simulink model "kinovaMicoSimscapeModel"  (R2021b)
(part 41 of 50)

Y5_10_1=(111*dq4*dqr1*sin(q2)*sin(q3)*sin(q6))/4000 - (37*dq6*dqr1*sin(q2)*sin(q3)*sin(q6))/4000 - (111*dq4*dqr1*cos(q5)^2*sin(q2)*sin(q3)*sin(q6))/2000 - (111*dq6*dqr1*cos(q5)*sin(q2)*sin(q3)*sin(q6))/4000 - (37*dq2*dqr1*cos(q3)*cos(q4)^2*cos(q6)*sin(q2))/2000 + (37*dq3*dqr1*cos(q3)*cos(q4)^2*cos(q6)*sin(q2))/2000 + (37*3^(1/2)*dq1*dqr1*cos(q2)*sin(q2)*sin(q4)*sin(q6))/2000 - (37*3^(1/2)*dq2*dqr1*cos(q4)*sin(q2)*sin(q3)*sin(q6))/4000 + (37*3^(1/2)*dq3*dqr1*cos(q4)*sin(q2)*sin(q3)*sin(q6))/4000 - (37*3^(1/2)*dq4*dqr1*cos(q3)*sin(q2)*sin(q4)*sin(q6))/4000 - (37*3^(1/2)*dq6*dqr1*cos(q3)*sin(q2)*sin(q4)*sin(q6))/4000 + (37*dq2*dqr1*cos(q3)*cos(q4)^2*cos(q5)^2*cos(q6)*sin(q2))/1000 - (37*dq3*dqr1*cos(q3)*cos(q4)^2*cos(q5)^2*cos(q6)*sin(q2))/1000 + (37*dq1*dqr1*cos(q2)*cos(q3)*sin(q2)*sin(q3)*sin(q6))/1000 - (877*dq1*dqr1*cos(q2)*cos(q4)*sin(q2)*sin(q5)*sin(q6))/4000 - (1231*dq1*dqr1*cos(q2)*cos(q6)*sin(q2)*sin(q4)*sin(q5))/40000 + (37*dq2*dqr1*cos(q3)*cos(q4)*sin(q2)*sin(q4)*sin(q6))/800 + (877*dq2*dqr1*cos(q4)*cos(q5)*sin(q2)*sin(q3)*sin(q6))/8000 - (37*dq3*dqr1*cos(q3)*cos(q4)*sin(q2)*sin(q4)*sin(q6))/800 + (37*dq2*dqr1*cos(q3)*cos(q5)*sin(q2)*sin(q5)*sin(q6))/1000 - (877*dq3*dqr1*cos(q4)*cos(q5)*sin(q2)*sin(q3)*sin(q6))/8000 - (37*dq3*dqr1*cos(q3)*cos(q5)*sin(q2)*sin(q5)*sin(q6))/1000 - (111*dq4*dqr1*cos(q5)*cos(q6)*sin(q2)*sin(q3)*sin(q5))/4000 - (877*dq2*dqr1*sin(q2)*sin(q3)*sin(q4)*sin(q5)*sin(q6))/4000 + (877*dq3*dqr1*sin(q2)*sin(q3)*sin(q4)*sin(q5)*sin(q6))/4000 - dq2*dqr1*cos(q3)*sin(q2)*sin(q5)*sin(q6)*((641*3^(1/2))/20000 + 37/1000) + dq3*dqr1*cos(q3)*sin(q2)*sin(q5)*sin(q6)*((641*3^(1/2))/20000 + 37/1000) - dq4*dqr1*cos(q5)*sin(q2)*sin(q3)*sin(q6)*((641*3^(1/2))/40000 + 37/2000) - dq4*dqr1*cos(q6)*sin(q2)*sin(q3)*sin(q5)*((641*3^(1/2))/80000 - 37/8000) - (37*3^(1/2)*dq1*dqr1*cos(q2)*cos(q4)*cos(q6)*sin(q2))/2000 + (37*3^(1/2)*dq1*dqr1*cos(q2)*cos(q3)^2*cos(q4)*cos(q6)*sin(q2))/1000 + (37*3^(1/2)*dq1*dqr1*cos(q2)*cos(q4)*cos(q5)^2*cos(q6)*sin(q2))/1000 - (37*3^(1/2)*dq4*dqr1*cos(q3)*cos(q4)*cos(q5)^2*cos(q6)*sin(q2))/2000 + (29*dq1*dqr1*cos(q2)*cos(q3)*cos(q4)*cos(q5)*cos(q6)*sin(q2))/200 - (37*3^(1/2)*dq1*dqr1*cos(q2)*cos(q3)^2*sin(q2)*sin(q4)*sin(q6))/1000 - (37*3^(1/2)*dq1*dqr1*cos(q2)*cos(q5)^2*sin(q2)*sin(q4)*sin(q6))/1000 + (37*3^(1/2)*dq2*dqr1*cos(q4)*cos(q5)^2*sin(q2)*sin(q3)*sin(q6))/2000 + (37*3^(1/2)*dq2*dqr1*cos(q5)^2*cos(q6)*sin(q2)*sin(q3)*sin(q4))/2000 - (37*3^(1/2)*dq3*dqr1*cos(q4)*cos(q5)^2*sin(q2)*sin(q3)*sin(q6))/2000 - (37*3^(1/2)*dq3*dqr1*cos(q5)^2*cos(q6)*sin(q2)*sin(q3)*sin(q4))/2000 + (37*3^(1/2)*dq4*dqr1*cos(q3)*cos(q5)^2*sin(q2)*sin(q4)*sin(q6))/2000 - (29*dq1*dqr1*cos(q2)*cos(q3)*cos(q4)*sin(q2)*sin(q5)*sin(q6))/100 - (29*dq1*dqr1*cos(q2)*cos(q3)*cos(q5)*sin(q2)*sin(q4)*sin(q6))/200 - (29*dq1*dqr1*cos(q2)*cos(q3)*cos(q6)*sin(q2)*sin(q4)*sin(q5))/400 - dq1*dqr1*cos(q2)*cos(q4)*cos(q5)*cos(q6)*sin(q2)*((37*3^(1/2))/4000 - 877/8000) - dq2*dqr1*cos(q5)*cos(q6)*sin(q2)*sin(q3)*sin(q4)*((37*3^(1/2))/4000 - 877/8000) + dq3*dqr1*cos(q5)*cos(q6)*sin(q2)*sin(q3)*sin(q4)*((37*3^(1/2))/4000 - 877/8000) + dq1*dqr1*cos(q2)*cos(q5)*sin(q2)*sin(q4)*sin(q6)*((37*3^(1/2))/2000 - 1231/20000) - dq2*dqr1*cos(q4)*cos(q6)*sin(q2)*sin(q3)*sin(q5)*((37*3^(1/2))/8000 - 877/16000) + dq3*dqr1*cos(q4)*cos(q6)*sin(q2)*sin(q3)*sin(q5)*((37*3^(1/2))/8000 - 877/16000) - dq4*dqr1*cos(q3)*cos(q5)*sin(q2)*sin(q4)*sin(q6)*((37*3^(1/2))/2000 + 1923/40000) + dq4*dqr1*cos(q3)*cos(q6)*sin(q2)*sin(q4)*sin(q5)*((37*3^(1/2))/8000 - 1923/80000) + (37*dq1*dqr1*cos(q2)*cos(q3)*cos(q4)^2*sin(q2)*sin(q3)*sin(q6))/400 - (37*dq1*dqr1*cos(q2)*cos(q3)*cos(q5)^2*sin(q2)*sin(q3)*sin(q6))/500 + (877*dq1*dqr1*cos(q2)*cos(q3)^2*cos(q4)*sin(q2)*sin(q5)*sin(q6))/2000 + (1231*dq1*dqr1*cos(q2)*cos(q3)^2*cos(q6)*sin(q2)*sin(q4)*sin(q5))/20000 - (37*dq2*dqr1*cos(q3)*cos(q4)*cos(q5)^2*sin(q2)*sin(q4)*sin(q6))/400 - (37*dq2*dqr1*cos(q3)*cos(q4)^2*cos(q5)*sin(q2)*sin(q5)*sin(q6))/500 + (37*dq3*dqr1*cos(q3)*cos(q4)*cos(q5)^2*sin(q2)*sin(q4)*sin(q6))/400 + (37*dq3*dqr1*cos(q3)*cos(q4)^2*cos(q5)*sin(q2)*sin(q5)*sin(q6))/500 - dq2*dqr1*cos(q3)*cos(q4)^2*cos(q5)*cos(q6)*sin(q2)*((641*3^(1/2))/40000 - 37/4000) + dq3*dqr1*cos(q3)*cos(q4)^2*cos(q5)*cos(q6)*sin(q2)*((641*3^(1/2))/40000 - 37/4000) + (29*3^(1/2)*dq1*dqr1*cos(q2)*cos(q5)*sin(q2)*sin(q3)*sin(q6))/200 + (29*3^(1/2)*dq1*dqr1*cos(q2)*cos(q6)*sin(q2)*sin(q3)*sin(q5))/400 + (37*3^(1/2)*dq6*dqr1*cos(q3)*cos(q4)*sin(q2)*sin(q5)*sin(q6))/2000 + (37*3^(1/2)*dq6*dqr1*cos(q3)*cos(q5)*sin(q2)*sin(q4)*sin(q6))/4000 + dq2*dqr1*cos(q3)*cos(q4)^2*sin(q2)*sin(q5)*sin(q6)*((641*3^(1/2))/20000 + 37/1000) - dq3*dqr1*cos(q3)*cos(q4)^2*sin(q2)*sin(q5)*sin(q6)*((641*3^(1/2))/20000 + 37/1000) + (37*dq1*dqr1*cos(q2)*cos(q3)*cos(q4)*cos(q6)*sin(q2)*sin(q3)*sin(q4))/1000 - (37*dq1*dqr1*cos(q2)*cos(q3)*cos(q5)*cos(q6)*sin(q2)*sin(q3)*sin(q5))/1000 - (37*dq2*dqr1*cos(q3)*cos(q4)*cos(q5)*cos(q6)*sin(q2)*sin(q4)*sin(q5))/800 + (37*dq3*dqr1*cos(q3)*cos(q4)*cos(q5)*cos(q6)*sin(q2)*sin(q4)*sin(q5))/800 - (37*3^(1/2)*dq1*dqr1*cos(q2)*cos(q3)^2*cos(q4)*cos(q5)^2*cos(q6)*sin(q2))/500 - dq1*dqr1*cos(q2)*cos(q3)*cos(q5)*sin(q2)*sin(q3)*sin(q6)*((2513*3^(1/2))/10000 + 37/1000) - dq1*dqr1*cos(q2)*cos(q3)*cos(q6)*sin(q2)*sin(q3)*sin(q5)*((2513*3^(1/2))/20000 - 37/1000) + dq2*dqr1*cos(q3)*cos(q4)*cos(q5)*sin(q2)*sin(q4)*sin(q6)*((641*3^(1/2))/40000 + 37/2000) - dq3*dqr1*cos(q3)*cos(q4)*cos(q5)*sin(q2)*sin(q4)*sin(q6)*((641*3^(1/2))/40000 + 37/2000) + dq2*dqr1*cos(q3)*cos(q4)*cos(q6)*sin(q2)*sin(q4)*sin(q5)*((641*3^(1/2))/80000 - 37/8000) - dq3*dqr1*cos(q3)*cos(q4)*cos(q6)*sin(q2)*sin(q4)*sin(q5)*((641*3^(1/2))/80000 - 37/8000) + (37*3^(1/2)*dq1*dqr1*cos(q2)*cos(q3)^2*cos(q5)^2*sin(q2)*sin(q4)*sin(q6))/500 + dq1*dqr1*cos(q2)*cos(q3)^2*cos(q4)*cos(q5)*cos(q6)*sin(q2)*((37*3^(1/2))/2000 - 877/4000) - (37*3^(1/2)*dq1*dqr1*cos(q2)*cos(q4)*cos(q5)*sin(q2)*sin(q5)*sin(q6))/500 - (37*3^(1/2)*dq1*dqr1*cos(q2)*cos(q5)*cos(q6)*sin(q2)*sin(q4)*sin(q5))/2000 + (37*3^(1/2)*dq2*dqr1*cos(q4)*cos(q5)*cos(q6)*sin(q2)*sin(q3)*sin(q5))/4000 - (37*3^(1/2)*dq3*dqr1*cos(q4)*cos(q5)*cos(q6)*sin(q2)*sin(q3)*sin(q5))/4000 + (37*3^(1/2)*dq4*dqr1*cos(q3)*cos(q4)*cos(q5)*sin(q2)*sin(q5)*sin(q6))/1000 + (37*3^(1/2)*dq4*dqr1*cos(q3)*cos(q5)*cos(q6)*sin(q2)*sin(q4)*sin(q5))/4000 - dq1*dqr1*cos(q2)*cos(q3)^2*cos(q5)*sin(q2)*sin(q4)*sin(q6)*((37*3^(1/2))/1000 - 1231/10000) - (37*3^(1/2)*dq2*dqr1*cos(q5)*sin(q2)*sin(q3)*sin(q4)*sin(q5)*sin(q6))/1000 + (37*3^(1/2)*dq3*dqr1*cos(q5)*sin(q2)*sin(q3)*sin(q4)*sin(q5)*sin(q6))/1000 - (37*dq1*dqr1*cos(q2)*cos(q3)*cos(q4)^2*cos(q5)^2*sin(q2)*sin(q3)*sin(q6))/200 - (37*dq1*dqr1*cos(q2)*cos(q3)*cos(q4)*cos(q5)^2*cos(q6)*sin(q2)*sin(q3)*sin(q4))/500 - (37*dq1*dqr1*cos(q2)*cos(q3)*cos(q4)^2*cos(q5)*cos(q6)*sin(q2)*sin(q3)*sin(q5))/400 + dq1*dqr1*cos(q2)*cos(q3)*cos(q4)^2*cos(q5)*sin(q2)*sin(q3)*sin(q6)*((641*3^(1/2))/20000 + 37/1000) + dq1*dqr1*cos(q2)*cos(q3)*cos(q4)^2*cos(q6)*sin(q2)*sin(q3)*sin(q5)*((641*3^(1/2))/40000 - 37/4000) + (37*3^(1/2)*dq1*dqr1*cos(q2)*cos(q3)^2*cos(q4)*cos(q5)*sin(q2)*sin(q5)*sin(q6))/250 + (37*3^(1/2)*dq1*dqr1*cos(q2)*cos(q3)^2*cos(q5)*cos(q6)*sin(q2)*sin(q4)*sin(q5))/1000 + dq1*dqr1*cos(q2)*cos(q3)*cos(q4)*cos(q5)*cos(q6)*sin(q2)*sin(q3)*sin(q4)*((641*3^(1/2))/20000 - 37/2000) - dq1*dqr1*cos(q2)*cos(q3)*cos(q4)*sin(q2)*sin(q3)*sin(q4)*sin(q5)*sin(q6)*((641*3^(1/2))/10000 + 37/500) + (37*dq1*dqr1*cos(q2)*cos(q3)*cos(q4)*cos(q5)*sin(q2)*sin(q3)*sin(q4)*sin(q5)*sin(q6))/250;
Y5_10_2=(7*dq1*dqr1*cos(q5)*cos(q6)*sin(q4))/2000 - (7*dq1*dqr1*sin(q4)*sin(q5)*sin(q6))/1000 + (29*dq1*dqr1*cos(q4)*cos(q5)*cos(q6)*sin(q3))/200 - (29*dq2*dqr1*cos(q2)*cos(q5)*cos(q6)*sin(q4))/200 - (29*dq1*dqr1*cos(q4)*sin(q3)*sin(q5)*sin(q6))/100 - (29*dq1*dqr1*cos(q5)*sin(q3)*sin(q4)*sin(q6))/200 - (29*dq1*dqr1*cos(q6)*sin(q3)*sin(q4)*sin(q5))/400 + (29*dq2*dqr1*cos(q2)*sin(q4)*sin(q5)*sin(q6))/100 - (37*dq1*dqr1*cos(q2)^2*cos(q4)*cos(q6)*sin(q4))/2000 + (37*dq2*dqr1*cos(q2)*cos(q4)^2*cos(q6)*sin(q3))/2000 - (37*dq1*dqr1*cos(q3)^2*cos(q4)*cos(q6)*sin(q4))/2000 + (37*dq2*dqr1*cos(q2)*cos(q5)^2*cos(q6)*sin(q3))/2000 - (37*dq2*dqr1*cos(q3)*cos(q5)^2*cos(q6)*sin(q2))/2000 - (37*dq3*dqr1*cos(q2)*cos(q4)^2*cos(q6)*sin(q3))/2000 - (37*dq3*dqr1*cos(q2)*cos(q5)^2*cos(q6)*sin(q3))/2000 + (37*dq3*dqr1*cos(q3)*cos(q5)^2*cos(q6)*sin(q2))/2000 - (37*3^(1/2)*dq1*dqr1*cos(q3)*sin(q3)*sin(q4)*sin(q6))/2000 + (37*3^(1/2)*dq4*dqr1*cos(q2)*sin(q3)*sin(q4)*sin(q6))/4000 + (37*3^(1/2)*dq6*dqr1*cos(q2)*sin(q3)*sin(q4)*sin(q6))/4000 + (37*dq1*dqr1*cos(q2)^2*cos(q3)^2*cos(q4)*cos(q6)*sin(q4))/1000 + (37*dq1*dqr1*cos(q2)^2*cos(q4)*cos(q5)^2*cos(q6)*sin(q4))/1000 - (37*dq2*dqr1*cos(q2)*cos(q4)^2*cos(q5)^2*cos(q6)*sin(q3))/1000 + (37*dq1*dqr1*cos(q3)^2*cos(q4)*cos(q5)^2*cos(q6)*sin(q4))/1000 + (37*dq3*dqr1*cos(q2)*cos(q4)^2*cos(q5)^2*cos(q6)*sin(q3))/1000 - (37*dq2*dqr1*cos(q2)*cos(q4)*sin(q3)*sin(q4)*sin(q6))/800 + (877*dq1*dqr1*cos(q3)*cos(q4)*sin(q3)*sin(q5)*sin(q6))/4000 + (1231*dq1*dqr1*cos(q3)*cos(q6)*sin(q3)*sin(q4)*sin(q5))/40000 - (877*dq2*dqr1*cos(q2)*cos(q3)*sin(q4)*sin(q5)*sin(q6))/4000 + (37*dq3*dqr1*cos(q2)*cos(q4)*sin(q3)*sin(q4)*sin(q6))/800 - (37*dq2*dqr1*cos(q2)*cos(q5)*sin(q3)*sin(q5)*sin(q6))/1000 + (877*dq3*dqr1*cos(q2)*cos(q3)*sin(q4)*sin(q5)*sin(q6))/4000 + (37*dq3*dqr1*cos(q2)*cos(q5)*sin(q3)*sin(q5)*sin(q6))/1000 - dq2*dqr1*cos(q2)*cos(q5)*cos(q6)*sin(q3)*((641*3^(1/2))/40000 - 37/4000) + dq2*dqr1*cos(q3)*cos(q5)*cos(q6)*sin(q2)*((641*3^(1/2))/40000 - 37/4000) + dq3*dqr1*cos(q2)*cos(q5)*cos(q6)*sin(q3)*((641*3^(1/2))/40000 - 37/4000) - dq3*dqr1*cos(q3)*cos(q5)*cos(q6)*sin(q2)*((641*3^(1/2))/40000 - 37/4000) - (29*dq1*dqr1*cos(q2)^2*cos(q4)*cos(q5)*cos(q6)*sin(q3))/200 + dq2*dqr1*cos(q2)*sin(q3)*sin(q5)*sin(q6)*((641*3^(1/2))/20000 + 37/1000) - dq3*dqr1*cos(q2)*sin(q3)*sin(q5)*sin(q6)*((641*3^(1/2))/20000 + 37/1000) + (29*dq1*dqr1*cos(q2)^2*cos(q4)*sin(q3)*sin(q5)*sin(q6))/100 + (29*dq1*dqr1*cos(q2)^2*cos(q5)*sin(q3)*sin(q4)*sin(q6))/200 + (29*dq1*dqr1*cos(q2)^2*cos(q6)*sin(q3)*sin(q4)*sin(q5))/400 + (37*3^(1/2)*dq1*dqr1*cos(q3)*cos(q4)*cos(q6)*sin(q3))/2000 - (37*3^(1/2)*dq4*dqr1*cos(q2)*cos(q4)*cos(q6)*sin(q3))/2000 + (37*3^(1/2)*dq4*dqr1*cos(q3)*cos(q4)*cos(q6)*sin(q2))/2000 - (37*3^(1/2)*dq1*dqr1*cos(q2)^2*cos(q3)*cos(q4)*cos(q6)*sin(q3))/1000 - (37*3^(1/2)*dq1*dqr1*cos(q3)*cos(q4)*cos(q5)^2*cos(q6)*sin(q3))/1000 + (37*3^(1/2)*dq2*dqr1*cos(q2)*cos(q3)*cos(q5)^2*cos(q6)*sin(q4))/2000 - (37*3^(1/2)*dq3*dqr1*cos(q2)*cos(q3)*cos(q5)^2*cos(q6)*sin(q4))/2000 + (37*3^(1/2)*dq4*dqr1*cos(q2)*cos(q4)*cos(q5)^2*cos(q6)*sin(q3))/2000 + (37*3^(1/2)*dq1*dqr1*cos(q2)^2*cos(q3)*sin(q3)*sin(q4)*sin(q6))/1000 + (37*3^(1/2)*dq1*dqr1*cos(q3)*cos(q5)^2*sin(q3)*sin(q4)*sin(q6))/1000 - (37*3^(1/2)*dq4*dqr1*cos(q2)*cos(q5)^2*sin(q3)*sin(q4)*sin(q6))/2000 - (37*dq1*dqr1*cos(q2)^2*cos(q3)^2*cos(q4)*cos(q5)^2*cos(q6)*sin(q4))/500 - (37*dq1*dqr1*cos(q2)^2*cos(q3)^2*cos(q4)^2*cos(q5)*cos(q6)*sin(q5))/400 + dq1*dqr1*cos(q3)*cos(q4)*cos(q5)*cos(q6)*sin(q3)*((37*3^(1/2))/4000 - 877/8000) - dq2*dqr1*cos(q2)*cos(q3)*cos(q5)*cos(q6)*sin(q4)*((37*3^(1/2))/4000 - 877/8000) + dq3*dqr1*cos(q2)*cos(q3)*cos(q5)*cos(q6)*sin(q4)*((37*3^(1/2))/4000 - 877/8000) - dq1*dqr1*cos(q3)*cos(q5)*sin(q3)*sin(q4)*sin(q6)*((37*3^(1/2))/2000 - 1231/20000) + dq4*dqr1*cos(q2)*cos(q5)*sin(q3)*sin(q4)*sin(q6)*((37*3^(1/2))/2000 + 1923/40000) - dq4*dqr1*cos(q2)*cos(q6)*sin(q3)*sin(q4)*sin(q5)*((37*3^(1/2))/8000 - 1923/80000) - (877*dq1*dqr1*cos(q2)^2*cos(q3)*cos(q4)*sin(q3)*sin(q5)*sin(q6))/2000 - (1231*dq1*dqr1*cos(q2)^2*cos(q3)*cos(q6)*sin(q3)*sin(q4)*sin(q5))/20000 + (37*dq2*dqr1*cos(q2)*cos(q4)*cos(q5)^2*sin(q3)*sin(q4)*sin(q6))/400 - (37*dq1*dqr1*cos(q2)^2*cos(q4)*cos(q5)*sin(q4)*sin(q5)*sin(q6))/500 + (37*dq2*dqr1*cos(q2)*cos(q4)^2*cos(q5)*sin(q3)*sin(q5)*sin(q6))/500 - (37*dq3*dqr1*cos(q2)*cos(q4)*cos(q5)^2*sin(q3)*sin(q4)*sin(q6))/400 - (37*dq1*dqr1*cos(q3)^2*cos(q4)*cos(q5)*sin(q4)*sin(q5)*sin(q6))/500 - (37*dq3*dqr1*cos(q2)*cos(q4)^2*cos(q5)*sin(q3)*sin(q5)*sin(q6))/500 - dq1*dqr1*cos(q2)^2*cos(q4)*cos(q5)*cos(q6)*sin(q4)*((641*3^(1/2))/40000 - 37/4000) + dq2*dqr1*cos(q2)*cos(q4)^2*cos(q5)*cos(q6)*sin(q3)*((641*3^(1/2))/40000 - 37/4000) - dq1*dqr1*cos(q3)^2*cos(q4)*cos(q5)*cos(q6)*sin(q4)*((641*3^(1/2))/40000 - 37/4000) - dq3*dqr1*cos(q2)*cos(q4)^2*cos(q5)*cos(q6)*sin(q3)*((641*3^(1/2))/40000 - 37/4000) - (37*3^(1/2)*dq6*dqr1*cos(q2)*cos(q4)*sin(q3)*sin(q5)*sin(q6))/2000 - (37*3^(1/2)*dq6*dqr1*cos(q2)*cos(q5)*sin(q3)*sin(q4)*sin(q6))/4000 + dq1*dqr1*cos(q2)^2*cos(q4)*sin(q4)*sin(q5)*sin(q6)*((641*3^(1/2))/20000 + 37/1000) - dq2*dqr1*cos(q2)*cos(q4)^2*sin(q3)*sin(q5)*sin(q6)*((641*3^(1/2))/20000 + 37/1000) + dq1*dqr1*cos(q3)^2*cos(q4)*sin(q4)*sin(q5)*sin(q6)*((641*3^(1/2))/20000 + 37/1000) + dq3*dqr1*cos(q2)*cos(q4)^2*sin(q3)*sin(q5)*sin(q6)*((641*3^(1/2))/20000 + 37/1000) + dq1*dqr1*cos(q2)^2*cos(q3)^2*cos(q4)*cos(q5)*cos(q6)*sin(q4)*((641*3^(1/2))/20000 - 37/2000) + (37*dq2*dqr1*cos(q2)*cos(q4)*cos(q5)*cos(q6)*sin(q3)*sin(q4)*sin(q5))/800 - (37*dq3*dqr1*cos(q2)*cos(q4)*cos(q5)*cos(q6)*sin(q3)*sin(q4)*sin(q5))/800 - dq1*dqr1*cos(q2)^2*cos(q3)^2*cos(q4)*sin(q4)*sin(q5)*sin(q6)*((641*3^(1/2))/10000 + 37/500) + (37*3^(1/2)*dq1*dqr1*cos(q2)^2*cos(q3)*cos(q4)*cos(q5)^2*cos(q6)*sin(q3))/500 - dq2*dqr1*cos(q2)*cos(q4)*cos(q5)*sin(q3)*sin(q4)*sin(q6)*((641*3^(1/2))/40000 + 37/2000) + dq3*dqr1*cos(q2)*cos(q4)*cos(q5)*sin(q3)*sin(q4)*sin(q6)*((641*3^(1/2))/40000 + 37/2000) - dq2*dqr1*cos(q2)*cos(q4)*cos(q6)*sin(q3)*sin(q4)*sin(q5)*((641*3^(1/2))/80000 - 37/8000) + dq3*dqr1*cos(q2)*cos(q4)*cos(q6)*sin(q3)*sin(q4)*sin(q5)*((641*3^(1/2))/80000 - 37/8000) - (37*3^(1/2)*dq1*dqr1*cos(q2)^2*cos(q3)*cos(q5)^2*sin(q3)*sin(q4)*sin(q6))/500 - dq1*dqr1*cos(q2)^2*cos(q3)*cos(q4)*cos(q5)*cos(q6)*sin(q3)*((37*3^(1/2))/2000 - 877/4000) + (37*3^(1/2)*dq1*dqr1*cos(q3)*cos(q4)*cos(q5)*sin(q3)*sin(q5)*sin(q6))/500 + (37*3^(1/2)*dq1*dqr1*cos(q3)*cos(q5)*cos(q6)*sin(q3)*sin(q4)*sin(q5))/2000 - (37*3^(1/2)*dq2*dqr1*cos(q2)*cos(q3)*cos(q5)*sin(q4)*sin(q5)*sin(q6))/1000 + (37*3^(1/2)*dq3*dqr1*cos(q2)*cos(q3)*cos(q5)*sin(q4)*sin(q5)*sin(q6))/1000 - (37*3^(1/2)*dq4*dqr1*cos(q2)*cos(q4)*cos(q5)*sin(q3)*sin(q5)*sin(q6))/1000 - (37*3^(1/2)*dq4*dqr1*cos(q2)*cos(q5)*cos(q6)*sin(q3)*sin(q4)*sin(q5))/4000 + dq1*dqr1*cos(q2)^2*cos(q3)*cos(q5)*sin(q3)*sin(q4)*sin(q6)*((37*3^(1/2))/1000 - 1231/10000) + (37*dq1*dqr1*cos(q2)^2*cos(q3)^2*cos(q4)*cos(q5)*sin(q4)*sin(q5)*sin(q6))/250 - (37*3^(1/2)*dq1*dqr1*cos(q2)^2*cos(q3)*cos(q4)*cos(q5)*sin(q3)*sin(q5)*sin(q6))/250 - (37*3^(1/2)*dq1*dqr1*cos(q2)^2*cos(q3)*cos(q5)*cos(q6)*sin(q3)*sin(q4)*sin(q5))/1000;
Y5_10_3=(111*dq1*dqr1*sin(q6))/4000 - (37*dq1*dqr1*cos(q2)^2*sin(q6))/2000 - (37*dq1*dqr1*cos(q3)^2*sin(q6))/2000 - (111*dq1*dqr1*cos(q5)^2*sin(q6))/2000 + (37*dq1*dqr1*cos(q2)^2*cos(q3)^2*sin(q6))/1000 - (37*dq1*dqr1*cos(q2)^2*cos(q4)^2*sin(q6))/800 + (37*dq1*dqr1*cos(q2)^2*cos(q5)^2*sin(q6))/1000 - (37*dq1*dqr1*cos(q3)^2*cos(q4)^2*sin(q6))/800 + (37*dq1*dqr1*cos(q3)^2*cos(q5)^2*sin(q6))/1000 + (111*dq4*dqr1*cos(q2)*cos(q3)*sin(q6))/4000 + (7*dq1*dqr1*cos(q4)*cos(q5)*sin(q6))/2000 + (7*dq1*dqr1*cos(q4)*cos(q6)*sin(q5))/4000 - (111*dq1*dqr1*cos(q5)*cos(q6)*sin(q5))/4000 - (37*dq6*dqr1*cos(q2)*cos(q3)*sin(q6))/4000 - dq1*dqr1*cos(q5)*sin(q6)*((641*3^(1/2))/40000 + 37/2000) - dq1*dqr1*cos(q6)*sin(q5)*((641*3^(1/2))/80000 - 37/8000) - (29*3^(1/2)*dq1*dqr1*cos(q3)*cos(q5)*sin(q6))/200 - (29*3^(1/2)*dq1*dqr1*cos(q3)*cos(q6)*sin(q5))/400 + dq1*dqr1*cos(q2)^2*cos(q5)*sin(q6)*((2513*3^(1/2))/20000 + 37/2000) + dq1*dqr1*cos(q3)^2*cos(q5)*sin(q6)*((2513*3^(1/2))/20000 + 37/2000) + dq1*dqr1*cos(q2)^2*cos(q6)*sin(q5)*((2513*3^(1/2))/40000 - 37/2000) + dq1*dqr1*cos(q3)^2*cos(q6)*sin(q5)*((2513*3^(1/2))/40000 - 37/2000) - (29*dq2*dqr1*cos(q2)*cos(q4)*cos(q5)*sin(q6))/200 - (29*dq2*dqr1*cos(q2)*cos(q4)*cos(q6)*sin(q5))/400 + (29*dq2*dqr2*cos(q4)*cos(q5)*cos(q6)*sin(q3))/200 - (111*dq6*dqr1*cos(q2)*cos(q3)*cos(q5)*sin(q6))/4000 + (37*dq1*dqr1*cos(q2)^2*cos(q3)^2*cos(q4)^2*sin(q6))/400 - (37*dq1*dqr1*cos(q2)^2*cos(q3)^2*cos(q5)^2*sin(q6))/500 + (37*dq1*dqr1*cos(q2)^2*cos(q4)^2*cos(q5)^2*sin(q6))/400 + (37*dq1*dqr1*cos(q3)^2*cos(q4)^2*cos(q5)^2*sin(q6))/400 - (29*dq2*dqr2*cos(q4)*sin(q3)*sin(q5)*sin(q6))/100 - (29*dq2*dqr2*cos(q5)*sin(q3)*sin(q4)*sin(q6))/200 - (29*dq2*dqr2*cos(q6)*sin(q3)*sin(q4)*sin(q5))/400 + (37*dq1*dqr2*cos(q2)*cos(q4)^2*cos(q6)*sin(q3))/2000 - (37*dq1*dqr2*cos(q3)*cos(q4)^2*cos(q6)*sin(q2))/2000 + (37*dq1*dqr2*cos(q2)*cos(q5)^2*cos(q6)*sin(q3))/2000 - (37*dq1*dqr2*cos(q3)*cos(q5)^2*cos(q6)*sin(q2))/2000 + (37*dq1*dqr1*cos(q2)^2*cos(q5)*cos(q6)*sin(q5))/2000 + (37*dq1*dqr1*cos(q3)^2*cos(q5)*cos(q6)*sin(q5))/2000 - (111*dq4*dqr1*cos(q2)*cos(q3)*cos(q5)^2*sin(q6))/2000 - (37*3^(1/2)*dq1*dqr2*cos(q4)*sin(q2)*sin(q3)*sin(q6))/4000 - (37*dq1*dqr1*cos(q2)^2*cos(q3)^2*cos(q5)*cos(q6)*sin(q5))/1000 - (37*dq1*dqr2*cos(q2)*cos(q4)^2*cos(q5)^2*cos(q6)*sin(q3))/1000 + (37*dq1*dqr2*cos(q3)*cos(q4)^2*cos(q5)^2*cos(q6)*sin(q2))/1000 + (37*dq1*dqr1*cos(q2)^2*cos(q4)^2*cos(q5)*cos(q6)*sin(q5))/800 + (37*dq1*dqr1*cos(q3)^2*cos(q4)^2*cos(q5)*cos(q6)*sin(q5))/800 + (29*3^(1/2)*dq1*dqr1*cos(q2)^2*cos(q3)*cos(q5)*sin(q6))/200 + (29*3^(1/2)*dq1*dqr1*cos(q2)^2*cos(q3)*cos(q6)*sin(q5))/400 + (877*dq2*dqr1*cos(q2)*cos(q3)*cos(q4)*cos(q5)*sin(q6))/8000 - (877*dq3*dqr1*cos(q2)*cos(q3)*cos(q4)*cos(q5)*sin(q6))/8000 - (111*dq4*dqr1*cos(q2)*cos(q3)*cos(q5)*cos(q6)*sin(q5))/4000 - dq1*dqr1*cos(q2)^2*cos(q3)^2*cos(q5)*sin(q6)*((2513*3^(1/2))/10000 + 37/1000) - dq1*dqr1*cos(q2)^2*cos(q3)^2*cos(q6)*sin(q5)*((2513*3^(1/2))/20000 - 37/1000) - dq1*dqr1*cos(q2)^2*cos(q4)^2*cos(q5)*sin(q6)*((641*3^(1/2))/40000 + 37/2000) - dq1*dqr1*cos(q3)^2*cos(q4)^2*cos(q5)*sin(q6)*((641*3^(1/2))/40000 + 37/2000) - dq1*dqr1*cos(q2)^2*cos(q4)^2*cos(q6)*sin(q5)*((641*3^(1/2))/80000 - 37/8000) - dq1*dqr1*cos(q3)^2*cos(q4)^2*cos(q6)*sin(q5)*((641*3^(1/2))/80000 - 37/8000) - (37*dq1*dqr2*cos(q2)*cos(q4)*sin(q3)*sin(q4)*sin(q6))/800 + (37*dq1*dqr2*cos(q3)*cos(q4)*sin(q2)*sin(q4)*sin(q6))/800 + (877*dq1*dqr2*cos(q4)*cos(q5)*sin(q2)*sin(q3)*sin(q6))/8000 - (37*dq1*dqr2*cos(q2)*cos(q5)*sin(q3)*sin(q5)*sin(q6))/1000 + (37*dq1*dqr2*cos(q3)*cos(q5)*sin(q2)*sin(q5)*sin(q6))/1000 - (877*dq1*dqr2*sin(q2)*sin(q3)*sin(q4)*sin(q5)*sin(q6))/4000 - dq4*dqr1*cos(q2)*cos(q3)*cos(q5)*sin(q6)*((641*3^(1/2))/40000 + 37/2000) - dq1*dqr2*cos(q2)*cos(q5)*cos(q6)*sin(q3)*((641*3^(1/2))/40000 - 37/4000) + dq1*dqr2*cos(q3)*cos(q5)*cos(q6)*sin(q2)*((641*3^(1/2))/40000 - 37/4000) - dq4*dqr1*cos(q2)*cos(q3)*cos(q6)*sin(q5)*((641*3^(1/2))/80000 - 37/8000) + dq1*dqr2*cos(q2)*sin(q3)*sin(q5)*sin(q6)*((641*3^(1/2))/20000 + 37/1000) - dq1*dqr2*cos(q3)*sin(q2)*sin(q5)*sin(q6)*((641*3^(1/2))/20000 + 37/1000) - (37*dq1*dqr1*cos(q2)^2*cos(q3)^2*cos(q4)^2*cos(q5)^2*sin(q6))/200 - (37*3^(1/2)*dq2*dqr1*cos(q2)*cos(q3)*cos(q4)*sin(q6))/4000 + (37*3^(1/2)*dq3*dqr1*cos(q2)*cos(q3)*cos(q4)*sin(q6))/4000 + (37*3^(1/2)*dq2*dqr1*cos(q2)*cos(q3)*cos(q4)*cos(q5)^2*sin(q6))/2000 - (37*3^(1/2)*dq3*dqr1*cos(q2)*cos(q3)*cos(q4)*cos(q5)^2*sin(q6))/2000 + (37*3^(1/2)*dq1*dqr2*cos(q4)*cos(q5)^2*sin(q2)*sin(q3)*sin(q6))/2000 + (37*3^(1/2)*dq1*dqr2*cos(q5)^2*cos(q6)*sin(q2)*sin(q3)*sin(q4))/2000 - dq2*dqr1*cos(q2)*cos(q3)*cos(q4)*cos(q6)*sin(q5)*((37*3^(1/2))/8000 - 877/16000) + dq3*dqr1*cos(q2)*cos(q3)*cos(q4)*cos(q6)*sin(q5)*((37*3^(1/2))/8000 - 877/16000) + dq1*dqr1*cos(q2)^2*cos(q3)^2*cos(q4)^2*cos(q5)*sin(q6)*((641*3^(1/2))/20000 + 37/1000) + dq1*dqr1*cos(q2)^2*cos(q3)^2*cos(q4)^2*cos(q6)*sin(q5)*((641*3^(1/2))/40000 - 37/4000) - dq1*dqr2*cos(q5)*cos(q6)*sin(q2)*sin(q3)*sin(q4)*((37*3^(1/2))/4000 - 877/8000) - dq1*dqr2*cos(q4)*cos(q6)*sin(q2)*sin(q3)*sin(q5)*((37*3^(1/2))/8000 - 877/16000) + (37*dq1*dqr2*cos(q2)*cos(q4)*cos(q5)^2*sin(q3)*sin(q4)*sin(q6))/400 - (37*dq1*dqr2*cos(q3)*cos(q4)*cos(q5)^2*sin(q2)*sin(q4)*sin(q6))/400 + (37*dq1*dqr2*cos(q2)*cos(q4)^2*cos(q5)*sin(q3)*sin(q5)*sin(q6))/500 - (37*dq1*dqr2*cos(q3)*cos(q4)^2*cos(q5)*sin(q2)*sin(q5)*sin(q6))/500 + dq1*dqr2*cos(q2)*cos(q4)^2*cos(q5)*cos(q6)*sin(q3)*((641*3^(1/2))/40000 - 37/4000) - dq1*dqr2*cos(q3)*cos(q4)^2*cos(q5)*cos(q6)*sin(q2)*((641*3^(1/2))/40000 - 37/4000) - dq1*dqr2*cos(q2)*cos(q4)^2*sin(q3)*sin(q5)*sin(q6)*((641*3^(1/2))/20000 + 37/1000) + dq1*dqr2*cos(q3)*cos(q4)^2*sin(q2)*sin(q5)*sin(q6)*((641*3^(1/2))/20000 + 37/1000) + (37*dq1*dqr2*cos(q2)*cos(q4)*cos(q5)*cos(q6)*sin(q3)*sin(q4)*sin(q5))/800 - (37*dq1*dqr2*cos(q3)*cos(q4)*cos(q5)*cos(q6)*sin(q2)*sin(q4)*sin(q5))/800 - dq1*dqr2*cos(q2)*cos(q4)*cos(q5)*sin(q3)*sin(q4)*sin(q6)*((641*3^(1/2))/40000 + 37/2000) + dq1*dqr2*cos(q3)*cos(q4)*cos(q5)*sin(q2)*sin(q4)*sin(q6)*((641*3^(1/2))/40000 + 37/2000) - dq1*dqr2*cos(q2)*cos(q4)*cos(q6)*sin(q3)*sin(q4)*sin(q5)*((641*3^(1/2))/80000 - 37/8000) + dq1*dqr2*cos(q3)*cos(q4)*cos(q6)*sin(q2)*sin(q4)*sin(q5)*((641*3^(1/2))/80000 - 37/8000) + (37*3^(1/2)*dq2*dqr1*cos(q2)*cos(q3)*cos(q4)*cos(q5)*cos(q6)*sin(q5))/4000 - (37*3^(1/2)*dq3*dqr1*cos(q2)*cos(q3)*cos(q4)*cos(q5)*cos(q6)*sin(q5))/4000 + (37*3^(1/2)*dq1*dqr2*cos(q4)*cos(q5)*cos(q6)*sin(q2)*sin(q3)*sin(q5))/4000 - (37*3^(1/2)*dq1*dqr2*cos(q5)*sin(q2)*sin(q3)*sin(q4)*sin(q5)*sin(q6))/1000;
Y5_10_4=(37*dq3*dqr2*sin(q6))/1000 - (37*dq2*dqr2*sin(q6))/1000 + (37*dq2*dqr2*cos(q4)^2*sin(q6))/800 + (37*dq2*dqr2*cos(q5)^2*sin(q6))/500 - (37*dq3*dqr2*cos(q4)^2*sin(q6))/800 - (37*dq3*dqr2*cos(q5)^2*sin(q6))/500 - (37*3^(1/2)*dq4*dqr2*cos(q4)*sin(q6))/4000 - (37*3^(1/2)*dq4*dqr2*cos(q6)*sin(q4))/2000 - (37*3^(1/2)*dq6*dqr2*cos(q4)*sin(q6))/4000 - (37*dq2*dqr2*cos(q4)^2*cos(q5)^2*sin(q6))/400 + (37*dq3*dqr2*cos(q4)^2*cos(q5)^2*sin(q6))/400 + (37*dq2*dqr2*cos(q4)*cos(q6)*sin(q4))/2000 - (37*dq3*dqr2*cos(q4)*cos(q6)*sin(q4))/2000 + (37*dq2*dqr2*cos(q5)*cos(q6)*sin(q5))/1000 - (37*dq3*dqr2*cos(q5)*cos(q6)*sin(q5))/1000 + dq2*dqr2*cos(q5)*sin(q6)*((117*3^(1/2))/1250 - 37/2000) - dq3*dqr2*cos(q5)*sin(q6)*((117*3^(1/2))/1250 - 37/2000) + dq2*dqr2*cos(q6)*sin(q5)*((117*3^(1/2))/2500 - 37/4000) - dq3*dqr2*cos(q6)*sin(q5)*((117*3^(1/2))/2500 - 37/4000) - (29*3^(1/2)*dq2*dqr2*cos(q3)*cos(q5)*sin(q6))/200 - (29*3^(1/2)*dq2*dqr2*cos(q3)*cos(q6)*sin(q5))/400 + (37*3^(1/2)*dq6*dqr2*cos(q4)*cos(q5)*sin(q6))/4000 + dq2*dqr2*cos(q4)^2*cos(q5)*sin(q6)*((641*3^(1/2))/40000 + 37/2000) - dq3*dqr2*cos(q4)^2*cos(q5)*sin(q6)*((641*3^(1/2))/40000 + 37/2000) + dq2*dqr2*cos(q4)^2*cos(q6)*sin(q5)*((641*3^(1/2))/80000 - 37/8000) - dq3*dqr2*cos(q4)^2*cos(q6)*sin(q5)*((641*3^(1/2))/80000 - 37/8000) - (37*3^(1/2)*dq6*dqr2*sin(q4)*sin(q5)*sin(q6))/2000 + (37*3^(1/2)*dq4*dqr2*cos(q4)*cos(q5)^2*sin(q6))/2000 + (37*3^(1/2)*dq4*dqr2*cos(q5)^2*cos(q6)*sin(q4))/2000 - (29*dq1*dqr2*cos(q2)*cos(q4)*cos(q5)*sin(q6))/200 - (29*dq1*dqr2*cos(q2)*cos(q4)*cos(q6)*sin(q5))/400 - (29*dq1*dqr2*cos(q2)*cos(q5)*cos(q6)*sin(q4))/200 + (29*dq1*dqr2*cos(q2)*sin(q4)*sin(q5)*sin(q6))/100 - dq4*dqr2*cos(q4)*cos(q5)*sin(q6)*((37*3^(1/2))/2000 + 1923/40000) + dq4*dqr2*cos(q4)*cos(q6)*sin(q5)*((37*3^(1/2))/8000 - 1923/80000) - (37*dq1*dqr3*cos(q2)*cos(q4)^2*cos(q6)*sin(q3))/2000 + (37*dq1*dqr3*cos(q3)*cos(q4)^2*cos(q6)*sin(q2))/2000 - (37*dq1*dqr3*cos(q2)*cos(q5)^2*cos(q6)*sin(q3))/2000 + (37*dq1*dqr3*cos(q3)*cos(q5)^2*cos(q6)*sin(q2))/2000 - (37*dq2*dqr2*cos(q4)*cos(q5)^2*cos(q6)*sin(q4))/1000 - (37*dq2*dqr2*cos(q4)^2*cos(q5)*cos(q6)*sin(q5))/800 + (37*dq3*dqr2*cos(q4)*cos(q5)^2*cos(q6)*sin(q4))/1000 + (37*dq3*dqr2*cos(q4)^2*cos(q5)*cos(q6)*sin(q5))/800 + (37*3^(1/2)*dq1*dqr3*cos(q4)*sin(q2)*sin(q3)*sin(q6))/4000 - (37*3^(1/2)*dq4*dqr2*cos(q5)*sin(q4)*sin(q5)*sin(q6))/1000 + (37*3^(1/2)*dq4*dqr3*cos(q5)*sin(q4)*sin(q5)*sin(q6))/1000 + (37*dq1*dqr3*cos(q2)*cos(q4)^2*cos(q5)^2*cos(q6)*sin(q3))/1000 - (37*dq1*dqr3*cos(q3)*cos(q4)^2*cos(q5)^2*cos(q6)*sin(q2))/1000 + (877*dq1*dqr2*cos(q2)*cos(q3)*cos(q4)*cos(q5)*sin(q6))/8000 - (877*dq1*dqr2*cos(q2)*cos(q3)*sin(q4)*sin(q5)*sin(q6))/4000 + (37*dq1*dqr3*cos(q2)*cos(q4)*sin(q3)*sin(q4)*sin(q6))/800 - (37*dq1*dqr3*cos(q3)*cos(q4)*sin(q2)*sin(q4)*sin(q6))/800 + (877*dq1*dqr3*cos(q2)*cos(q3)*sin(q4)*sin(q5)*sin(q6))/4000 - (877*dq1*dqr3*cos(q4)*cos(q5)*sin(q2)*sin(q3)*sin(q6))/8000 + (37*dq1*dqr3*cos(q2)*cos(q5)*sin(q3)*sin(q5)*sin(q6))/1000 - (37*dq1*dqr3*cos(q3)*cos(q5)*sin(q2)*sin(q5)*sin(q6))/1000 + (37*dq2*dqr2*cos(q4)*cos(q5)*sin(q4)*sin(q5)*sin(q6))/500 - (37*dq2*dqr3*cos(q4)*cos(q5)*sin(q4)*sin(q5)*sin(q6))/500 - (37*dq3*dqr2*cos(q4)*cos(q5)*sin(q4)*sin(q5)*sin(q6))/500 + (37*dq3*dqr3*cos(q4)*cos(q5)*sin(q4)*sin(q5)*sin(q6))/500 + (877*dq1*dqr3*sin(q2)*sin(q3)*sin(q4)*sin(q5)*sin(q6))/4000 + dq1*dqr3*cos(q2)*cos(q5)*cos(q6)*sin(q3)*((641*3^(1/2))/40000 - 37/4000) - dq1*dqr3*cos(q3)*cos(q5)*cos(q6)*sin(q2)*((641*3^(1/2))/40000 - 37/4000) + dq2*dqr2*cos(q4)*cos(q5)*cos(q6)*sin(q4)*((641*3^(1/2))/40000 - 37/4000) - dq3*dqr2*cos(q4)*cos(q5)*cos(q6)*sin(q4)*((641*3^(1/2))/40000 - 37/4000) - dq1*dqr3*cos(q2)*sin(q3)*sin(q5)*sin(q6)*((641*3^(1/2))/20000 + 37/1000) + dq1*dqr3*cos(q3)*sin(q2)*sin(q5)*sin(q6)*((641*3^(1/2))/20000 + 37/1000) - dq2*dqr2*cos(q4)*sin(q4)*sin(q5)*sin(q6)*((641*3^(1/2))/20000 + 37/1000) + dq2*dqr3*cos(q4)*sin(q4)*sin(q5)*sin(q6)*((641*3^(1/2))/20000 + 37/1000) + dq3*dqr2*cos(q4)*sin(q4)*sin(q5)*sin(q6)*((641*3^(1/2))/20000 + 37/1000) - dq3*dqr3*cos(q4)*sin(q4)*sin(q5)*sin(q6)*((641*3^(1/2))/20000 + 37/1000) - (37*3^(1/2)*dq1*dqr2*cos(q2)*cos(q3)*cos(q4)*sin(q6))/4000 + (37*3^(1/2)*dq4*dqr2*cos(q4)*cos(q5)*cos(q6)*sin(q5))/4000 + (37*3^(1/2)*dq1*dqr2*cos(q2)*cos(q3)*cos(q4)*cos(q5)^2*sin(q6))/2000 + (37*3^(1/2)*dq1*dqr2*cos(q2)*cos(q3)*cos(q5)^2*cos(q6)*sin(q4))/2000 - (37*3^(1/2)*dq1*dqr3*cos(q4)*cos(q5)^2*sin(q2)*sin(q3)*sin(q6))/2000 - (37*3^(1/2)*dq1*dqr3*cos(q5)^2*cos(q6)*sin(q2)*sin(q3)*sin(q4))/2000 - dq1*dqr2*cos(q2)*cos(q3)*cos(q5)*cos(q6)*sin(q4)*((37*3^(1/2))/4000 - 877/8000) - dq1*dqr2*cos(q2)*cos(q3)*cos(q4)*cos(q6)*sin(q5)*((37*3^(1/2))/8000 - 877/16000) + dq1*dqr3*cos(q5)*cos(q6)*sin(q2)*sin(q3)*sin(q4)*((37*3^(1/2))/4000 - 877/8000) + dq1*dqr3*cos(q4)*cos(q6)*sin(q2)*sin(q3)*sin(q5)*((37*3^(1/2))/8000 - 877/16000) - (37*dq1*dqr3*cos(q2)*cos(q4)*cos(q5)^2*sin(q3)*sin(q4)*sin(q6))/400 + (37*dq1*dqr3*cos(q3)*cos(q4)*cos(q5)^2*sin(q2)*sin(q4)*sin(q6))/400 - (37*dq1*dqr3*cos(q2)*cos(q4)^2*cos(q5)*sin(q3)*sin(q5)*sin(q6))/500 + (37*dq1*dqr3*cos(q3)*cos(q4)^2*cos(q5)*sin(q2)*sin(q5)*sin(q6))/500 - dq1*dqr3*cos(q2)*cos(q4)^2*cos(q5)*cos(q6)*sin(q3)*((641*3^(1/2))/40000 - 37/4000) + dq1*dqr3*cos(q3)*cos(q4)^2*cos(q5)*cos(q6)*sin(q2)*((641*3^(1/2))/40000 - 37/4000) + dq1*dqr3*cos(q2)*cos(q4)^2*sin(q3)*sin(q5)*sin(q6)*((641*3^(1/2))/20000 + 37/1000) - dq1*dqr3*cos(q3)*cos(q4)^2*sin(q2)*sin(q5)*sin(q6)*((641*3^(1/2))/20000 + 37/1000) - (37*dq1*dqr3*cos(q2)*cos(q4)*cos(q5)*cos(q6)*sin(q3)*sin(q4)*sin(q5))/800 + (37*dq1*dqr3*cos(q3)*cos(q4)*cos(q5)*cos(q6)*sin(q2)*sin(q4)*sin(q5))/800 + dq1*dqr3*cos(q2)*cos(q4)*cos(q5)*sin(q3)*sin(q4)*sin(q6)*((641*3^(1/2))/40000 + 37/2000) - dq1*dqr3*cos(q3)*cos(q4)*cos(q5)*sin(q2)*sin(q4)*sin(q6)*((641*3^(1/2))/40000 + 37/2000) + dq1*dqr3*cos(q2)*cos(q4)*cos(q6)*sin(q3)*sin(q4)*sin(q5)*((641*3^(1/2))/80000 - 37/8000) - dq1*dqr3*cos(q3)*cos(q4)*cos(q6)*sin(q2)*sin(q4)*sin(q5)*((641*3^(1/2))/80000 - 37/8000) + (37*3^(1/2)*dq1*dqr2*cos(q2)*cos(q3)*cos(q4)*cos(q5)*cos(q6)*sin(q5))/4000 - (37*3^(1/2)*dq1*dqr2*cos(q2)*cos(q3)*cos(q5)*sin(q4)*sin(q5)*sin(q6))/1000 + (37*3^(1/2)*dq1*dqr3*cos(q2)*cos(q3)*cos(q5)*sin(q4)*sin(q5)*sin(q6))/1000 - (37*3^(1/2)*dq1*dqr3*cos(q4)*cos(q5)*cos(q6)*sin(q2)*sin(q3)*sin(q5))/4000 + (37*3^(1/2)*dq1*dqr3*cos(q5)*sin(q2)*sin(q3)*sin(q4)*sin(q5)*sin(q6))/1000;
Y5_10_5=(37*dq2*dqr3*sin(q6))/1000 - (37*dq3*dqr3*sin(q6))/1000 + (111*dq4*dqr4*sin(q6))/4000 - (37*dq6*dqr4*sin(q6))/4000 - (37*dq6*dqr5*sin(q6))/2000 - (37*dq2*dqr3*cos(q4)^2*sin(q6))/800 - (37*dq2*dqr3*cos(q5)^2*sin(q6))/500 + (37*dq3*dqr3*cos(q4)^2*sin(q6))/800 + (37*dq3*dqr3*cos(q5)^2*sin(q6))/500 - (111*dq4*dqr4*cos(q5)^2*sin(q6))/2000 - (111*dq6*dqr4*cos(q5)*sin(q6))/4000 - (37*3^(1/2)*dq2*dqr4*cos(q4)*sin(q6))/4000 - (37*3^(1/2)*dq2*dqr4*cos(q6)*sin(q4))/2000 + (37*3^(1/2)*dq3*dqr4*cos(q4)*sin(q6))/4000 + (37*3^(1/2)*dq3*dqr4*cos(q6)*sin(q4))/2000 + (37*3^(1/2)*dq4*dqr3*cos(q4)*sin(q6))/4000 + (37*3^(1/2)*dq4*dqr3*cos(q6)*sin(q4))/2000 + (37*3^(1/2)*dq6*dqr3*cos(q4)*sin(q6))/4000 + (37*dq2*dqr3*cos(q4)^2*cos(q5)^2*sin(q6))/400 - (37*dq3*dqr3*cos(q4)^2*cos(q5)^2*sin(q6))/400 + (111*dq1*dqr4*cos(q2)*cos(q3)*sin(q6))/4000 - (37*dq2*dqr3*cos(q4)*cos(q6)*sin(q4))/2000 + (37*dq3*dqr3*cos(q4)*cos(q6)*sin(q4))/2000 - (37*dq2*dqr3*cos(q5)*cos(q6)*sin(q5))/1000 + (37*dq3*dqr3*cos(q5)*cos(q6)*sin(q5))/1000 - (111*dq4*dqr4*cos(q5)*cos(q6)*sin(q5))/4000 + (111*dq1*dqr4*sin(q2)*sin(q3)*sin(q6))/4000 - (37*dq1*dqr6*sin(q2)*sin(q3)*sin(q6))/4000 - dq2*dqr3*cos(q5)*sin(q6)*((117*3^(1/2))/1250 - 37/2000) + dq3*dqr3*cos(q5)*sin(q6)*((117*3^(1/2))/1250 - 37/2000) - dq2*dqr3*cos(q6)*sin(q5)*((117*3^(1/2))/2500 - 37/4000) + dq3*dqr3*cos(q6)*sin(q5)*((117*3^(1/2))/2500 - 37/4000) - dq4*dqr4*cos(q5)*sin(q6)*((641*3^(1/2))/40000 + 37/2000) - dq4*dqr4*cos(q6)*sin(q5)*((641*3^(1/2))/80000 - 37/8000) - (111*dq1*dqr4*cos(q5)^2*sin(q2)*sin(q3)*sin(q6))/2000 - (37*3^(1/2)*dq6*dqr3*cos(q4)*cos(q5)*sin(q6))/4000 - dq2*dqr3*cos(q4)^2*cos(q5)*sin(q6)*((641*3^(1/2))/40000 + 37/2000) + dq3*dqr3*cos(q4)^2*cos(q5)*sin(q6)*((641*3^(1/2))/40000 + 37/2000) - dq2*dqr3*cos(q4)^2*cos(q6)*sin(q5)*((641*3^(1/2))/80000 - 37/8000) + dq3*dqr3*cos(q4)^2*cos(q6)*sin(q5)*((641*3^(1/2))/80000 - 37/8000) + (37*3^(1/2)*dq6*dqr3*sin(q4)*sin(q5)*sin(q6))/2000 + (37*3^(1/2)*dq2*dqr4*cos(q4)*cos(q5)^2*sin(q6))/2000 + (37*3^(1/2)*dq2*dqr4*cos(q5)^2*cos(q6)*sin(q4))/2000 - (37*3^(1/2)*dq3*dqr4*cos(q4)*cos(q5)^2*sin(q6))/2000 - (37*3^(1/2)*dq3*dqr4*cos(q5)^2*cos(q6)*sin(q4))/2000 - (37*3^(1/2)*dq4*dqr3*cos(q4)*cos(q5)^2*sin(q6))/2000 - (37*3^(1/2)*dq4*dqr3*cos(q5)^2*cos(q6)*sin(q4))/2000 - (111*dq1*dqr6*cos(q5)*sin(q2)*sin(q3)*sin(q6))/4000 - dq2*dqr4*cos(q4)*cos(q5)*sin(q6)*((37*3^(1/2))/2000 + 1923/40000) + dq3*dqr4*cos(q4)*cos(q5)*sin(q6)*((37*3^(1/2))/2000 + 1923/40000) + dq4*dqr3*cos(q4)*cos(q5)*sin(q6)*((37*3^(1/2))/2000 + 1923/40000) + dq2*dqr4*cos(q4)*cos(q6)*sin(q5)*((37*3^(1/2))/8000 - 1923/80000) - dq3*dqr4*cos(q4)*cos(q6)*sin(q5)*((37*3^(1/2))/8000 - 1923/80000) - dq4*dqr3*cos(q4)*cos(q6)*sin(q5)*((37*3^(1/2))/8000 - 1923/80000) - (111*dq1*dqr4*cos(q2)*cos(q3)*cos(q5)^2*sin(q6))/2000 + (37*dq2*dqr3*cos(q4)*cos(q5)^2*cos(q6)*sin(q4))/1000 + (37*dq2*dqr3*cos(q4)^2*cos(q5)*cos(q6)*sin(q5))/800 - (37*dq3*dqr3*cos(q4)*cos(q5)^2*cos(q6)*sin(q4))/1000 - (37*dq3*dqr3*cos(q4)^2*cos(q5)*cos(q6)*sin(q5))/800 + (37*3^(1/2)*dq1*dqr4*cos(q2)*sin(q3)*sin(q4)*sin(q6))/4000 - (37*3^(1/2)*dq1*dqr4*cos(q3)*sin(q2)*sin(q4)*sin(q6))/4000 + (37*3^(1/2)*dq1*dqr6*cos(q2)*sin(q3)*sin(q4)*sin(q6))/4000 - (37*3^(1/2)*dq1*dqr6*cos(q3)*sin(q2)*sin(q4)*sin(q6))/4000 - (37*3^(1/2)*dq2*dqr4*cos(q5)*sin(q4)*sin(q5)*sin(q6))/1000 + (37*3^(1/2)*dq3*dqr4*cos(q5)*sin(q4)*sin(q5)*sin(q6))/1000 - (877*dq1*dqr3*cos(q2)*cos(q3)*cos(q4)*cos(q5)*sin(q6))/8000 - (111*dq1*dqr4*cos(q2)*cos(q3)*cos(q5)*cos(q6)*sin(q5))/4000 - (111*dq1*dqr4*cos(q5)*cos(q6)*sin(q2)*sin(q3)*sin(q5))/4000 - dq1*dqr4*cos(q2)*cos(q3)*cos(q5)*sin(q6)*((641*3^(1/2))/40000 + 37/2000) - dq2*dqr3*cos(q4)*cos(q5)*cos(q6)*sin(q4)*((641*3^(1/2))/40000 - 37/4000) + dq3*dqr3*cos(q4)*cos(q5)*cos(q6)*sin(q4)*((641*3^(1/2))/40000 - 37/4000) - dq1*dqr4*cos(q2)*cos(q3)*cos(q6)*sin(q5)*((641*3^(1/2))/80000 - 37/8000) - dq1*dqr4*cos(q5)*sin(q2)*sin(q3)*sin(q6)*((641*3^(1/2))/40000 + 37/2000) - dq1*dqr4*cos(q6)*sin(q2)*sin(q3)*sin(q5)*((641*3^(1/2))/80000 - 37/8000) + (37*3^(1/2)*dq1*dqr3*cos(q2)*cos(q3)*cos(q4)*sin(q6))/4000 - (37*3^(1/2)*dq1*dqr4*cos(q2)*cos(q4)*cos(q6)*sin(q3))/2000 + (37*3^(1/2)*dq1*dqr4*cos(q3)*cos(q4)*cos(q6)*sin(q2))/2000 + (37*3^(1/2)*dq2*dqr4*cos(q4)*cos(q5)*cos(q6)*sin(q5))/4000 - (37*3^(1/2)*dq3*dqr4*cos(q4)*cos(q5)*cos(q6)*sin(q5))/4000 - (37*3^(1/2)*dq4*dqr3*cos(q4)*cos(q5)*cos(q6)*sin(q5))/4000 - (37*3^(1/2)*dq1*dqr3*cos(q2)*cos(q3)*cos(q4)*cos(q5)^2*sin(q6))/2000 - (37*3^(1/2)*dq1*dqr3*cos(q2)*cos(q3)*cos(q5)^2*cos(q6)*sin(q4))/2000 + (37*3^(1/2)*dq1*dqr4*cos(q2)*cos(q4)*cos(q5)^2*cos(q6)*sin(q3))/2000 - (37*3^(1/2)*dq1*dqr4*cos(q3)*cos(q4)*cos(q5)^2*cos(q6)*sin(q2))/2000 - (37*3^(1/2)*dq1*dqr4*cos(q2)*cos(q5)^2*sin(q3)*sin(q4)*sin(q6))/2000 + (37*3^(1/2)*dq1*dqr4*cos(q3)*cos(q5)^2*sin(q2)*sin(q4)*sin(q6))/2000 + dq1*dqr3*cos(q2)*cos(q3)*cos(q5)*cos(q6)*sin(q4)*((37*3^(1/2))/4000 - 877/8000) + dq1*dqr3*cos(q2)*cos(q3)*cos(q4)*cos(q6)*sin(q5)*((37*3^(1/2))/8000 - 877/16000) + dq1*dqr4*cos(q2)*cos(q5)*sin(q3)*sin(q4)*sin(q6)*((37*3^(1/2))/2000 + 1923/40000) - dq1*dqr4*cos(q3)*cos(q5)*sin(q2)*sin(q4)*sin(q6)*((37*3^(1/2))/2000 + 1923/40000) - dq1*dqr4*cos(q2)*cos(q6)*sin(q3)*sin(q4)*sin(q5)*((37*3^(1/2))/8000 - 1923/80000) + dq1*dqr4*cos(q3)*cos(q6)*sin(q2)*sin(q4)*sin(q5)*((37*3^(1/2))/8000 - 1923/80000) - (37*3^(1/2)*dq1*dqr6*cos(q2)*cos(q5)*sin(q3)*sin(q4)*sin(q6))/4000 + (37*3^(1/2)*dq1*dqr6*cos(q3)*cos(q4)*sin(q2)*sin(q5)*sin(q6))/2000 + (37*3^(1/2)*dq1*dqr6*cos(q3)*cos(q5)*sin(q2)*sin(q4)*sin(q6))/4000 - (37*3^(1/2)*dq1*dqr3*cos(q2)*cos(q3)*cos(q4)*cos(q5)*cos(q6)*sin(q5))/4000 - (37*3^(1/2)*dq1*dqr4*cos(q2)*cos(q4)*cos(q5)*sin(q3)*sin(q5)*sin(q6))/1000 - (37*3^(1/2)*dq1*dqr4*cos(q2)*cos(q5)*cos(q6)*sin(q3)*sin(q4)*sin(q5))/4000 + (37*3^(1/2)*dq1*dqr4*cos(q3)*cos(q4)*cos(q5)*sin(q2)*sin(q5)*sin(q6))/1000 + (37*3^(1/2)*dq1*dqr4*cos(q3)*cos(q5)*cos(q6)*sin(q2)*sin(q4)*sin(q5))/4000;
Y5_10_6=(37*ddqr4*cos(q6))/2000 + (37*ddqr5*cos(q6))/1000 + (37*ddqr6*cos(q6))/1000 - (37*dq4*dqr6*sin(q6))/4000 - (37*dq5*dqr6*sin(q6))/2000 - (37*dq6*dqr6*sin(q6))/1000 + (37*ddqr1*cos(q2)*cos(q3)*cos(q6))/2000 + (37*ddqr1*cos(q6)*sin(q2)*sin(q3))/2000 - (877*ddqr2*cos(q4)*sin(q5)*sin(q6))/4000 + (877*ddqr3*cos(q4)*sin(q5)*sin(q6))/4000 - ddqr4*cos(q5)*cos(q6)*((641*3^(1/2))/40000 - 37/4000) + ddqr4*sin(q5)*sin(q6)*((641*3^(1/2))/20000 + 37/1000) + (37*3^(1/2)*ddqr2*cos(q4)*cos(q6))/2000 - (37*3^(1/2)*ddqr3*cos(q4)*cos(q6))/2000 - (111*dq4*dqr6*cos(q5)*sin(q6))/4000 - (29*ddqr2*cos(q3)*cos(q4)*cos(q5)*cos(q6))/200 - (29*ddqr1*cos(q4)*cos(q5)*sin(q2)*sin(q6))/200 - (29*ddqr1*cos(q4)*cos(q6)*sin(q2)*sin(q5))/400 - (29*ddqr1*cos(q5)*cos(q6)*sin(q2)*sin(q4))/200 + (29*ddqr2*cos(q3)*cos(q4)*sin(q5)*sin(q6))/100 + (29*ddqr2*cos(q3)*cos(q5)*sin(q4)*sin(q6))/200 + (29*ddqr2*cos(q3)*cos(q6)*sin(q4)*sin(q5))/400 - (37*3^(1/2)*dq2*dqr6*cos(q4)*sin(q6))/4000 + (37*3^(1/2)*dq3*dqr6*cos(q4)*sin(q6))/4000 + (29*ddqr1*sin(q2)*sin(q4)*sin(q5)*sin(q6))/100 - ddqr2*cos(q4)*cos(q5)*cos(q6)*((37*3^(1/2))/4000 - 877/8000) + ddqr3*cos(q4)*cos(q5)*cos(q6)*((37*3^(1/2))/4000 - 877/8000) - ddqr2*cos(q5)*sin(q4)*sin(q6)*((37*3^(1/2))/2000 + 1577/10000) + ddqr3*cos(q5)*sin(q4)*sin(q6)*((37*3^(1/2))/2000 + 1577/10000) + ddqr2*cos(q6)*sin(q4)*sin(q5)*((37*3^(1/2))/4000 - 1577/20000) - ddqr3*cos(q6)*sin(q4)*sin(q5)*((37*3^(1/2))/4000 - 1577/20000) - (37*dq1*dqr6*cos(q2)*cos(q3)*sin(q6))/4000 - (29*3^(1/2)*ddqr2*cos(q5)*sin(q3)*sin(q6))/200 - (29*3^(1/2)*ddqr2*cos(q6)*sin(q3)*sin(q5))/400 - (7*ddqr1*cos(q2)*cos(q3)*cos(q4)*sin(q5)*sin(q6))/1000 - (7*ddqr1*cos(q2)*cos(q3)*cos(q5)*sin(q4)*sin(q6))/2000 - (7*ddqr1*cos(q2)*cos(q3)*cos(q6)*sin(q4)*sin(q5))/4000 + (7*ddqr1*cos(q4)*cos(q5)*cos(q6)*sin(q2)*sin(q3))/2000 + (37*3^(1/2)*dq2*dqr6*cos(q4)*cos(q5)*sin(q6))/4000 - (37*3^(1/2)*dq3*dqr6*cos(q4)*cos(q5)*sin(q6))/4000 + (877*ddqr1*cos(q2)*sin(q3)*sin(q4)*sin(q5)*sin(q6))/4000 - (877*ddqr1*cos(q3)*sin(q2)*sin(q4)*sin(q5)*sin(q6))/4000 - (7*ddqr1*cos(q4)*sin(q2)*sin(q3)*sin(q5)*sin(q6))/1000 - (7*ddqr1*cos(q5)*sin(q2)*sin(q3)*sin(q4)*sin(q6))/2000 - (7*ddqr1*cos(q6)*sin(q2)*sin(q3)*sin(q4)*sin(q5))/4000 - ddqr1*cos(q2)*cos(q3)*cos(q5)*cos(q6)*((641*3^(1/2))/40000 - 37/4000) - (37*3^(1/2)*dq2*dqr6*sin(q4)*sin(q5)*sin(q6))/2000 + (37*3^(1/2)*dq3*dqr6*sin(q4)*sin(q5)*sin(q6))/2000 + ddqr1*cos(q2)*cos(q3)*sin(q5)*sin(q6)*((641*3^(1/2))/20000 + 37/1000) - ddqr1*cos(q5)*cos(q6)*sin(q2)*sin(q3)*((641*3^(1/2))/40000 - 37/4000) + ddqr1*sin(q2)*sin(q3)*sin(q5)*sin(q6)*((641*3^(1/2))/20000 + 37/1000) - (111*dq1*dqr6*cos(q2)*cos(q3)*cos(q5)*sin(q6))/4000 - (37*3^(1/2)*ddqr1*cos(q2)*cos(q6)*sin(q3)*sin(q4))/2000 + (37*3^(1/2)*ddqr1*cos(q3)*cos(q6)*sin(q2)*sin(q4))/2000 + (7*3^(1/2)*ddqr1*cos(q2)*cos(q5)*sin(q3)*sin(q6))/2000 + (7*3^(1/2)*ddqr1*cos(q2)*cos(q6)*sin(q3)*sin(q5))/4000 - (7*3^(1/2)*ddqr1*cos(q3)*cos(q5)*sin(q2)*sin(q6))/2000 - (7*3^(1/2)*ddqr1*cos(q3)*cos(q6)*sin(q2)*sin(q5))/4000 + (7*ddqr1*cos(q2)*cos(q3)*cos(q4)*cos(q5)*cos(q6))/2000 + ddqr1*cos(q2)*cos(q5)*cos(q6)*sin(q3)*sin(q4)*((37*3^(1/2))/4000 - 877/8000) - ddqr1*cos(q3)*cos(q5)*cos(q6)*sin(q2)*sin(q4)*((37*3^(1/2))/4000 - 877/8000) - ddqr1*cos(q2)*cos(q4)*cos(q5)*sin(q3)*sin(q6)*((37*3^(1/2))/2000 + 1577/10000) + ddqr1*cos(q3)*cos(q4)*cos(q5)*sin(q2)*sin(q6)*((37*3^(1/2))/2000 + 1577/10000) + ddqr1*cos(q2)*cos(q4)*cos(q6)*sin(q3)*sin(q5)*((37*3^(1/2))/4000 - 1577/20000) - ddqr1*cos(q3)*cos(q4)*cos(q6)*sin(q2)*sin(q5)*((37*3^(1/2))/4000 - 1577/20000) - (37*3^(1/2)*dq1*dqr6*cos(q2)*cos(q4)*sin(q3)*sin(q5)*sin(q6))/2000;
Y5_14_1=(37*cos(q2)*cos(q4)*cos(q5)*sin(q3))/1000 - (37*3^(1/2)*sin(q2)*sin(q3)*sin(q5))/2000 - (37*3^(1/2)*cos(q2)*cos(q3)*sin(q5))/2000 - (37*cos(q3)*cos(q4)*cos(q5)*sin(q2))/1000 - (37*cos(q2)*sin(q3)*sin(q4)*sin(q5))/2000 + (37*cos(q3)*sin(q2)*sin(q4)*sin(q5))/2000;
Y5_19_1=(dq2*dqr2*sin(2*q4))/4 - (3*dq1*dqr1*sin(2*q5))/8 + (dq2*dqr2*sin(2*q5))/2 - (dq3*dqr2*sin(2*q4))/4 - (dq3*dqr2*sin(2*q5))/2 - (3^(1/2)*dq4*dqr2*sin(q4))/2 + (3^(1/2)*dq4*dqr3*sin(q4))/2 - (dq1*dqr1*cos(q2)^2*cos(q4)*sin(q4))/2 + (dq1*dqr2*cos(q2)*cos(q4)^2*sin(q3))/2 - (dq1*dqr2*cos(q3)*cos(q4)^2*sin(q2))/2 + (dq2*dqr1*cos(q2)*cos(q4)^2*sin(q3))/2 - (dq2*dqr1*cos(q3)*cos(q4)^2*sin(q2))/2 - (dq1*dqr1*cos(q3)^2*cos(q4)*sin(q4))/2 + (dq1*dqr2*cos(q2)*cos(q5)^2*sin(q3))/2 - (dq1*dqr2*cos(q3)*cos(q5)^2*sin(q2))/2 - (dq1*dqr3*cos(q2)*cos(q4)^2*sin(q3))/2 + (dq1*dqr3*cos(q3)*cos(q4)^2*sin(q2))/2 + (dq2*dqr1*cos(q2)*cos(q5)^2*sin(q3))/2 - (dq2*dqr1*cos(q3)*cos(q5)^2*sin(q2))/2 - (dq3*dqr1*cos(q2)*cos(q4)^2*sin(q3))/2 + (dq3*dqr1*cos(q3)*cos(q4)^2*sin(q2))/2 + (dq1*dqr1*cos(q2)^2*cos(q5)*sin(q5))/2 - (dq1*dqr3*cos(q2)*cos(q5)^2*sin(q3))/2 + (dq1*dqr3*cos(q3)*cos(q5)^2*sin(q2))/2 - (dq3*dqr1*cos(q2)*cos(q5)^2*sin(q3))/2 + (dq3*dqr1*cos(q3)*cos(q5)^2*sin(q2))/2 + (dq1*dqr1*cos(q3)^2*cos(q5)*sin(q5))/2 - dq2*dqr2*cos(q4)*cos(q5)^2*sin(q4) - (5*dq2*dqr2*cos(q4)^2*cos(q5)*sin(q5))/4 + dq2*dqr3*cos(q4)*cos(q5)^2*sin(q4) + dq3*dqr2*cos(q4)*cos(q5)^2*sin(q4) + (5*dq3*dqr2*cos(q4)^2*cos(q5)*sin(q5))/4 - dq3*dqr3*cos(q4)*cos(q5)^2*sin(q4) + (3^(1/2)*dq4*dqr2*cos(q5)^2*sin(q4))/2 - (3^(1/2)*dq4*dqr3*cos(q5)^2*sin(q4))/2 - (3^(1/2)*dq1*dqr1*cos(q2)*cos(q4)*sin(q2))/2 + (3^(1/2)*dq1*dqr1*cos(q3)*cos(q4)*sin(q3))/2 - (3^(1/2)*dq4*dqr1*cos(q2)*cos(q4)*sin(q3))/2 + (3^(1/2)*dq4*dqr1*cos(q3)*cos(q4)*sin(q2))/2 + (3^(1/2)*dq4*dqr2*cos(q4)*cos(q5)*sin(q5))/4 + dq1*dqr1*cos(q2)^2*cos(q3)^2*cos(q4)*sin(q4) + dq1*dqr1*cos(q2)^2*cos(q4)*cos(q5)^2*sin(q4) - dq1*dqr1*cos(q2)^2*cos(q3)^2*cos(q5)*sin(q5) - dq1*dqr2*cos(q2)*cos(q4)^2*cos(q5)^2*sin(q3) + dq1*dqr2*cos(q3)*cos(q4)^2*cos(q5)^2*sin(q2) - dq2*dqr1*cos(q2)*cos(q4)^2*cos(q5)^2*sin(q3) + dq2*dqr1*cos(q3)*cos(q4)^2*cos(q5)^2*sin(q2) + (5*dq1*dqr1*cos(q2)^2*cos(q4)^2*cos(q5)*sin(q5))/4 + dq1*dqr1*cos(q3)^2*cos(q4)*cos(q5)^2*sin(q4) + dq1*dqr3*cos(q2)*cos(q4)^2*cos(q5)^2*sin(q3) - dq1*dqr3*cos(q3)*cos(q4)^2*cos(q5)^2*sin(q2) + dq3*dqr1*cos(q2)*cos(q4)^2*cos(q5)^2*sin(q3) - dq3*dqr1*cos(q3)*cos(q4)^2*cos(q5)^2*sin(q2) + (5*dq1*dqr1*cos(q3)^2*cos(q4)^2*cos(q5)*sin(q5))/4 - (3*dq4*dqr1*cos(q2)*cos(q3)*cos(q5)*sin(q5))/4 - (3*dq4*dqr1*cos(q5)*sin(q2)*sin(q3)*sin(q5))/4 + 3^(1/2)*dq1*dqr1*cos(q2)*cos(q3)^2*cos(q4)*sin(q2) - 3^(1/2)*dq1*dqr1*cos(q2)^2*cos(q3)*cos(q4)*sin(q3) + 3^(1/2)*dq1*dqr1*cos(q2)*cos(q4)*cos(q5)^2*sin(q2) - 3^(1/2)*dq1*dqr1*cos(q3)*cos(q4)*cos(q5)^2*sin(q3) + (3^(1/2)*dq1*dqr2*cos(q2)*cos(q3)*cos(q5)^2*sin(q4))/2 + (3^(1/2)*dq2*dqr1*cos(q2)*cos(q3)*cos(q5)^2*sin(q4))/2 - (3^(1/2)*dq1*dqr3*cos(q2)*cos(q3)*cos(q5)^2*sin(q4))/2 - (3^(1/2)*dq3*dqr1*cos(q2)*cos(q3)*cos(q5)^2*sin(q4))/2 + (3^(1/2)*dq4*dqr1*cos(q2)*cos(q4)*cos(q5)^2*sin(q3))/2 - (3^(1/2)*dq4*dqr1*cos(q3)*cos(q4)*cos(q5)^2*sin(q2))/2 + (3^(1/2)*dq1*dqr2*cos(q5)^2*sin(q2)*sin(q3)*sin(q4))/2 + (3^(1/2)*dq2*dqr1*cos(q5)^2*sin(q2)*sin(q3)*sin(q4))/2 - (3^(1/2)*dq1*dqr3*cos(q5)^2*sin(q2)*sin(q3)*sin(q4))/2 - (3^(1/2)*dq3*dqr1*cos(q5)^2*sin(q2)*sin(q3)*sin(q4))/2 - 2*dq1*dqr1*cos(q2)^2*cos(q3)^2*cos(q4)*cos(q5)^2*sin(q4) - (5*dq1*dqr1*cos(q2)^2*cos(q3)^2*cos(q4)^2*cos(q5)*sin(q5))/2 + dq1*dqr1*cos(q2)*cos(q3)*cos(q4)*sin(q2)*sin(q3)*sin(q4) - dq1*dqr1*cos(q2)*cos(q3)*cos(q5)*sin(q2)*sin(q3)*sin(q5) + (5*dq1*dqr2*cos(q2)*cos(q4)*cos(q5)*sin(q3)*sin(q4)*sin(q5))/4 - (5*dq1*dqr2*cos(q3)*cos(q4)*cos(q5)*sin(q2)*sin(q4)*sin(q5))/4 + (5*dq2*dqr1*cos(q2)*cos(q4)*cos(q5)*sin(q3)*sin(q4)*sin(q5))/4 - (5*dq2*dqr1*cos(q3)*cos(q4)*cos(q5)*sin(q2)*sin(q4)*sin(q5))/4 - (5*dq1*dqr3*cos(q2)*cos(q4)*cos(q5)*sin(q3)*sin(q4)*sin(q5))/4 + (5*dq1*dqr3*cos(q3)*cos(q4)*cos(q5)*sin(q2)*sin(q4)*sin(q5))/4 - (5*dq3*dqr1*cos(q2)*cos(q4)*cos(q5)*sin(q3)*sin(q4)*sin(q5))/4 + (5*dq3*dqr1*cos(q3)*cos(q4)*cos(q5)*sin(q2)*sin(q4)*sin(q5))/4 - 2*3^(1/2)*dq1*dqr1*cos(q2)*cos(q3)^2*cos(q4)*cos(q5)^2*sin(q2) + 2*3^(1/2)*dq1*dqr1*cos(q2)^2*cos(q3)*cos(q4)*cos(q5)^2*sin(q3) + (3^(1/2)*dq1*dqr2*cos(q2)*cos(q3)*cos(q4)*cos(q5)*sin(q5))/4 + (3^(1/2)*dq2*dqr1*cos(q2)*cos(q3)*cos(q4)*cos(q5)*sin(q5))/4 - (3^(1/2)*dq1*dqr3*cos(q2)*cos(q3)*cos(q4)*cos(q5)*sin(q5))/4 - (3^(1/2)*dq3*dqr1*cos(q2)*cos(q3)*cos(q4)*cos(q5)*sin(q5))/4 - (3^(1/2)*dq1*dqr1*cos(q2)*cos(q5)*sin(q2)*sin(q4)*sin(q5))/2 + (3^(1/2)*dq1*dqr1*cos(q3)*cos(q5)*sin(q3)*sin(q4)*sin(q5))/2 + (3^(1/2)*dq1*dqr2*cos(q4)*cos(q5)*sin(q2)*sin(q3)*sin(q5))/4 + (3^(1/2)*dq2*dqr1*cos(q4)*cos(q5)*sin(q2)*sin(q3)*sin(q5))/4 - (3^(1/2)*dq1*dqr3*cos(q4)*cos(q5)*sin(q2)*sin(q3)*sin(q5))/4 - (3^(1/2)*dq3*dqr1*cos(q4)*cos(q5)*sin(q2)*sin(q3)*sin(q5))/4 - (3^(1/2)*dq4*dqr1*cos(q2)*cos(q5)*sin(q3)*sin(q4)*sin(q5))/4 + (3^(1/2)*dq4*dqr1*cos(q3)*cos(q5)*sin(q2)*sin(q4)*sin(q5))/4 + 3^(1/2)*dq1*dqr1*cos(q2)*cos(q3)^2*cos(q5)*sin(q2)*sin(q4)*sin(q5) - 3^(1/2)*dq1*dqr1*cos(q2)^2*cos(q3)*cos(q5)*sin(q3)*sin(q4)*sin(q5) - 2*dq1*dqr1*cos(q2)*cos(q3)*cos(q4)*cos(q5)^2*sin(q2)*sin(q3)*sin(q4) - (5*dq1*dqr1*cos(q2)*cos(q3)*cos(q4)^2*cos(q5)*sin(q2)*sin(q3)*sin(q5))/2;
Y5_19_2=ddqr4/2 + ddqr5 - (dq2*dqr3*sin(2*q4))/4 - (dq2*dqr3*sin(2*q5))/2 + (dq3*dqr3*sin(2*q4))/4 + (dq3*dqr3*sin(2*q5))/2 - (3*dq4*dqr4*sin(2*q5))/8 + (ddqr1*cos(q2)*cos(q3))/2 + (ddqr1*sin(q2)*sin(q3))/2 + (3^(1/2)*ddqr2*cos(q4))/2 - (3^(1/2)*ddqr3*cos(q4))/2 - (3^(1/2)*dq2*dqr4*sin(q4))/2 + (3^(1/2)*dq3*dqr4*sin(q4))/2 + (5*dq2*dqr3*cos(q4)^2*cos(q5)*sin(q5))/4 - (5*dq3*dqr3*cos(q4)^2*cos(q5)*sin(q5))/4 + (3^(1/2)*dq2*dqr4*cos(q5)^2*sin(q4))/2 - (3^(1/2)*dq3*dqr4*cos(q5)^2*sin(q4))/2 - (3^(1/2)*ddqr1*cos(q2)*sin(q3)*sin(q4))/2 + (3^(1/2)*ddqr1*cos(q3)*sin(q2)*sin(q4))/2 - (3^(1/2)*dq1*dqr4*cos(q2)*cos(q4)*sin(q3))/2 + (3^(1/2)*dq1*dqr4*cos(q3)*cos(q4)*sin(q2))/2 + (3^(1/2)*dq2*dqr4*cos(q4)*cos(q5)*sin(q5))/4 - (3^(1/2)*dq3*dqr4*cos(q4)*cos(q5)*sin(q5))/4 - (3^(1/2)*dq4*dqr3*cos(q4)*cos(q5)*sin(q5))/4 - (3*dq1*dqr4*cos(q2)*cos(q3)*cos(q5)*sin(q5))/4 - (3*dq1*dqr4*cos(q5)*sin(q2)*sin(q3)*sin(q5))/4 + (3^(1/2)*dq1*dqr4*cos(q2)*cos(q4)*cos(q5)^2*sin(q3))/2 - (3^(1/2)*dq1*dqr4*cos(q3)*cos(q4)*cos(q5)^2*sin(q2))/2 - (3^(1/2)*dq1*dqr4*cos(q2)*cos(q5)*sin(q3)*sin(q4)*sin(q5))/4 + (3^(1/2)*dq1*dqr4*cos(q3)*cos(q5)*sin(q2)*sin(q4)*sin(q5))/4;
Y5_20_1=(3*dq6*dqr1*sin(q2)*sin(q3)*sin(q5))/4 + (3*dq4*dqr1*cos(q6)^2*sin(q2)*sin(q3)*sin(q5))/16 - (3*dq6*dqr1*cos(q6)^2*sin(q2)*sin(q3)*sin(q5))/4 + (3^(1/2)*dq2*dqr1*sin(q2)*sin(q3)*sin(q4))/2 - (3^(1/2)*dq3*dqr1*sin(q2)*sin(q3)*sin(q4))/2 + (3*dq4*dqr1*cos(q5)*sin(q2)*sin(q3)*sin(q5))/4 + (3*dq4*dqr1*cos(q6)*sin(q2)*sin(q3)*sin(q6))/8 + (3*dq6*dqr1*cos(q6)*sin(q2)*sin(q3)*sin(q6))/8 - (3^(1/2)*dq6*dqr1*cos(q3)*sin(q2)*sin(q4)*sin(q5))/4 - (3^(1/2)*dq2*dqr1*cos(q5)^2*sin(q2)*sin(q3)*sin(q4))/2 - (3^(1/2)*dq2*dqr1*cos(q6)^2*sin(q2)*sin(q3)*sin(q4))/2 + (3^(1/2)*dq3*dqr1*cos(q5)^2*sin(q2)*sin(q3)*sin(q4))/2 + (3^(1/2)*dq3*dqr1*cos(q6)^2*sin(q2)*sin(q3)*sin(q4))/2 + (3*dq4*dqr1*cos(q5)*cos(q6)*sin(q2)*sin(q3)*sin(q6))/8 - (3*dq6*dqr1*cos(q5)*cos(q6)*sin(q2)*sin(q3)*sin(q6))/8 - (15*dq4*dqr1*cos(q5)*cos(q6)^2*sin(q2)*sin(q3)*sin(q5))/16 - (3*dq4*dqr1*cos(q5)^2*cos(q6)*sin(q2)*sin(q3)*sin(q6))/4 - (3^(1/2)*dq1*dqr1*cos(q2)*cos(q6)^2*sin(q2)*sin(q4)*sin(q5))/8 - (3^(1/2)*dq2*dqr1*cos(q4)*cos(q6)^2*sin(q2)*sin(q3)*sin(q5))/16 - (3^(1/2)*dq2*dqr1*cos(q5)*cos(q6)^2*sin(q2)*sin(q3)*sin(q4))/8 + (3^(1/2)*dq3*dqr1*cos(q4)*cos(q6)^2*sin(q2)*sin(q3)*sin(q5))/16 + (3^(1/2)*dq3*dqr1*cos(q5)*cos(q6)^2*sin(q2)*sin(q3)*sin(q4))/8 + (3*3^(1/2)*dq4*dqr1*cos(q3)*cos(q6)^2*sin(q2)*sin(q4)*sin(q5))/16 + (3^(1/2)*dq6*dqr1*cos(q3)*cos(q6)^2*sin(q2)*sin(q4)*sin(q5))/4 - dq1*dqr1*cos(q2)*cos(q3)*cos(q4)*sin(q2)*sin(q3)*sin(q4) + dq1*dqr1*cos(q2)*cos(q3)*cos(q5)*sin(q2)*sin(q3)*sin(q5) + (dq1*dqr1*cos(q2)*cos(q3)*cos(q6)*sin(q2)*sin(q3)*sin(q6))/2 + (5*dq2*dqr1*cos(q3)*cos(q4)*cos(q5)*sin(q2)*sin(q4)*sin(q5))/4 - (5*dq3*dqr1*cos(q3)*cos(q4)*cos(q5)*sin(q2)*sin(q4)*sin(q5))/4 + (5*dq2*dqr1*cos(q3)*cos(q4)*cos(q6)*sin(q2)*sin(q4)*sin(q6))/8 - (5*dq3*dqr1*cos(q3)*cos(q4)*cos(q6)*sin(q2)*sin(q4)*sin(q6))/8 + (dq2*dqr1*cos(q3)*cos(q5)*cos(q6)*sin(q2)*sin(q5)*sin(q6))/2 + (5*3^(1/2)*dq2*dqr1*cos(q5)^2*cos(q6)^2*sin(q2)*sin(q3)*sin(q4))/8 - (5*3^(1/2)*dq3*dqr1*cos(q5)^2*cos(q6)^2*sin(q2)*sin(q3)*sin(q4))/8 + (3*dq1*dqr1*cos(q2)*cos(q3)*cos(q6)^2*sin(q2)*sin(q3)*sin(q5))/4 - (3*dq2*dqr1*cos(q3)*cos(q4)*cos(q6)^2*sin(q2)*sin(q4)*sin(q5))/16 + (3*dq3*dqr1*cos(q3)*cos(q4)*cos(q6)^2*sin(q2)*sin(q4)*sin(q5))/16 - (3*dq2*dqr1*cos(q3)*cos(q4)^2*cos(q6)*sin(q2)*sin(q5)*sin(q6))/4 + (3*dq3*dqr1*cos(q3)*cos(q4)^2*cos(q6)*sin(q2)*sin(q5)*sin(q6))/4 + (3^(1/2)*dq1*dqr1*cos(q2)*cos(q5)*sin(q2)*sin(q4)*sin(q5))/2 + (3^(1/2)*dq1*dqr1*cos(q2)*cos(q6)*sin(q2)*sin(q4)*sin(q6))/4 - (3^(1/2)*dq2*dqr1*cos(q4)*cos(q5)*sin(q2)*sin(q3)*sin(q5))/4 + (3^(1/2)*dq3*dqr1*cos(q4)*cos(q5)*sin(q2)*sin(q3)*sin(q5))/4 - (3^(1/2)*dq2*dqr1*cos(q4)*cos(q6)*sin(q2)*sin(q3)*sin(q6))/8 - (3^(1/2)*dq4*dqr1*cos(q3)*cos(q5)*sin(q2)*sin(q4)*sin(q5))/4 + (3^(1/2)*dq3*dqr1*cos(q4)*cos(q6)*sin(q2)*sin(q3)*sin(q6))/8 - (3^(1/2)*dq4*dqr1*cos(q3)*cos(q6)*sin(q2)*sin(q4)*sin(q6))/8 + (3*3^(1/2)*dq6*dqr1*cos(q3)*cos(q6)*sin(q2)*sin(q4)*sin(q6))/8 - 3^(1/2)*dq1*dqr1*cos(q2)*cos(q3)^2*cos(q5)*sin(q2)*sin(q4)*sin(q5) - (3^(1/2)*dq1*dqr1*cos(q2)*cos(q3)^2*cos(q6)*sin(q2)*sin(q4)*sin(q6))/2 - (5*3^(1/2)*dq1*dqr1*cos(q2)*cos(q5)*cos(q6)^2*sin(q2)*sin(q4)*sin(q5))/8 - (3^(1/2)*dq1*dqr1*cos(q2)*cos(q5)^2*cos(q6)*sin(q2)*sin(q4)*sin(q6))/2 + (5*3^(1/2)*dq2*dqr1*cos(q4)*cos(q5)*cos(q6)^2*sin(q2)*sin(q3)*sin(q5))/16 + (3^(1/2)*dq2*dqr1*cos(q4)*cos(q5)^2*cos(q6)*sin(q2)*sin(q3)*sin(q6))/4 - (5*3^(1/2)*dq3*dqr1*cos(q4)*cos(q5)*cos(q6)^2*sin(q2)*sin(q3)*sin(q5))/16 - (3^(1/2)*dq3*dqr1*cos(q4)*cos(q5)^2*cos(q6)*sin(q2)*sin(q3)*sin(q6))/4 + (5*3^(1/2)*dq4*dqr1*cos(q3)*cos(q5)*cos(q6)^2*sin(q2)*sin(q4)*sin(q5))/16 + (3^(1/2)*dq4*dqr1*cos(q3)*cos(q5)^2*cos(q6)*sin(q2)*sin(q4)*sin(q6))/4 + (3*dq1*dqr1*cos(q2)*cos(q3)*cos(q5)*cos(q6)*sin(q2)*sin(q3)*sin(q6))/2 - (3*dq2*dqr1*cos(q3)*cos(q4)*cos(q5)*cos(q6)*sin(q2)*sin(q4)*sin(q6))/8 + (3*dq3*dqr1*cos(q3)*cos(q4)*cos(q5)*cos(q6)*sin(q2)*sin(q4)*sin(q6))/8 + (3^(1/2)*dq1*dqr1*cos(q2)*cos(q3)^2*cos(q6)^2*sin(q2)*sin(q4)*sin(q5))/4 + 2*dq1*dqr1*cos(q2)*cos(q3)*cos(q4)*cos(q5)^2*sin(q2)*sin(q3)*sin(q4) + (5*dq1*dqr1*cos(q2)*cos(q3)*cos(q4)*cos(q6)^2*sin(q2)*sin(q3)*sin(q4))/4 + (5*dq1*dqr1*cos(q2)*cos(q3)*cos(q4)^2*cos(q5)*sin(q2)*sin(q3)*sin(q5))/2 - (5*dq1*dqr1*cos(q2)*cos(q3)*cos(q5)*cos(q6)^2*sin(q2)*sin(q3)*sin(q5))/4 + (5*dq1*dqr1*cos(q2)*cos(q3)*cos(q4)^2*cos(q6)*sin(q2)*sin(q3)*sin(q6))/4 - dq1*dqr1*cos(q2)*cos(q3)*cos(q5)^2*cos(q6)*sin(q2)*sin(q3)*sin(q6) - (25*dq2*dqr1*cos(q3)*cos(q4)*cos(q5)*cos(q6)^2*sin(q2)*sin(q4)*sin(q5))/16 - (5*dq2*dqr1*cos(q3)*cos(q4)*cos(q5)^2*cos(q6)*sin(q2)*sin(q4)*sin(q6))/4 + (25*dq3*dqr1*cos(q3)*cos(q4)*cos(q5)*cos(q6)^2*sin(q2)*sin(q4)*sin(q5))/16 - dq2*dqr1*cos(q3)*cos(q4)^2*cos(q5)*cos(q6)*sin(q2)*sin(q5)*sin(q6) + (5*dq3*dqr1*cos(q3)*cos(q4)*cos(q5)^2*cos(q6)*sin(q2)*sin(q4)*sin(q6))/4 + dq3*dqr1*cos(q3)*cos(q4)^2*cos(q5)*cos(q6)*sin(q2)*sin(q5)*sin(q6) + (3^(1/2)*dq1*dqr1*cos(q2)*cos(q4)*cos(q6)*sin(q2)*sin(q5)*sin(q6))/4 - (3^(1/2)*dq1*dqr1*cos(q2)*cos(q5)*cos(q6)*sin(q2)*sin(q4)*sin(q6))/4 - (3^(1/2)*dq2*dqr1*cos(q4)*cos(q5)*cos(q6)*sin(q2)*sin(q3)*sin(q6))/8 + (3^(1/2)*dq3*dqr1*cos(q4)*cos(q5)*cos(q6)*sin(q2)*sin(q3)*sin(q6))/8 + (3*3^(1/2)*dq4*dqr1*cos(q3)*cos(q5)*cos(q6)*sin(q2)*sin(q4)*sin(q6))/8 + (3^(1/2)*dq6*dqr1*cos(q3)*cos(q4)*cos(q6)*sin(q2)*sin(q5)*sin(q6))/4 + (3^(1/2)*dq6*dqr1*cos(q3)*cos(q5)*cos(q6)*sin(q2)*sin(q4)*sin(q6))/8 + (3^(1/2)*dq2*dqr1*cos(q6)*sin(q2)*sin(q3)*sin(q4)*sin(q5)*sin(q6))/4 - (3^(1/2)*dq3*dqr1*cos(q6)*sin(q2)*sin(q3)*sin(q4)*sin(q5)*sin(q6))/4 - (3*dq1*dqr1*cos(q2)*cos(q3)*cos(q4)^2*cos(q6)^2*sin(q2)*sin(q3)*sin(q5))/8 + (5*3^(1/2)*dq1*dqr1*cos(q2)*cos(q3)^2*cos(q5)*cos(q6)^2*sin(q2)*sin(q4)*sin(q5))/4 + 3^(1/2)*dq1*dqr1*cos(q2)*cos(q3)^2*cos(q5)^2*cos(q6)*sin(q2)*sin(q4)*sin(q6) - (3*dq1*dqr1*cos(q2)*cos(q3)*cos(q4)*cos(q5)*cos(q6)^2*sin(q2)*sin(q3)*sin(q4))/4 - (3*dq1*dqr1*cos(q2)*cos(q3)*cos(q4)^2*cos(q5)*cos(q6)*sin(q2)*sin(q3)*sin(q6))/4 - 3^(1/2)*dq1*dqr1*cos(q2)*cos(q4)*cos(q5)*cos(q6)*sin(q2)*sin(q5)*sin(q6) + (3^(1/2)*dq4*dqr1*cos(q3)*cos(q4)*cos(q5)*cos(q6)*sin(q2)*sin(q5)*sin(q6))/2 - (3^(1/2)*dq2*dqr1*cos(q5)*cos(q6)*sin(q2)*sin(q3)*sin(q4)*sin(q5)*sin(q6))/2 + (3^(1/2)*dq3*dqr1*cos(q5)*cos(q6)*sin(q2)*sin(q3)*sin(q4)*sin(q5)*sin(q6))/2 - (5*dq1*dqr1*cos(q2)*cos(q3)*cos(q4)*cos(q5)^2*cos(q6)^2*sin(q2)*sin(q3)*sin(q4))/2 - (25*dq1*dqr1*cos(q2)*cos(q3)*cos(q4)^2*cos(q5)*cos(q6)^2*sin(q2)*sin(q3)*sin(q5))/8 - (5*dq1*dqr1*cos(q2)*cos(q3)*cos(q4)^2*cos(q5)^2*cos(q6)*sin(q2)*sin(q3)*sin(q6))/2 - (3^(1/2)*dq1*dqr1*cos(q2)*cos(q3)^2*cos(q4)*cos(q6)*sin(q2)*sin(q5)*sin(q6))/2 + (3^(1/2)*dq1*dqr1*cos(q2)*cos(q3)^2*cos(q5)*cos(q6)*sin(q2)*sin(q4)*sin(q6))/2 + 2*3^(1/2)*dq1*dqr1*cos(q2)*cos(q3)^2*cos(q4)*cos(q5)*cos(q6)*sin(q2)*sin(q5)*sin(q6) + (3*dq1*dqr1*cos(q2)*cos(q3)*cos(q4)*cos(q6)*sin(q2)*sin(q3)*sin(q4)*sin(q5)*sin(q6))/2 + 2*dq1*dqr1*cos(q2)*cos(q3)*cos(q4)*cos(q5)*cos(q6)*sin(q2)*sin(q3)*sin(q4)*sin(q5)*sin(q6);
Y5_20_2=(dq3*dqr1*cos(q3)*sin(q2))/2 - (dq2*dqr1*cos(q3)*sin(q2))/2 - (dq2*dqr1*cos(q2)*cos(q4)^2*sin(q3))/2 + (dq2*dqr1*cos(q3)*cos(q4)^2*sin(q2))/2 + (dq2*dqr1*cos(q3)*cos(q5)^2*sin(q2))/2 - (dq3*dqr1*cos(q3)*cos(q4)^2*sin(q2))/2 + (dq2*dqr1*cos(q3)*cos(q6)^2*sin(q2))/2 - (dq3*dqr1*cos(q3)*cos(q5)^2*sin(q2))/2 - (dq3*dqr1*cos(q3)*cos(q6)^2*sin(q2))/2 + (3^(1/2)*dq1*dqr1*cos(q2)*cos(q4)*sin(q2))/2 + dq2*dqr1*cos(q2)*cos(q4)^2*cos(q5)^2*sin(q3) - dq2*dqr1*cos(q3)*cos(q4)^2*cos(q5)^2*sin(q2) + (5*dq2*dqr1*cos(q2)*cos(q4)^2*cos(q6)^2*sin(q3))/8 - (5*dq2*dqr1*cos(q3)*cos(q4)^2*cos(q6)^2*sin(q2))/8 - dq3*dqr1*cos(q2)*cos(q4)^2*cos(q5)^2*sin(q3) + dq3*dqr1*cos(q3)*cos(q4)^2*cos(q5)^2*sin(q2) - (5*dq2*dqr1*cos(q3)*cos(q5)^2*cos(q6)^2*sin(q2))/8 - (5*dq3*dqr1*cos(q2)*cos(q4)^2*cos(q6)^2*sin(q3))/8 + (5*dq3*dqr1*cos(q3)*cos(q4)^2*cos(q6)^2*sin(q2))/8 + (5*dq3*dqr1*cos(q3)*cos(q5)^2*cos(q6)^2*sin(q2))/8 - (3*dq2*dqr1*cos(q3)*cos(q5)*cos(q6)^2*sin(q2))/8 + (3*dq3*dqr1*cos(q3)*cos(q5)*cos(q6)^2*sin(q2))/8 + (3^(1/2)*dq6*dqr1*cos(q2)*sin(q3)*sin(q4)*sin(q5))/4 - (3*dq2*dqr1*cos(q2)*cos(q4)^2*cos(q5)*cos(q6)^2*sin(q3))/8 + (3*dq2*dqr1*cos(q3)*cos(q4)^2*cos(q5)*cos(q6)^2*sin(q2))/8 + (3*dq3*dqr1*cos(q2)*cos(q4)^2*cos(q5)*cos(q6)^2*sin(q3))/8 - (3*dq3*dqr1*cos(q3)*cos(q4)^2*cos(q5)*cos(q6)^2*sin(q2))/8 - 3^(1/2)*dq1*dqr1*cos(q2)*cos(q3)^2*cos(q4)*sin(q2) + 3^(1/2)*dq1*dqr1*cos(q2)^2*cos(q3)*cos(q4)*sin(q3) - 3^(1/2)*dq1*dqr1*cos(q2)*cos(q4)*cos(q5)^2*sin(q2) - (5*3^(1/2)*dq1*dqr1*cos(q2)*cos(q4)*cos(q6)^2*sin(q2))/8 + (3^(1/2)*dq4*dqr1*cos(q3)*cos(q4)*cos(q5)^2*sin(q2))/2 + (3^(1/2)*dq4*dqr1*cos(q3)*cos(q4)*cos(q6)^2*sin(q2))/8 - (5*dq2*dqr1*cos(q2)*cos(q4)^2*cos(q5)^2*cos(q6)^2*sin(q3))/4 + (5*dq2*dqr1*cos(q3)*cos(q4)^2*cos(q5)^2*cos(q6)^2*sin(q2))/4 + (5*dq3*dqr1*cos(q2)*cos(q4)^2*cos(q5)^2*cos(q6)^2*sin(q3))/4 - (5*dq3*dqr1*cos(q3)*cos(q4)^2*cos(q5)^2*cos(q6)^2*sin(q2))/4 - (3*dq2*dqr1*cos(q2)*cos(q6)*sin(q3)*sin(q5)*sin(q6))/4 + (3*dq2*dqr1*cos(q3)*cos(q6)*sin(q2)*sin(q5)*sin(q6))/4 + (3*dq3*dqr1*cos(q2)*cos(q6)*sin(q3)*sin(q5)*sin(q6))/4 - (3*dq3*dqr1*cos(q3)*cos(q6)*sin(q2)*sin(q5)*sin(q6))/4 + (3^(1/2)*dq6*dqr1*cos(q3)*cos(q4)*cos(q5)*sin(q2))/2 - (3^(1/2)*dq1*dqr1*cos(q2)*cos(q4)*cos(q5)*cos(q6)^2*sin(q2))/8 - (3^(1/2)*dq6*dqr1*cos(q3)*cos(q4)*cos(q5)*cos(q6)^2*sin(q2))/2 + (3^(1/2)*dq1*dqr1*cos(q3)*cos(q6)^2*sin(q3)*sin(q4)*sin(q5))/8 - (3*3^(1/2)*dq4*dqr1*cos(q2)*cos(q6)^2*sin(q3)*sin(q4)*sin(q5))/16 - (3^(1/2)*dq6*dqr1*cos(q2)*cos(q6)^2*sin(q3)*sin(q4)*sin(q5))/4 - (5*dq2*dqr1*cos(q2)*cos(q4)*cos(q5)*sin(q3)*sin(q4)*sin(q5))/4 + (5*dq3*dqr1*cos(q2)*cos(q4)*cos(q5)*sin(q3)*sin(q4)*sin(q5))/4 - (5*dq2*dqr1*cos(q2)*cos(q4)*cos(q6)*sin(q3)*sin(q4)*sin(q6))/8 + (5*dq3*dqr1*cos(q2)*cos(q4)*cos(q6)*sin(q3)*sin(q4)*sin(q6))/8 - (dq2*dqr1*cos(q2)*cos(q5)*cos(q6)*sin(q3)*sin(q5)*sin(q6))/2 + (dq3*dqr1*cos(q2)*cos(q5)*cos(q6)*sin(q3)*sin(q5)*sin(q6))/2 - (dq3*dqr1*cos(q3)*cos(q5)*cos(q6)*sin(q2)*sin(q5)*sin(q6))/2 + 2*3^(1/2)*dq1*dqr1*cos(q2)*cos(q3)^2*cos(q4)*cos(q5)^2*sin(q2) + (5*3^(1/2)*dq1*dqr1*cos(q2)*cos(q3)^2*cos(q4)*cos(q6)^2*sin(q2))/4 - 2*3^(1/2)*dq1*dqr1*cos(q2)^2*cos(q3)*cos(q4)*cos(q5)^2*sin(q3) - (5*3^(1/2)*dq1*dqr1*cos(q2)^2*cos(q3)*cos(q4)*cos(q6)^2*sin(q3))/4 + (5*3^(1/2)*dq1*dqr1*cos(q2)*cos(q4)*cos(q5)^2*cos(q6)^2*sin(q2))/4 - (5*3^(1/2)*dq4*dqr1*cos(q3)*cos(q4)*cos(q5)^2*cos(q6)^2*sin(q2))/8 + (3*dq2*dqr1*cos(q2)*cos(q4)*cos(q6)^2*sin(q3)*sin(q4)*sin(q5))/16 - (3*dq3*dqr1*cos(q2)*cos(q4)*cos(q6)^2*sin(q3)*sin(q4)*sin(q5))/16 + (3*dq2*dqr1*cos(q2)*cos(q4)^2*cos(q6)*sin(q3)*sin(q5)*sin(q6))/4 - (3*dq3*dqr1*cos(q2)*cos(q4)^2*cos(q6)*sin(q3)*sin(q5)*sin(q6))/4 - (3^(1/2)*dq1*dqr1*cos(q3)*cos(q5)*sin(q3)*sin(q4)*sin(q5))/2 - (3^(1/2)*dq1*dqr1*cos(q3)*cos(q6)*sin(q3)*sin(q4)*sin(q6))/4 + (3^(1/2)*dq4*dqr1*cos(q2)*cos(q5)*sin(q3)*sin(q4)*sin(q5))/4 + (3^(1/2)*dq4*dqr1*cos(q2)*cos(q6)*sin(q3)*sin(q4)*sin(q6))/8 - (3*3^(1/2)*dq6*dqr1*cos(q2)*cos(q6)*sin(q3)*sin(q4)*sin(q6))/8 + 3^(1/2)*dq1*dqr1*cos(q2)^2*cos(q3)*cos(q5)*sin(q3)*sin(q4)*sin(q5) + (3^(1/2)*dq1*dqr1*cos(q2)^2*cos(q3)*cos(q6)*sin(q3)*sin(q4)*sin(q6))/2 + (5*3^(1/2)*dq1*dqr1*cos(q3)*cos(q5)*cos(q6)^2*sin(q3)*sin(q4)*sin(q5))/8 + (3^(1/2)*dq1*dqr1*cos(q3)*cos(q5)^2*cos(q6)*sin(q3)*sin(q4)*sin(q6))/2 - (5*3^(1/2)*dq4*dqr1*cos(q2)*cos(q5)*cos(q6)^2*sin(q3)*sin(q4)*sin(q5))/16 - (3^(1/2)*dq4*dqr1*cos(q2)*cos(q5)^2*cos(q6)*sin(q3)*sin(q4)*sin(q6))/4 + (3*dq2*dqr1*cos(q2)*cos(q4)*cos(q5)*cos(q6)*sin(q3)*sin(q4)*sin(q6))/8 - (3*dq3*dqr1*cos(q2)*cos(q4)*cos(q5)*cos(q6)*sin(q3)*sin(q4)*sin(q6))/8 + (3^(1/2)*dq1*dqr1*cos(q2)*cos(q3)^2*cos(q4)*cos(q5)*cos(q6)^2*sin(q2))/4 - (3^(1/2)*dq1*dqr1*cos(q2)^2*cos(q3)*cos(q4)*cos(q5)*cos(q6)^2*sin(q3))/4 - (3^(1/2)*dq1*dqr1*cos(q2)^2*cos(q3)*cos(q6)^2*sin(q3)*sin(q4)*sin(q5))/4 + (25*dq2*dqr1*cos(q2)*cos(q4)*cos(q5)*cos(q6)^2*sin(q3)*sin(q4)*sin(q5))/16 + (5*dq2*dqr1*cos(q2)*cos(q4)*cos(q5)^2*cos(q6)*sin(q3)*sin(q4)*sin(q6))/4 - (25*dq3*dqr1*cos(q2)*cos(q4)*cos(q5)*cos(q6)^2*sin(q3)*sin(q4)*sin(q5))/16 + dq2*dqr1*cos(q2)*cos(q4)^2*cos(q5)*cos(q6)*sin(q3)*sin(q5)*sin(q6) - (5*dq3*dqr1*cos(q2)*cos(q4)*cos(q5)^2*cos(q6)*sin(q3)*sin(q4)*sin(q6))/4 - dq3*dqr1*cos(q2)*cos(q4)^2*cos(q5)*cos(q6)*sin(q3)*sin(q5)*sin(q6) - (5*3^(1/2)*dq1*dqr1*cos(q2)*cos(q3)^2*cos(q4)*cos(q5)^2*cos(q6)^2*sin(q2))/2 + (5*3^(1/2)*dq1*dqr1*cos(q2)^2*cos(q3)*cos(q4)*cos(q5)^2*cos(q6)^2*sin(q3))/2 - (3^(1/2)*dq1*dqr1*cos(q3)*cos(q4)*cos(q6)*sin(q3)*sin(q5)*sin(q6))/4 + (3^(1/2)*dq1*dqr1*cos(q3)*cos(q5)*cos(q6)*sin(q3)*sin(q4)*sin(q6))/4 - (3*3^(1/2)*dq4*dqr1*cos(q2)*cos(q5)*cos(q6)*sin(q3)*sin(q4)*sin(q6))/8 - (3^(1/2)*dq6*dqr1*cos(q2)*cos(q4)*cos(q6)*sin(q3)*sin(q5)*sin(q6))/4 - (3^(1/2)*dq6*dqr1*cos(q2)*cos(q5)*cos(q6)*sin(q3)*sin(q4)*sin(q6))/8 - (5*3^(1/2)*dq1*dqr1*cos(q2)^2*cos(q3)*cos(q5)*cos(q6)^2*sin(q3)*sin(q4)*sin(q5))/4 - 3^(1/2)*dq1*dqr1*cos(q2)^2*cos(q3)*cos(q5)^2*cos(q6)*sin(q3)*sin(q4)*sin(q6) + 3^(1/2)*dq1*dqr1*cos(q3)*cos(q4)*cos(q5)*cos(q6)*sin(q3)*sin(q5)*sin(q6) - (3^(1/2)*dq4*dqr1*cos(q2)*cos(q4)*cos(q5)*cos(q6)*sin(q3)*sin(q5)*sin(q6))/2 + (3^(1/2)*dq1*dqr1*cos(q2)^2*cos(q3)*cos(q4)*cos(q6)*sin(q3)*sin(q5)*sin(q6))/2 - (3^(1/2)*dq1*dqr1*cos(q2)^2*cos(q3)*cos(q5)*cos(q6)*sin(q3)*sin(q4)*sin(q6))/2 - 2*3^(1/2)*dq1*dqr1*cos(q2)^2*cos(q3)*cos(q4)*cos(q5)*cos(q6)*sin(q3)*sin(q5)*sin(q6);
Y5_20_3=(3*dq1*dqr1*cos(q6)^2*sin(q5))/16 + (dq2*dqr1*cos(q2)*sin(q3))/2 - (dq3*dqr1*cos(q2)*sin(q3))/2 + (dq1*dqr1*cos(q2)^2*cos(q4)*sin(q4))/2 + (dq1*dqr1*cos(q3)^2*cos(q4)*sin(q4))/2 - (dq2*dqr1*cos(q2)*cos(q5)^2*sin(q3))/2 + (dq3*dqr1*cos(q2)*cos(q4)^2*sin(q3))/2 - (dq1*dqr1*cos(q2)^2*cos(q5)*sin(q5))/2 - (dq2*dqr1*cos(q2)*cos(q6)^2*sin(q3))/2 + (dq3*dqr1*cos(q2)*cos(q5)^2*sin(q3))/2 - (dq1*dqr1*cos(q3)^2*cos(q5)*sin(q5))/2 + (dq3*dqr1*cos(q2)*cos(q6)^2*sin(q3))/2 - (dq1*dqr1*cos(q2)^2*cos(q6)*sin(q6))/4 - (15*dq1*dqr1*cos(q5)*cos(q6)^2*sin(q5))/16 - (3*dq1*dqr1*cos(q2)^2*cos(q6)^2*sin(q5))/8 - (3*dq1*dqr1*cos(q3)^2*cos(q6)^2*sin(q5))/8 + (3*dq6*dqr1*cos(q2)*cos(q3)*sin(q5))/4 - (3^(1/2)*dq1*dqr1*cos(q3)*cos(q4)*sin(q3))/2 + (3^(1/2)*dq2*dqr1*cos(q2)*cos(q3)*sin(q4))/2 - (3^(1/2)*dq3*dqr1*cos(q2)*cos(q3)*sin(q4))/2 - dq1*dqr1*cos(q2)^2*cos(q3)^2*cos(q4)*sin(q4) - dq1*dqr1*cos(q2)^2*cos(q4)*cos(q5)^2*sin(q4) + dq1*dqr1*cos(q2)^2*cos(q3)^2*cos(q5)*sin(q5) - (5*dq1*dqr1*cos(q2)^2*cos(q4)*cos(q6)^2*sin(q4))/8 - (5*dq1*dqr1*cos(q2)^2*cos(q4)^2*cos(q5)*sin(q5))/4 - dq1*dqr1*cos(q3)^2*cos(q4)*cos(q5)^2*sin(q4) + (dq1*dqr1*cos(q2)^2*cos(q3)^2*cos(q6)*sin(q6))/2 - (5*dq1*dqr1*cos(q3)^2*cos(q4)*cos(q6)^2*sin(q4))/8 - (5*dq1*dqr1*cos(q3)^2*cos(q4)^2*cos(q5)*sin(q5))/4 + (5*dq2*dqr1*cos(q2)*cos(q5)^2*cos(q6)^2*sin(q3))/8 + (5*dq1*dqr1*cos(q2)^2*cos(q5)*cos(q6)^2*sin(q5))/8 - (5*dq1*dqr1*cos(q2)^2*cos(q4)^2*cos(q6)*sin(q6))/8 - (5*dq3*dqr1*cos(q2)*cos(q5)^2*cos(q6)^2*sin(q3))/8 + (dq1*dqr1*cos(q2)^2*cos(q5)^2*cos(q6)*sin(q6))/2 + (5*dq1*dqr1*cos(q3)^2*cos(q5)*cos(q6)^2*sin(q5))/8 + (3*dq4*dqr1*cos(q2)*cos(q3)*cos(q5)*sin(q5))/4 + (3*dq1*dqr1*cos(q2)^2*cos(q3)^2*cos(q6)^2*sin(q5))/4 + (3*dq1*dqr1*cos(q2)^2*cos(q4)^2*cos(q6)^2*sin(q5))/16 + (3*dq1*dqr1*cos(q3)^2*cos(q4)^2*cos(q6)^2*sin(q5))/16 + (3*dq2*dqr1*cos(q2)*cos(q5)*cos(q6)^2*sin(q3))/8 - (3*dq3*dqr1*cos(q2)*cos(q5)*cos(q6)^2*sin(q3))/8 - (3*dq1*dqr1*cos(q2)^2*cos(q5)*cos(q6)*sin(q6))/4 + (3*dq4*dqr1*cos(q2)*cos(q3)*cos(q6)^2*sin(q5))/16 - (3*dq6*dqr1*cos(q2)*cos(q3)*cos(q6)^2*sin(q5))/4 + (3*dq1*dqr1*cos(q2)^2*cos(q4)*cos(q5)*cos(q6)^2*sin(q4))/8 + (3*dq1*dqr1*cos(q2)^2*cos(q3)^2*cos(q5)*cos(q6)*sin(q6))/2 + (3*dq1*dqr1*cos(q3)^2*cos(q4)*cos(q5)*cos(q6)^2*sin(q4))/8 + (3*dq1*dqr1*cos(q2)^2*cos(q4)^2*cos(q5)*cos(q6)*sin(q6))/8 + 3^(1/2)*dq1*dqr1*cos(q3)*cos(q4)*cos(q5)^2*sin(q3) - (3^(1/2)*dq2*dqr1*cos(q2)*cos(q3)*cos(q5)^2*sin(q4))/2 + (5*3^(1/2)*dq1*dqr1*cos(q3)*cos(q4)*cos(q6)^2*sin(q3))/8 - (3^(1/2)*dq2*dqr1*cos(q2)*cos(q3)*cos(q6)^2*sin(q4))/2 + (3^(1/2)*dq3*dqr1*cos(q2)*cos(q3)*cos(q5)^2*sin(q4))/2 + (3^(1/2)*dq3*dqr1*cos(q2)*cos(q3)*cos(q6)^2*sin(q4))/2 - (3^(1/2)*dq4*dqr1*cos(q2)*cos(q4)*cos(q5)^2*sin(q3))/2 - (3^(1/2)*dq4*dqr1*cos(q2)*cos(q4)*cos(q6)^2*sin(q3))/8 + 2*dq1*dqr1*cos(q2)^2*cos(q3)^2*cos(q4)*cos(q5)^2*sin(q4) + (5*dq1*dqr1*cos(q2)^2*cos(q3)^2*cos(q4)*cos(q6)^2*sin(q4))/4 + (5*dq1*dqr1*cos(q2)^2*cos(q3)^2*cos(q4)^2*cos(q5)*sin(q5))/2 + (5*dq1*dqr1*cos(q2)^2*cos(q4)*cos(q5)^2*cos(q6)^2*sin(q4))/4 - (5*dq1*dqr1*cos(q2)^2*cos(q3)^2*cos(q5)*cos(q6)^2*sin(q5))/4 + (5*dq1*dqr1*cos(q2)^2*cos(q3)^2*cos(q4)^2*cos(q6)*sin(q6))/4 - dq1*dqr1*cos(q2)^2*cos(q3)^2*cos(q5)^2*cos(q6)*sin(q6) + (25*dq1*dqr1*cos(q2)^2*cos(q4)^2*cos(q5)*cos(q6)^2*sin(q5))/16 + (5*dq1*dqr1*cos(q3)^2*cos(q4)*cos(q5)^2*cos(q6)^2*sin(q4))/4 + (5*dq1*dqr1*cos(q2)^2*cos(q4)^2*cos(q5)^2*cos(q6)*sin(q6))/4 + (25*dq1*dqr1*cos(q3)^2*cos(q4)^2*cos(q5)*cos(q6)^2*sin(q5))/16 - (15*dq4*dqr1*cos(q2)*cos(q3)*cos(q5)*cos(q6)^2*sin(q5))/16 - (3*dq1*dqr1*cos(q2)^2*cos(q3)^2*cos(q4)^2*cos(q6)^2*sin(q5))/8 - (3^(1/2)*dq6*dqr1*cos(q2)*cos(q4)*cos(q5)*sin(q3))/2 + (3^(1/2)*dq1*dqr1*cos(q3)*cos(q4)*cos(q5)*cos(q6)^2*sin(q3))/8 - (3^(1/2)*dq2*dqr1*cos(q2)*cos(q3)*cos(q4)*cos(q6)^2*sin(q5))/16 - (3^(1/2)*dq2*dqr1*cos(q2)*cos(q3)*cos(q5)*cos(q6)^2*sin(q4))/8 + (3^(1/2)*dq3*dqr1*cos(q2)*cos(q3)*cos(q4)*cos(q6)^2*sin(q5))/16 + (3^(1/2)*dq3*dqr1*cos(q2)*cos(q3)*cos(q5)*cos(q6)^2*sin(q4))/8 + (3^(1/2)*dq6*dqr1*cos(q2)*cos(q4)*cos(q5)*cos(q6)^2*sin(q3))/2 - (3*dq1*dqr1*cos(q2)^2*cos(q3)^2*cos(q4)*cos(q5)*cos(q6)^2*sin(q4))/4 - (3*dq1*dqr1*cos(q2)^2*cos(q3)^2*cos(q4)^2*cos(q5)*cos(q6)*sin(q6))/4 - (5*3^(1/2)*dq1*dqr1*cos(q3)*cos(q4)*cos(q5)^2*cos(q6)^2*sin(q3))/4 + (5*3^(1/2)*dq2*dqr1*cos(q2)*cos(q3)*cos(q5)^2*cos(q6)^2*sin(q4))/8 - (5*3^(1/2)*dq3*dqr1*cos(q2)*cos(q3)*cos(q5)^2*cos(q6)^2*sin(q4))/8 + (5*3^(1/2)*dq4*dqr1*cos(q2)*cos(q4)*cos(q5)^2*cos(q6)^2*sin(q3))/8 - (5*dq1*dqr1*cos(q2)^2*cos(q3)^2*cos(q4)*cos(q5)^2*cos(q6)^2*sin(q4))/2 - (25*dq1*dqr1*cos(q2)^2*cos(q3)^2*cos(q4)^2*cos(q5)*cos(q6)^2*sin(q5))/8 - (5*dq1*dqr1*cos(q2)^2*cos(q3)^2*cos(q4)^2*cos(q5)^2*cos(q6)*sin(q6))/2 - (3*dq1*dqr1*cos(q2)^2*cos(q4)*cos(q6)*sin(q4)*sin(q5)*sin(q6))/4 - (3*dq1*dqr1*cos(q3)^2*cos(q4)*cos(q6)*sin(q4)*sin(q5)*sin(q6))/4 - (3^(1/2)*dq2*dqr1*cos(q2)*cos(q3)*cos(q4)*cos(q5)*sin(q5))/4 + (3^(1/2)*dq3*dqr1*cos(q2)*cos(q3)*cos(q4)*cos(q5)*sin(q5))/4 - dq1*dqr1*cos(q2)^2*cos(q4)*cos(q5)*cos(q6)*sin(q4)*sin(q5)*sin(q6) - dq1*dqr1*cos(q3)^2*cos(q4)*cos(q5)*cos(q6)*sin(q4)*sin(q5)*sin(q6) + (3^(1/2)*dq2*dqr1*cos(q2)*cos(q3)*cos(q6)*sin(q4)*sin(q5)*sin(q6))/4 - (3^(1/2)*dq3*dqr1*cos(q2)*cos(q3)*cos(q6)*sin(q4)*sin(q5)*sin(q6))/4 + (3*dq1*dqr1*cos(q2)^2*cos(q3)^2*cos(q4)*cos(q6)*sin(q4)*sin(q5)*sin(q6))/2 + (5*3^(1/2)*dq2*dqr1*cos(q2)*cos(q3)*cos(q4)*cos(q5)*cos(q6)^2*sin(q5))/16 + (3^(1/2)*dq2*dqr1*cos(q2)*cos(q3)*cos(q4)*cos(q5)^2*cos(q6)*sin(q6))/4 - (5*3^(1/2)*dq3*dqr1*cos(q2)*cos(q3)*cos(q4)*cos(q5)*cos(q6)^2*sin(q5))/16 - (3^(1/2)*dq2*dqr1*cos(q2)*cos(q3)*cos(q5)*cos(q6)*sin(q4)*sin(q5)*sin(q6))/2 + (3^(1/2)*dq3*dqr1*cos(q2)*cos(q3)*cos(q5)*cos(q6)*sin(q4)*sin(q5)*sin(q6))/2 + 2*dq1*dqr1*cos(q2)^2*cos(q3)^2*cos(q4)*cos(q5)*cos(q6)*sin(q4)*sin(q5)*sin(q6);
Y5_20_4=(3*dq1*dqr1*sin(2*q5))/8 + (3*dq1*dqr1*sin(2*q6))/16 + (dq1*dqr2*cos(q2)*sin(q3))/2 - (dq1*dqr2*cos(q3)*sin(q2))/2 - (dq1*dqr2*cos(q2)*cos(q4)^2*sin(q3))/2 + (dq1*dqr2*cos(q3)*cos(q4)^2*sin(q2))/2 - (dq1*dqr2*cos(q2)*cos(q5)^2*sin(q3))/2 + (dq1*dqr2*cos(q3)*cos(q5)^2*sin(q2))/2 - (dq1*dqr2*cos(q2)*cos(q6)^2*sin(q3))/2 + (dq1*dqr2*cos(q3)*cos(q6)^2*sin(q2))/2 - (dq1*dqr1*cos(q3)^2*cos(q6)*sin(q6))/4 + dq2*dqr2*cos(q4)*cos(q5)^2*sin(q4) + (5*dq2*dqr2*cos(q4)*cos(q6)^2*sin(q4))/8 - dq3*dqr2*cos(q4)*cos(q5)^2*sin(q4) - (3*dq1*dqr1*cos(q5)^2*cos(q6)*sin(q6))/4 - (5*dq3*dqr2*cos(q4)*cos(q6)^2*sin(q4))/8 - (3^(1/2)*dq6*dqr2*cos(q5)*sin(q4))/2 - (3^(1/2)*dq4*dqr2*cos(q5)^2*sin(q4))/2 - (3^(1/2)*dq4*dqr2*cos(q6)^2*sin(q4))/8 + (3*dq1*dqr1*cos(q5)*cos(q6)*sin(q6))/8 + (3^(1/2)*dq1*dqr2*cos(q2)*cos(q3)*sin(q4))/2 + (3^(1/2)*dq1*dqr2*sin(q2)*sin(q3)*sin(q4))/2 + dq1*dqr2*cos(q2)*cos(q4)^2*cos(q5)^2*sin(q3) - dq1*dqr2*cos(q3)*cos(q4)^2*cos(q5)^2*sin(q2) + (5*dq1*dqr2*cos(q2)*cos(q4)^2*cos(q6)^2*sin(q3))/8 - (5*dq1*dqr2*cos(q3)*cos(q4)^2*cos(q6)^2*sin(q2))/8 + (5*dq1*dqr2*cos(q2)*cos(q5)^2*cos(q6)^2*sin(q3))/8 - (5*dq1*dqr2*cos(q3)*cos(q5)^2*cos(q6)^2*sin(q2))/8 - (5*dq1*dqr1*cos(q3)^2*cos(q4)^2*cos(q6)*sin(q6))/8 + (dq1*dqr1*cos(q3)^2*cos(q5)^2*cos(q6)*sin(q6))/2 - (5*dq2*dqr2*cos(q4)*cos(q5)^2*cos(q6)^2*sin(q4))/4 + (5*dq3*dqr2*cos(q4)*cos(q5)^2*cos(q6)^2*sin(q4))/4 + (3^(1/2)*dq6*dqr2*cos(q5)*cos(q6)^2*sin(q4))/2 + (3*dq4*dqr1*cos(q2)*cos(q3)*cos(q6)*sin(q6))/8 + (3*dq6*dqr1*cos(q2)*cos(q3)*cos(q6)*sin(q6))/8 + (5*3^(1/2)*dq4*dqr2*cos(q5)^2*cos(q6)^2*sin(q4))/8 + (3*dq1*dqr2*cos(q2)*cos(q5)*cos(q6)^2*sin(q3))/8 - (3*dq1*dqr2*cos(q3)*cos(q5)*cos(q6)^2*sin(q2))/8 - (3*dq1*dqr1*cos(q3)^2*cos(q5)*cos(q6)*sin(q6))/4 - (3*dq2*dqr2*cos(q4)*cos(q5)*cos(q6)^2*sin(q4))/8 + (3*dq3*dqr2*cos(q4)*cos(q5)*cos(q6)^2*sin(q4))/8 - (3^(1/2)*dq6*dqr2*cos(q6)*sin(q4)*sin(q5)*sin(q6))/4 - (3*dq1*dqr2*cos(q2)*cos(q4)^2*cos(q5)*cos(q6)^2*sin(q3))/8 + (3*dq1*dqr2*cos(q3)*cos(q4)^2*cos(q5)*cos(q6)^2*sin(q2))/8 + (3*dq1*dqr1*cos(q3)^2*cos(q4)^2*cos(q5)*cos(q6)*sin(q6))/8 - (3^(1/2)*dq1*dqr2*cos(q2)*cos(q3)*cos(q5)^2*sin(q4))/2 - (3^(1/2)*dq1*dqr2*cos(q2)*cos(q3)*cos(q6)^2*sin(q4))/2 + (3*dq4*dqr1*cos(q2)*cos(q3)*cos(q5)*cos(q6)*sin(q6))/8 - (3*dq6*dqr1*cos(q2)*cos(q3)*cos(q5)*cos(q6)*sin(q6))/8 - (3^(1/2)*dq1*dqr2*cos(q5)^2*sin(q2)*sin(q3)*sin(q4))/2 - (3^(1/2)*dq1*dqr2*cos(q6)^2*sin(q2)*sin(q3)*sin(q4))/2 - (5*dq1*dqr2*cos(q2)*cos(q4)^2*cos(q5)^2*cos(q6)^2*sin(q3))/4 + (5*dq1*dqr2*cos(q3)*cos(q4)^2*cos(q5)^2*cos(q6)^2*sin(q2))/4 + (5*dq1*dqr1*cos(q3)^2*cos(q4)^2*cos(q5)^2*cos(q6)*sin(q6))/4 - (3*dq1*dqr2*cos(q2)*cos(q6)*sin(q3)*sin(q5)*sin(q6))/4 + (3*dq1*dqr2*cos(q3)*cos(q6)*sin(q2)*sin(q5)*sin(q6))/4 + (3*dq2*dqr2*cos(q4)*cos(q6)*sin(q4)*sin(q5)*sin(q6))/4 - (3*dq3*dqr2*cos(q4)*cos(q6)*sin(q4)*sin(q5)*sin(q6))/4 - (3*dq4*dqr1*cos(q2)*cos(q3)*cos(q5)^2*cos(q6)*sin(q6))/4 - (3^(1/2)*dq1*dqr2*cos(q2)*cos(q3)*cos(q5)*cos(q6)^2*sin(q4))/8 - (3^(1/2)*dq1*dqr2*cos(q4)*cos(q6)^2*sin(q2)*sin(q3)*sin(q5))/16 - (3^(1/2)*dq1*dqr2*cos(q5)*cos(q6)^2*sin(q2)*sin(q3)*sin(q4))/8 - (5*dq1*dqr2*cos(q2)*cos(q4)*cos(q5)*sin(q3)*sin(q4)*sin(q5))/4 + (5*dq1*dqr2*cos(q3)*cos(q4)*cos(q5)*sin(q2)*sin(q4)*sin(q5))/4 - (5*dq1*dqr2*cos(q2)*cos(q4)*cos(q6)*sin(q3)*sin(q4)*sin(q6))/8 + (5*dq1*dqr2*cos(q3)*cos(q4)*cos(q6)*sin(q2)*sin(q4)*sin(q6))/8 - (dq1*dqr2*cos(q2)*cos(q5)*cos(q6)*sin(q3)*sin(q5)*sin(q6))/2 + (dq1*dqr2*cos(q3)*cos(q5)*cos(q6)*sin(q2)*sin(q5)*sin(q6))/2 + dq2*dqr2*cos(q4)*cos(q5)*cos(q6)*sin(q4)*sin(q5)*sin(q6) - dq3*dqr2*cos(q4)*cos(q5)*cos(q6)*sin(q4)*sin(q5)*sin(q6) + (5*3^(1/2)*dq1*dqr2*cos(q2)*cos(q3)*cos(q5)^2*cos(q6)^2*sin(q4))/8 + (5*3^(1/2)*dq1*dqr2*cos(q5)^2*cos(q6)^2*sin(q2)*sin(q3)*sin(q4))/8 + (3*dq1*dqr2*cos(q2)*cos(q4)*cos(q6)^2*sin(q3)*sin(q4)*sin(q5))/16 - (3*dq1*dqr2*cos(q3)*cos(q4)*cos(q6)^2*sin(q2)*sin(q4)*sin(q5))/16 + (3*dq1*dqr2*cos(q2)*cos(q4)^2*cos(q6)*sin(q3)*sin(q5)*sin(q6))/4 - (3*dq1*dqr2*cos(q3)*cos(q4)^2*cos(q6)*sin(q2)*sin(q5)*sin(q6))/4 - (3^(1/2)*dq2*dqr1*cos(q2)*cos(q3)*cos(q4)*cos(q6)*sin(q6))/8 + (3^(1/2)*dq3*dqr1*cos(q2)*cos(q3)*cos(q4)*cos(q6)*sin(q6))/8 - (3^(1/2)*dq1*dqr2*cos(q4)*cos(q5)*sin(q2)*sin(q3)*sin(q5))/4 - (3^(1/2)*dq1*dqr2*cos(q4)*cos(q6)*sin(q2)*sin(q3)*sin(q6))/8 - (3^(1/2)*dq4*dqr2*cos(q5)*cos(q6)*sin(q4)*sin(q5)*sin(q6))/2 + (5*3^(1/2)*dq1*dqr2*cos(q4)*cos(q5)*cos(q6)^2*sin(q2)*sin(q3)*sin(q5))/16 + (3^(1/2)*dq1*dqr2*cos(q4)*cos(q5)^2*cos(q6)*sin(q2)*sin(q3)*sin(q6))/4 + (3*dq1*dqr2*cos(q2)*cos(q4)*cos(q5)*cos(q6)*sin(q3)*sin(q4)*sin(q6))/8 - (3*dq1*dqr2*cos(q3)*cos(q4)*cos(q5)*cos(q6)*sin(q2)*sin(q4)*sin(q6))/8 + (25*dq1*dqr2*cos(q2)*cos(q4)*cos(q5)*cos(q6)^2*sin(q3)*sin(q4)*sin(q5))/16 - (25*dq1*dqr2*cos(q3)*cos(q4)*cos(q5)*cos(q6)^2*sin(q2)*sin(q4)*sin(q5))/16 + (5*dq1*dqr2*cos(q2)*cos(q4)*cos(q5)^2*cos(q6)*sin(q3)*sin(q4)*sin(q6))/4 - (5*dq1*dqr2*cos(q3)*cos(q4)*cos(q5)^2*cos(q6)*sin(q2)*sin(q4)*sin(q6))/4 + dq1*dqr2*cos(q2)*cos(q4)^2*cos(q5)*cos(q6)*sin(q3)*sin(q5)*sin(q6) - dq1*dqr2*cos(q3)*cos(q4)^2*cos(q5)*cos(q6)*sin(q2)*sin(q5)*sin(q6) - (3^(1/2)*dq2*dqr1*cos(q2)*cos(q3)*cos(q4)*cos(q5)*cos(q6)*sin(q6))/8 + (3^(1/2)*dq3*dqr1*cos(q2)*cos(q3)*cos(q4)*cos(q5)*cos(q6)*sin(q6))/8 + (3^(1/2)*dq1*dqr2*cos(q2)*cos(q3)*cos(q6)*sin(q4)*sin(q5)*sin(q6))/4 - (3^(1/2)*dq1*dqr2*cos(q4)*cos(q5)*cos(q6)*sin(q2)*sin(q3)*sin(q6))/8 + (3^(1/2)*dq1*dqr2*cos(q6)*sin(q2)*sin(q3)*sin(q4)*sin(q5)*sin(q6))/4 + (5*3^(1/2)*dq1*dqr2*cos(q2)*cos(q3)*cos(q4)*cos(q5)*cos(q6)^2*sin(q5))/16 - (3^(1/2)*dq3*dqr1*cos(q2)*cos(q3)*cos(q4)*cos(q5)^2*cos(q6)*sin(q6))/4 - (3^(1/2)*dq1*dqr2*cos(q2)*cos(q3)*cos(q5)*cos(q6)*sin(q4)*sin(q5)*sin(q6))/2 - (3^(1/2)*dq1*dqr2*cos(q5)*cos(q6)*sin(q2)*sin(q3)*sin(q4)*sin(q5)*sin(q6))/2;
Y5_20_5=(dq3*dqr2*sin(2*q4))/4 - (dq2*dqr2*sin(2*q5))/2 - (dq2*dqr2*sin(2*q4))/4 - (dq2*dqr2*sin(2*q6))/4 + (dq3*dqr2*sin(2*q5))/2 + (dq3*dqr2*sin(2*q6))/4 - (dq1*dqr3*cos(q2)*sin(q3))/2 + (dq1*dqr3*cos(q3)*sin(q2))/2 + (dq1*dqr3*cos(q2)*cos(q4)^2*sin(q3))/2 - (dq1*dqr3*cos(q3)*cos(q4)^2*sin(q2))/2 + (dq1*dqr3*cos(q2)*cos(q5)^2*sin(q3))/2 - (dq1*dqr3*cos(q3)*cos(q5)^2*sin(q2))/2 + (dq1*dqr3*cos(q2)*cos(q6)^2*sin(q3))/2 - (dq1*dqr3*cos(q3)*cos(q6)^2*sin(q2))/2 + (5*dq2*dqr2*cos(q4)^2*cos(q5)*sin(q5))/4 - (5*dq3*dqr2*cos(q4)^2*cos(q5)*sin(q5))/4 + (5*dq2*dqr2*cos(q5)*cos(q6)^2*sin(q5))/4 + (5*dq2*dqr2*cos(q4)^2*cos(q6)*sin(q6))/8 + dq2*dqr2*cos(q5)^2*cos(q6)*sin(q6) - (5*dq3*dqr2*cos(q5)*cos(q6)^2*sin(q5))/4 - (5*dq3*dqr2*cos(q4)^2*cos(q6)*sin(q6))/8 - dq3*dqr2*cos(q5)^2*cos(q6)*sin(q6) - (3^(1/2)*dq6*dqr2*cos(q4)*sin(q5))/4 - (3*dq2*dqr2*cos(q4)^2*cos(q6)^2*sin(q5))/16 + (3*dq3*dqr2*cos(q4)^2*cos(q6)^2*sin(q5))/16 - (3^(1/2)*dq4*dqr2*cos(q4)*cos(q5)*sin(q5))/4 - (3^(1/2)*dq4*dqr2*cos(q4)*cos(q6)*sin(q6))/8 + (3*3^(1/2)*dq6*dqr2*cos(q4)*cos(q6)*sin(q6))/8 - (3^(1/2)*dq1*dqr3*sin(q2)*sin(q3)*sin(q4))/2 - dq1*dqr3*cos(q2)*cos(q4)^2*cos(q5)^2*sin(q3) + dq1*dqr3*cos(q3)*cos(q4)^2*cos(q5)^2*sin(q2) - (5*dq1*dqr3*cos(q2)*cos(q4)^2*cos(q6)^2*sin(q3))/8 + (5*dq1*dqr3*cos(q3)*cos(q4)^2*cos(q6)^2*sin(q2))/8 - (5*dq1*dqr3*cos(q2)*cos(q5)^2*cos(q6)^2*sin(q3))/8 + (5*dq1*dqr3*cos(q3)*cos(q5)^2*cos(q6)^2*sin(q2))/8 - (25*dq2*dqr2*cos(q4)^2*cos(q5)*cos(q6)^2*sin(q5))/16 - (5*dq2*dqr2*cos(q4)^2*cos(q5)^2*cos(q6)*sin(q6))/4 + (25*dq3*dqr2*cos(q4)^2*cos(q5)*cos(q6)^2*sin(q5))/16 + (5*dq3*dqr2*cos(q4)^2*cos(q5)^2*cos(q6)*sin(q6))/4 + (3*3^(1/2)*dq4*dqr2*cos(q4)*cos(q6)^2*sin(q5))/16 + (3^(1/2)*dq6*dqr2*cos(q4)*cos(q6)^2*sin(q5))/4 - (3*dq1*dqr3*cos(q2)*cos(q5)*cos(q6)^2*sin(q3))/8 + (3*dq1*dqr3*cos(q3)*cos(q5)*cos(q6)^2*sin(q2))/8 - (3*dq2*dqr2*cos(q4)^2*cos(q5)*cos(q6)*sin(q6))/8 + (3*dq3*dqr2*cos(q4)^2*cos(q5)*cos(q6)*sin(q6))/8 + (3^(1/2)*dq6*dqr3*cos(q6)*sin(q4)*sin(q5)*sin(q6))/4 + (3*dq1*dqr3*cos(q2)*cos(q4)^2*cos(q5)*cos(q6)^2*sin(q3))/8 - (3*dq1*dqr3*cos(q3)*cos(q4)^2*cos(q5)*cos(q6)^2*sin(q2))/8 + (3^(1/2)*dq1*dqr3*cos(q2)*cos(q3)*cos(q5)^2*sin(q4))/2 + (5*3^(1/2)*dq4*dqr2*cos(q4)*cos(q5)*cos(q6)^2*sin(q5))/16 + (3^(1/2)*dq4*dqr2*cos(q4)*cos(q5)^2*cos(q6)*sin(q6))/4 + (3^(1/2)*dq1*dqr3*cos(q5)^2*sin(q2)*sin(q3)*sin(q4))/2 + (3^(1/2)*dq1*dqr3*cos(q6)^2*sin(q2)*sin(q3)*sin(q4))/2 + (5*dq1*dqr3*cos(q2)*cos(q4)^2*cos(q5)^2*cos(q6)^2*sin(q3))/4 - (5*dq1*dqr3*cos(q3)*cos(q4)^2*cos(q5)^2*cos(q6)^2*sin(q2))/4 + (3*dq1*dqr3*cos(q2)*cos(q6)*sin(q3)*sin(q5)*sin(q6))/4 - (3*dq1*dqr3*cos(q3)*cos(q6)*sin(q2)*sin(q5)*sin(q6))/4 - (3*dq2*dqr3*cos(q4)*cos(q6)*sin(q4)*sin(q5)*sin(q6))/4 + (3*dq3*dqr3*cos(q4)*cos(q6)*sin(q4)*sin(q5)*sin(q6))/4 + (3*3^(1/2)*dq4*dqr2*cos(q4)*cos(q5)*cos(q6)*sin(q6))/8 + (3^(1/2)*dq6*dqr2*cos(q4)*cos(q5)*cos(q6)*sin(q6))/8 - (3^(1/2)*dq1*dqr2*cos(q2)*cos(q3)*cos(q4)*cos(q6)^2*sin(q5))/16 + (3^(1/2)*dq1*dqr3*cos(q4)*cos(q6)^2*sin(q2)*sin(q3)*sin(q5))/16 + (3^(1/2)*dq1*dqr3*cos(q5)*cos(q6)^2*sin(q2)*sin(q3)*sin(q4))/8 + (5*dq1*dqr3*cos(q2)*cos(q4)*cos(q5)*sin(q3)*sin(q4)*sin(q5))/4 - (5*dq1*dqr3*cos(q3)*cos(q4)*cos(q5)*sin(q2)*sin(q4)*sin(q5))/4 + (5*dq1*dqr3*cos(q2)*cos(q4)*cos(q6)*sin(q3)*sin(q4)*sin(q6))/8 - (5*dq1*dqr3*cos(q3)*cos(q4)*cos(q6)*sin(q2)*sin(q4)*sin(q6))/8 + (dq1*dqr3*cos(q2)*cos(q5)*cos(q6)*sin(q3)*sin(q5)*sin(q6))/2 - (dq1*dqr3*cos(q3)*cos(q5)*cos(q6)*sin(q2)*sin(q5)*sin(q6))/2 - dq2*dqr3*cos(q4)*cos(q5)*cos(q6)*sin(q4)*sin(q5)*sin(q6) + dq3*dqr3*cos(q4)*cos(q5)*cos(q6)*sin(q4)*sin(q5)*sin(q6) - (5*3^(1/2)*dq1*dqr3*cos(q2)*cos(q3)*cos(q5)^2*cos(q6)^2*sin(q4))/8 - (5*3^(1/2)*dq1*dqr3*cos(q5)^2*cos(q6)^2*sin(q2)*sin(q3)*sin(q4))/8 - (3*dq1*dqr3*cos(q2)*cos(q4)*cos(q6)^2*sin(q3)*sin(q4)*sin(q5))/16 + (3*dq1*dqr3*cos(q3)*cos(q4)*cos(q6)^2*sin(q2)*sin(q4)*sin(q5))/16 - (3*dq1*dqr3*cos(q2)*cos(q4)^2*cos(q6)*sin(q3)*sin(q5)*sin(q6))/4 + (3*dq1*dqr3*cos(q3)*cos(q4)^2*cos(q6)*sin(q2)*sin(q5)*sin(q6))/4 - (3^(1/2)*dq1*dqr2*cos(q2)*cos(q3)*cos(q4)*cos(q5)*sin(q5))/4 - (3^(1/2)*dq1*dqr2*cos(q2)*cos(q3)*cos(q4)*cos(q6)*sin(q6))/8 + (3^(1/2)*dq1*dqr3*cos(q4)*cos(q5)*sin(q2)*sin(q3)*sin(q5))/4 + (3^(1/2)*dq1*dqr3*cos(q4)*cos(q6)*sin(q2)*sin(q3)*sin(q6))/8 + (3^(1/2)*dq4*dqr3*cos(q5)*cos(q6)*sin(q4)*sin(q5)*sin(q6))/2 - (5*3^(1/2)*dq1*dqr3*cos(q4)*cos(q5)*cos(q6)^2*sin(q2)*sin(q3)*sin(q5))/16 - (3^(1/2)*dq1*dqr3*cos(q4)*cos(q5)^2*cos(q6)*sin(q2)*sin(q3)*sin(q6))/4 - (3*dq1*dqr3*cos(q2)*cos(q4)*cos(q5)*cos(q6)*sin(q3)*sin(q4)*sin(q6))/8 + (3*dq1*dqr3*cos(q3)*cos(q4)*cos(q5)*cos(q6)*sin(q2)*sin(q4)*sin(q6))/8 - (25*dq1*dqr3*cos(q2)*cos(q4)*cos(q5)*cos(q6)^2*sin(q3)*sin(q4)*sin(q5))/16 + (25*dq1*dqr3*cos(q3)*cos(q4)*cos(q5)*cos(q6)^2*sin(q2)*sin(q4)*sin(q5))/16 - (5*dq1*dqr3*cos(q2)*cos(q4)*cos(q5)^2*cos(q6)*sin(q3)*sin(q4)*sin(q6))/4 + (5*dq1*dqr3*cos(q3)*cos(q4)*cos(q5)^2*cos(q6)*sin(q2)*sin(q4)*sin(q6))/4 - dq1*dqr3*cos(q2)*cos(q4)^2*cos(q5)*cos(q6)*sin(q3)*sin(q5)*sin(q6) + dq1*dqr3*cos(q3)*cos(q4)^2*cos(q5)*cos(q6)*sin(q2)*sin(q5)*sin(q6) - (3^(1/2)*dq1*dqr2*cos(q2)*cos(q3)*cos(q4)*cos(q5)*cos(q6)*sin(q6))/8 - (3^(1/2)*dq1*dqr3*cos(q2)*cos(q3)*cos(q6)*sin(q4)*sin(q5)*sin(q6))/4 + (3^(1/2)*dq1*dqr3*cos(q4)*cos(q5)*cos(q6)*sin(q2)*sin(q3)*sin(q6))/8 - (3^(1/2)*dq1*dqr3*cos(q6)*sin(q2)*sin(q3)*sin(q4)*sin(q5)*sin(q6))/4 + (3^(1/2)*dq1*dqr2*cos(q2)*cos(q3)*cos(q4)*cos(q5)^2*cos(q6)*sin(q6))/4 + (3^(1/2)*dq1*dqr3*cos(q2)*cos(q3)*cos(q5)*cos(q6)*sin(q4)*sin(q5)*sin(q6))/2 + (3^(1/2)*dq1*dqr3*cos(q5)*cos(q6)*sin(q2)*sin(q3)*sin(q4)*sin(q5)*sin(q6))/2;
Y5_20_6=(dq2*dqr3*sin(2*q4))/4 + (dq2*dqr3*sin(2*q5))/2 - (dq3*dqr3*sin(2*q4))/4 + (dq2*dqr3*sin(2*q6))/4 - (dq3*dqr3*sin(2*q5))/2 - (dq3*dqr3*sin(2*q6))/4 + (3*dq4*dqr4*cos(q6)^2*sin(q5))/16 - (3*dq6*dqr4*cos(q6)^2*sin(q5))/4 - dq2*dqr3*cos(q4)*cos(q5)^2*sin(q4) - (5*dq2*dqr3*cos(q4)*cos(q6)^2*sin(q4))/8 - (5*dq2*dqr3*cos(q4)^2*cos(q5)*sin(q5))/4 + dq3*dqr3*cos(q4)*cos(q5)^2*sin(q4) + (5*dq3*dqr3*cos(q4)*cos(q6)^2*sin(q4))/8 + (5*dq3*dqr3*cos(q4)^2*cos(q5)*sin(q5))/4 - (5*dq2*dqr3*cos(q5)*cos(q6)^2*sin(q5))/4 - (5*dq2*dqr3*cos(q4)^2*cos(q6)*sin(q6))/8 - dq2*dqr3*cos(q5)^2*cos(q6)*sin(q6) + (5*dq3*dqr3*cos(q5)*cos(q6)^2*sin(q5))/4 + (5*dq3*dqr3*cos(q4)^2*cos(q6)*sin(q6))/8 + dq3*dqr3*cos(q5)^2*cos(q6)*sin(q6) - (15*dq4*dqr4*cos(q5)*cos(q6)^2*sin(q5))/16 + (3^(1/2)*dq6*dqr3*cos(q4)*sin(q5))/4 + (3^(1/2)*dq6*dqr3*cos(q5)*sin(q4))/2 + (3*dq2*dqr3*cos(q4)^2*cos(q6)^2*sin(q5))/16 - (3*dq3*dqr3*cos(q4)^2*cos(q6)^2*sin(q5))/16 - (3^(1/2)*dq2*dqr4*cos(q5)^2*sin(q4))/2 - (3^(1/2)*dq2*dqr4*cos(q6)^2*sin(q4))/8 + (3^(1/2)*dq3*dqr4*cos(q5)^2*sin(q4))/2 + (3^(1/2)*dq4*dqr3*cos(q5)^2*sin(q4))/2 + (3^(1/2)*dq3*dqr4*cos(q6)^2*sin(q4))/8 + (3^(1/2)*dq4*dqr3*cos(q6)^2*sin(q4))/8 + (3*dq1*dqr4*cos(q6)^2*sin(q2)*sin(q3)*sin(q5))/16 - (3^(1/2)*dq1*dqr3*cos(q2)*cos(q3)*sin(q4))/2 - (3^(1/2)*dq2*dqr4*cos(q4)*cos(q5)*sin(q5))/4 + (3^(1/2)*dq3*dqr4*cos(q4)*cos(q5)*sin(q5))/4 + (3^(1/2)*dq4*dqr3*cos(q4)*cos(q5)*sin(q5))/4 + (3^(1/2)*dq4*dqr3*cos(q4)*cos(q6)*sin(q6))/8 - (3*3^(1/2)*dq6*dqr3*cos(q4)*cos(q6)*sin(q6))/8 + (5*dq2*dqr3*cos(q4)*cos(q5)^2*cos(q6)^2*sin(q4))/4 + (25*dq2*dqr3*cos(q4)^2*cos(q5)*cos(q6)^2*sin(q5))/16 - (5*dq3*dqr3*cos(q4)*cos(q5)^2*cos(q6)^2*sin(q4))/4 + (5*dq2*dqr3*cos(q4)^2*cos(q5)^2*cos(q6)*sin(q6))/4 - (25*dq3*dqr3*cos(q4)^2*cos(q5)*cos(q6)^2*sin(q5))/16 - (5*dq3*dqr3*cos(q4)^2*cos(q5)^2*cos(q6)*sin(q6))/4 + (3*3^(1/2)*dq2*dqr4*cos(q4)*cos(q6)^2*sin(q5))/16 - (3*3^(1/2)*dq3*dqr4*cos(q4)*cos(q6)^2*sin(q5))/16 - (3*3^(1/2)*dq4*dqr3*cos(q4)*cos(q6)^2*sin(q5))/16 - (3^(1/2)*dq6*dqr3*cos(q4)*cos(q6)^2*sin(q5))/4 - (3^(1/2)*dq6*dqr3*cos(q5)*cos(q6)^2*sin(q4))/2 + (3*dq1*dqr4*cos(q2)*cos(q3)*cos(q5)*sin(q5))/4 + (3*dq1*dqr4*cos(q5)*sin(q2)*sin(q3)*sin(q5))/4 + (3*dq1*dqr4*cos(q6)*sin(q2)*sin(q3)*sin(q6))/8 + (5*3^(1/2)*dq2*dqr4*cos(q5)^2*cos(q6)^2*sin(q4))/8 - (5*3^(1/2)*dq3*dqr4*cos(q5)^2*cos(q6)^2*sin(q4))/8 - (5*3^(1/2)*dq4*dqr3*cos(q5)^2*cos(q6)^2*sin(q4))/8 + (3*dq1*dqr4*cos(q2)*cos(q3)*cos(q6)^2*sin(q5))/16 + (3*dq2*dqr3*cos(q4)*cos(q5)*cos(q6)^2*sin(q4))/8 - (3*dq3*dqr3*cos(q4)*cos(q5)*cos(q6)^2*sin(q4))/8 + (3*dq2*dqr3*cos(q4)^2*cos(q5)*cos(q6)*sin(q6))/8 - (3*dq3*dqr3*cos(q4)^2*cos(q5)*cos(q6)*sin(q6))/8 + (3^(1/2)*dq1*dqr3*cos(q2)*cos(q3)*cos(q6)^2*sin(q4))/2 - (3^(1/2)*dq1*dqr4*cos(q2)*cos(q4)*cos(q5)^2*sin(q3))/2 + (3^(1/2)*dq1*dqr4*cos(q3)*cos(q4)*cos(q5)^2*sin(q2))/2 - (3^(1/2)*dq1*dqr4*cos(q2)*cos(q4)*cos(q6)^2*sin(q3))/8 + (3^(1/2)*dq1*dqr4*cos(q3)*cos(q4)*cos(q6)^2*sin(q2))/8 + (5*3^(1/2)*dq2*dqr4*cos(q4)*cos(q5)*cos(q6)^2*sin(q5))/16 - (5*3^(1/2)*dq3*dqr4*cos(q4)*cos(q5)*cos(q6)^2*sin(q5))/16 - (5*3^(1/2)*dq4*dqr3*cos(q4)*cos(q5)*cos(q6)^2*sin(q5))/16 - (3^(1/2)*dq4*dqr3*cos(q4)*cos(q5)^2*cos(q6)*sin(q6))/4 + (3*dq1*dqr4*cos(q5)*cos(q6)*sin(q2)*sin(q3)*sin(q6))/8 - (15*dq1*dqr4*cos(q2)*cos(q3)*cos(q5)*cos(q6)^2*sin(q5))/16 - (15*dq1*dqr4*cos(q5)*cos(q6)^2*sin(q2)*sin(q3)*sin(q5))/16 - (3*dq1*dqr4*cos(q5)^2*cos(q6)*sin(q2)*sin(q3)*sin(q6))/4 - (3*3^(1/2)*dq4*dqr3*cos(q4)*cos(q5)*cos(q6)*sin(q6))/8 - (3^(1/2)*dq6*dqr3*cos(q4)*cos(q5)*cos(q6)*sin(q6))/8 + (3^(1/2)*dq1*dqr3*cos(q2)*cos(q3)*cos(q4)*cos(q6)^2*sin(q5))/16 + (3^(1/2)*dq1*dqr3*cos(q2)*cos(q3)*cos(q5)*cos(q6)^2*sin(q4))/8 - (3*3^(1/2)*dq1*dqr4*cos(q2)*cos(q6)^2*sin(q3)*sin(q4)*sin(q5))/16 + (3*3^(1/2)*dq1*dqr4*cos(q3)*cos(q6)^2*sin(q2)*sin(q4)*sin(q5))/16 + (5*3^(1/2)*dq1*dqr4*cos(q2)*cos(q4)*cos(q5)^2*cos(q6)^2*sin(q3))/8 - (5*3^(1/2)*dq1*dqr4*cos(q3)*cos(q4)*cos(q5)^2*cos(q6)^2*sin(q2))/8 + (3^(1/2)*dq1*dqr3*cos(q2)*cos(q3)*cos(q4)*cos(q5)*sin(q5))/4 + (3^(1/2)*dq1*dqr3*cos(q2)*cos(q3)*cos(q4)*cos(q6)*sin(q6))/8 + (3^(1/2)*dq1*dqr4*cos(q2)*cos(q5)*sin(q3)*sin(q4)*sin(q5))/4 - (3^(1/2)*dq1*dqr4*cos(q3)*cos(q5)*sin(q2)*sin(q4)*sin(q5))/4 + (3^(1/2)*dq1*dqr4*cos(q2)*cos(q6)*sin(q3)*sin(q4)*sin(q6))/8 - (3^(1/2)*dq1*dqr4*cos(q3)*cos(q6)*sin(q2)*sin(q4)*sin(q6))/8 - (3^(1/2)*dq2*dqr4*cos(q5)*cos(q6)*sin(q4)*sin(q5)*sin(q6))/2 + (3^(1/2)*dq3*dqr4*cos(q5)*cos(q6)*sin(q4)*sin(q5)*sin(q6))/2 - (5*3^(1/2)*dq1*dqr4*cos(q2)*cos(q5)*cos(q6)^2*sin(q3)*sin(q4)*sin(q5))/16 + (5*3^(1/2)*dq1*dqr4*cos(q3)*cos(q5)*cos(q6)^2*sin(q2)*sin(q4)*sin(q5))/16 - (3^(1/2)*dq1*dqr4*cos(q2)*cos(q5)^2*cos(q6)*sin(q3)*sin(q4)*sin(q6))/4 + (3^(1/2)*dq1*dqr4*cos(q3)*cos(q5)^2*cos(q6)*sin(q2)*sin(q4)*sin(q6))/4 + (3^(1/2)*dq1*dqr3*cos(q2)*cos(q3)*cos(q4)*cos(q5)*cos(q6)*sin(q6))/8 - (3*3^(1/2)*dq1*dqr4*cos(q2)*cos(q5)*cos(q6)*sin(q3)*sin(q4)*sin(q6))/8 + (3*3^(1/2)*dq1*dqr4*cos(q3)*cos(q5)*cos(q6)*sin(q2)*sin(q4)*sin(q6))/8 - (5*3^(1/2)*dq1*dqr3*cos(q2)*cos(q3)*cos(q4)*cos(q5)*cos(q6)^2*sin(q5))/16 - (3^(1/2)*dq1*dqr3*cos(q2)*cos(q3)*cos(q4)*cos(q5)^2*cos(q6)*sin(q6))/4 - (3^(1/2)*dq1*dqr4*cos(q2)*cos(q4)*cos(q5)*cos(q6)*sin(q3)*sin(q5)*sin(q6))/2 + (3^(1/2)*dq1*dqr4*cos(q3)*cos(q4)*cos(q5)*cos(q6)*sin(q2)*sin(q5)*sin(q6))/2;
Y5_20_7=ddqr4/2 + ddqr5 + ddqr6/2 - (3*ddqr4*cos(q6)^2)/8 - (3*ddqr5*cos(q6)^2)/4 + (3*dq4*dqr6*sin(q5))/4 + (3*dq6*dqr4*sin(q5))/4 + (3*dq4*dqr4*sin(2*q5))/8 + (3*dq4*dqr4*sin(2*q6))/16 + (3*dq4*dqr6*sin(2*q6))/16 + (3*dq6*dqr4*sin(2*q6))/16 + (3*dq5*dqr6*sin(2*q6))/8 + (3*dq6*dqr5*sin(2*q6))/8 + (ddqr1*cos(q2)*cos(q3))/2 + (ddqr1*sin(q2)*sin(q3))/2 + (3*ddqr4*cos(q5)*cos(q6)^2)/8 + (3^(1/2)*ddqr2*cos(q4))/2 - (3^(1/2)*ddqr3*cos(q4))/2 - (3*3^(1/2)*ddqr2*cos(q4)*cos(q6)^2)/8 + (3*3^(1/2)*ddqr3*cos(q4)*cos(q6)^2)/8 - (3*dq4*dqr6*cos(q6)^2*sin(q5))/4 - (3*ddqr4*cos(q6)*sin(q5)*sin(q6))/4 - (3*ddqr1*cos(q2)*cos(q3)*cos(q6)^2)/8 - (3*ddqr1*cos(q6)^2*sin(q2)*sin(q3))/8 - (3^(1/2)*ddqr2*cos(q4)*cos(q5)*cos(q6)^2)/8 + (3^(1/2)*ddqr3*cos(q4)*cos(q5)*cos(q6)^2)/8 - (3*dq4*dqr4*cos(q5)^2*cos(q6)*sin(q6))/4 + (3^(1/2)*ddqr2*cos(q6)^2*sin(q4)*sin(q5))/4 - (3^(1/2)*ddqr3*cos(q6)^2*sin(q4)*sin(q5))/4 - (3^(1/2)*dq2*dqr6*cos(q4)*sin(q5))/4 - (3^(1/2)*dq2*dqr6*cos(q5)*sin(q4))/2 + (3^(1/2)*dq3*dqr6*cos(q4)*sin(q5))/4 + (3^(1/2)*dq3*dqr6*cos(q5)*sin(q4))/2 + (3*ddqr1*cos(q2)*cos(q3)*cos(q5)*cos(q6)^2)/8 + (3*ddqr1*cos(q5)*cos(q6)^2*sin(q2)*sin(q3))/8 + (3*dq1*dqr6*cos(q2)*cos(q3)*sin(q5))/4 + (3*dq4*dqr4*cos(q5)*cos(q6)*sin(q6))/8 - (3*dq4*dqr6*cos(q5)*cos(q6)*sin(q6))/8 - (3*dq6*dqr4*cos(q5)*cos(q6)*sin(q6))/8 - (3^(1/2)*ddqr1*cos(q2)*sin(q3)*sin(q4))/2 + (3^(1/2)*ddqr1*cos(q3)*sin(q2)*sin(q4))/2 + (3*dq1*dqr6*sin(q2)*sin(q3)*sin(q5))/4 - (3*dq1*dqr6*cos(q6)^2*sin(q2)*sin(q3)*sin(q5))/4 - (3*ddqr1*cos(q2)*cos(q3)*cos(q6)*sin(q5)*sin(q6))/4 - (3^(1/2)*dq2*dqr4*cos(q4)*cos(q6)*sin(q6))/8 + (3^(1/2)*dq3*dqr4*cos(q4)*cos(q6)*sin(q6))/8 + (3*3^(1/2)*dq2*dqr6*cos(q4)*cos(q6)*sin(q6))/8 - (3*3^(1/2)*dq3*dqr6*cos(q4)*cos(q6)*sin(q6))/8 - (3*ddqr1*cos(q6)*sin(q2)*sin(q3)*sin(q5)*sin(q6))/4 + (3^(1/2)*dq2*dqr6*cos(q4)*cos(q6)^2*sin(q5))/4 + (3^(1/2)*dq2*dqr6*cos(q5)*cos(q6)^2*sin(q4))/2 - (3^(1/2)*dq3*dqr6*cos(q4)*cos(q6)^2*sin(q5))/4 - (3^(1/2)*dq3*dqr6*cos(q5)*cos(q6)^2*sin(q4))/2 + (3*dq1*dqr4*cos(q2)*cos(q3)*cos(q6)*sin(q6))/8 + (3*dq1*dqr6*cos(q2)*cos(q3)*cos(q6)*sin(q6))/8 + (3^(1/2)*ddqr2*cos(q4)*cos(q6)*sin(q5)*sin(q6))/4 + (3^(1/2)*ddqr2*cos(q5)*cos(q6)*sin(q4)*sin(q6))/2 - (3^(1/2)*ddqr3*cos(q4)*cos(q6)*sin(q5)*sin(q6))/4 - (3^(1/2)*ddqr3*cos(q5)*cos(q6)*sin(q4)*sin(q6))/2 + (3*dq1*dqr6*cos(q6)*sin(q2)*sin(q3)*sin(q6))/8 - (3*dq1*dqr6*cos(q2)*cos(q3)*cos(q6)^2*sin(q5))/4 + (3*3^(1/2)*ddqr1*cos(q2)*cos(q6)^2*sin(q3)*sin(q4))/8 - (3*3^(1/2)*ddqr1*cos(q3)*cos(q6)^2*sin(q2)*sin(q4))/8 + (3^(1/2)*dq1*dqr6*cos(q2)*sin(q3)*sin(q4)*sin(q5))/4 - (3^(1/2)*dq1*dqr6*cos(q3)*sin(q2)*sin(q4)*sin(q5))/4 - (3^(1/2)*dq2*dqr6*cos(q6)*sin(q4)*sin(q5)*sin(q6))/4 + (3^(1/2)*dq3*dqr6*cos(q6)*sin(q4)*sin(q5)*sin(q6))/4 + (3^(1/2)*dq2*dqr4*cos(q4)*cos(q5)^2*cos(q6)*sin(q6))/4 - (3^(1/2)*dq3*dqr4*cos(q4)*cos(q5)^2*cos(q6)*sin(q6))/4 + (3*dq1*dqr4*cos(q2)*cos(q3)*cos(q5)*cos(q6)*sin(q6))/8 - (3*dq1*dqr6*cos(q2)*cos(q3)*cos(q5)*cos(q6)*sin(q6))/8 - (3*dq1*dqr6*cos(q5)*cos(q6)*sin(q2)*sin(q3)*sin(q6))/8 - (3*dq1*dqr4*cos(q2)*cos(q3)*cos(q5)^2*cos(q6)*sin(q6))/4 + (3^(1/2)*ddqr1*cos(q2)*cos(q4)*cos(q6)^2*sin(q3)*sin(q5))/4 + (3^(1/2)*ddqr1*cos(q2)*cos(q5)*cos(q6)^2*sin(q3)*sin(q4))/8 - (3^(1/2)*ddqr1*cos(q3)*cos(q4)*cos(q6)^2*sin(q2)*sin(q5))/4 - (3^(1/2)*ddqr1*cos(q3)*cos(q5)*cos(q6)^2*sin(q2)*sin(q4))/8 - (3^(1/2)*dq1*dqr6*cos(q2)*cos(q4)*cos(q5)*sin(q3))/2 + (3^(1/2)*dq1*dqr6*cos(q3)*cos(q4)*cos(q5)*sin(q2))/2 + (3*3^(1/2)*dq2*dqr4*cos(q4)*cos(q5)*cos(q6)*sin(q6))/8 - (3*3^(1/2)*dq3*dqr4*cos(q4)*cos(q5)*cos(q6)*sin(q6))/8 + (3^(1/2)*dq2*dqr6*cos(q4)*cos(q5)*cos(q6)*sin(q6))/8 - (3^(1/2)*dq3*dqr6*cos(q4)*cos(q5)*cos(q6)*sin(q6))/8 + (3^(1/2)*dq1*dqr6*cos(q2)*cos(q4)*cos(q5)*cos(q6)^2*sin(q3))/2 - (3^(1/2)*dq1*dqr6*cos(q3)*cos(q4)*cos(q5)*cos(q6)^2*sin(q2))/2 - (3^(1/2)*dq1*dqr6*cos(q2)*cos(q6)^2*sin(q3)*sin(q4)*sin(q5))/4 + (3^(1/2)*dq1*dqr6*cos(q3)*cos(q6)^2*sin(q2)*sin(q4)*sin(q5))/4 + (3^(1/2)*ddqr1*cos(q2)*cos(q4)*cos(q5)*cos(q6)*sin(q3)*sin(q6))/2 - (3^(1/2)*ddqr1*cos(q3)*cos(q4)*cos(q5)*cos(q6)*sin(q2)*sin(q6))/2 - (3^(1/2)*ddqr1*cos(q2)*cos(q6)*sin(q3)*sin(q4)*sin(q5)*sin(q6))/4 + (3^(1/2)*ddqr1*cos(q3)*cos(q6)*sin(q2)*sin(q4)*sin(q5)*sin(q6))/4 - (3*3^(1/2)*dq1*dqr6*cos(q2)*cos(q6)*sin(q3)*sin(q4)*sin(q6))/8 + (3*3^(1/2)*dq1*dqr6*cos(q3)*cos(q6)*sin(q2)*sin(q4)*sin(q6))/8 - (3^(1/2)*dq1*dqr6*cos(q2)*cos(q4)*cos(q6)*sin(q3)*sin(q5)*sin(q6))/4 - (3^(1/2)*dq1*dqr6*cos(q2)*cos(q5)*cos(q6)*sin(q3)*sin(q4)*sin(q6))/8 + (3^(1/2)*dq1*dqr6*cos(q3)*cos(q4)*cos(q6)*sin(q2)*sin(q5)*sin(q6))/4 + (3^(1/2)*dq1*dqr6*cos(q3)*cos(q5)*cos(q6)*sin(q2)*sin(q4)*sin(q6))/8;
Y5_24_1=(3^(1/2)*cos(q2)*cos(q3)*sin(q5))/2 + (3^(1/2)*sin(q2)*sin(q3)*sin(q5))/2 - cos(q2)*cos(q4)*cos(q5)*sin(q3) + cos(q3)*cos(q4)*cos(q5)*sin(q2) + (cos(q2)*sin(q3)*sin(q4)*sin(q5))/2 - (cos(q3)*sin(q2)*sin(q4)*sin(q5))/2;
Y5_25_1=(cos(q2)*cos(q4)*cos(q5)*cos(q6)*sin(q3))/2 - (3^(1/2)*cos(q2)*cos(q3)*cos(q6)*sin(q5))/4 - (3^(1/2)*cos(q5)*sin(q2)*sin(q3)*sin(q6))/2 - (3^(1/2)*cos(q6)*sin(q2)*sin(q3)*sin(q5))/4 - (3^(1/2)*cos(q2)*cos(q3)*cos(q5)*sin(q6))/2 - (cos(q3)*cos(q4)*cos(q5)*cos(q6)*sin(q2))/2 - cos(q2)*cos(q4)*sin(q3)*sin(q5)*sin(q6) - (cos(q2)*cos(q5)*sin(q3)*sin(q4)*sin(q6))/2 - (cos(q2)*cos(q6)*sin(q3)*sin(q4)*sin(q5))/4 + cos(q3)*cos(q4)*sin(q2)*sin(q5)*sin(q6) + (cos(q3)*cos(q5)*sin(q2)*sin(q4)*sin(q6))/2 + (cos(q3)*cos(q6)*sin(q2)*sin(q4)*sin(q5))/4;
Y6_10_1=(877*ddqr1*sin(q2 - q3)*cos(q5)*cos(q6)*sin(q4))/4000 - (37*dq2*dqr1*cos(q3)*cos(q6)*sin(q2))/4000 + (37*dq3*dqr1*cos(q3)*cos(q6)*sin(q2))/4000 - (87*dq1*dqr1*sin(q3)*sin(q4)*sin(q6))/800 + (37*dq5*dqr1*sin(q2)*sin(q3)*sin(q6))/4000 + (37*3^(1/2)*ddqr1*sin(q2 - q3)*cos(q6)*sin(q4))/2000 - (7*3^(1/2)*ddqr1*sin(q2 - q3)*cos(q5)*sin(q6))/4000 - (7*3^(1/2)*ddqr1*sin(q2 - q3)*cos(q6)*sin(q5))/2000 + (87*dq1*dqr1*cos(2*q2)*sin(q3)*sin(q4)*sin(q6))/800 - (111*dq4*dqr1*cos(2*q5)*sin(q2)*sin(q3)*sin(q6))/16000 - (111*dq4*dqr1*sin(2*q5)*cos(q6)*sin(q2)*sin(q3))/8000 + ddqr1*sin(q2 - q3)*cos(q4)*cos(q6)*sin(q5)*((37*3^(1/2))/2000 + 1577/10000) + ddqr1*sin(q2 - q3)*cos(q4)*cos(q5)*sin(q6)*((111*3^(1/2))/4000 + 1577/20000) - ddqr1*sin(q2 - q3)*sin(q4)*sin(q5)*sin(q6)*((37*3^(1/2))/4000 + 877/8000) - (29*dq1*dqr1*cos(q4)*sin(q3)*sin(q5)*sin(q6))/400 - (29*dq1*dqr1*cos(q5)*sin(q3)*sin(q4)*sin(q6))/800 - (29*dq1*dqr1*cos(q6)*sin(q3)*sin(q4)*sin(q5))/400 + (111*dq5*dqr1*cos(q5)*sin(q2)*sin(q3)*sin(q6))/4000 - dq4*dqr1*sin(q2)*sin(q3)*sin(q6)*((1923*3^(1/2))/80000 + 259/16000) + (37*3^(1/2)*dq2*dqr1*cos(q6)*sin(q2)*sin(q3)*sin(q4))/4000 - (37*3^(1/2)*dq3*dqr1*cos(q6)*sin(q2)*sin(q3)*sin(q4))/4000 - (37*3^(1/2)*dq5*dqr1*cos(q2)*sin(q3)*sin(q4)*sin(q6))/4000 + (37*3^(1/2)*dq5*dqr1*cos(q3)*sin(q2)*sin(q4)*sin(q6))/4000 + (37*dq2*dqr1*cos(2*q4)*cos(2*q5)*cos(q3)*cos(q6)*sin(q2))/4000 - (37*dq3*dqr1*cos(2*q4)*cos(2*q5)*cos(q3)*cos(q6)*sin(q2))/4000 - dq2*dqr1*sin(2*q4)*cos(q2)*sin(q3)*sin(q6)*((1923*3^(1/2))/160000 + 111/6400) + dq2*dqr1*sin(2*q4)*cos(q3)*sin(q2)*sin(q6)*((1923*3^(1/2))/160000 + 111/6400) - dq3*dqr1*sin(2*q4)*cos(q3)*sin(q2)*sin(q6)*((1923*3^(1/2))/160000 + 111/6400) + (37*dq2*dqr1*cos(2*q4)*sin(2*q5)*cos(q2)*sin(q3)*sin(q6))/8000 - (37*dq2*dqr1*cos(2*q4)*sin(2*q5)*cos(q3)*sin(q2)*sin(q6))/8000 + (37*dq2*dqr1*cos(2*q5)*sin(2*q4)*cos(q2)*sin(q3)*sin(q6))/6400 - (37*dq2*dqr1*cos(2*q5)*sin(2*q4)*cos(q3)*sin(q2)*sin(q6))/6400 - (37*dq2*dqr1*sin(2*q4)*sin(2*q5)*cos(q3)*cos(q6)*sin(q2))/3200 + (37*dq3*dqr1*cos(2*q4)*sin(2*q5)*cos(q3)*sin(q2)*sin(q6))/8000 + (37*dq3*dqr1*cos(2*q5)*sin(2*q4)*cos(q3)*sin(q2)*sin(q6))/6400 + (37*dq3*dqr1*sin(2*q4)*sin(2*q5)*cos(q3)*cos(q6)*sin(q2))/3200 + (29*3^(1/2)*dq1*dqr1*sin(2*q2)*cos(q6)*sin(q3)*sin(q5))/400 + (877*dq2*dqr1*cos(q4)*cos(q6)*sin(q2)*sin(q3)*sin(q5))/8000 + (877*dq2*dqr1*cos(q5)*cos(q6)*sin(q2)*sin(q3)*sin(q4))/4000 - (877*dq3*dqr1*cos(q4)*cos(q6)*sin(q2)*sin(q3)*sin(q5))/8000 - (877*dq3*dqr1*cos(q5)*cos(q6)*sin(q2)*sin(q3)*sin(q4))/4000 - (877*dq2*dqr1*sin(q2)*sin(q3)*sin(q4)*sin(q5)*sin(q6))/8000 + (877*dq3*dqr1*sin(q2)*sin(q3)*sin(q4)*sin(q5)*sin(q6))/8000 + dq2*dqr1*cos(q3)*cos(q5)*cos(q6)*sin(q2)*((641*3^(1/2))/40000 + 37/2000) - dq3*dqr1*cos(q3)*cos(q5)*cos(q6)*sin(q2)*((641*3^(1/2))/40000 + 37/2000) + dq2*dqr1*cos(q4)*sin(q2)*sin(q3)*sin(q6)*((37*3^(1/2))/16000 + 2631/16000) - dq3*dqr1*cos(q4)*sin(q2)*sin(q3)*sin(q6)*((37*3^(1/2))/16000 + 2631/16000) - dq4*dqr1*cos(q6)*sin(q2)*sin(q3)*sin(q5)*((641*3^(1/2))/40000 + 37/2000) + dq2*dqr1*cos(q2)*sin(q3)*sin(q5)*sin(q6)*((641*3^(1/2))/80000 + 37/1600) - dq2*dqr1*cos(q3)*sin(q2)*sin(q5)*sin(q6)*((641*3^(1/2))/80000 + 37/1600) - dq3*dqr1*cos(q2)*sin(q3)*sin(q5)*sin(q6)*((641*3^(1/2))/80000 + 37/1600) + dq3*dqr1*cos(q3)*sin(q2)*sin(q5)*sin(q6)*((641*3^(1/2))/80000 + 37/1600) - dq4*dqr1*cos(q2)*sin(q3)*sin(q4)*sin(q6)*((37*3^(1/2))/3200 + 1923/80000) + dq4*dqr1*cos(q3)*sin(q2)*sin(q4)*sin(q6)*((37*3^(1/2))/3200 + 1923/80000) - dq4*dqr1*cos(q5)*sin(q2)*sin(q3)*sin(q6)*((641*3^(1/2))/80000 - 37/8000) + (29*dq1*dqr1*cos(2*q2)*cos(q4)*sin(q3)*sin(q5)*sin(q6))/400 + (29*dq1*dqr1*cos(2*q2)*cos(q5)*sin(q3)*sin(q4)*sin(q6))/800 + (29*dq1*dqr1*cos(2*q2)*cos(q6)*sin(q3)*sin(q4)*sin(q5))/400 + (37*3^(1/2)*dq4*dqr1*cos(q3)*cos(q4)*cos(q6)*sin(q2))/4000 - (37*3^(1/2)*dq4*dqr1*cos(2*q5)*cos(q3)*cos(q4)*cos(q6)*sin(q2))/4000 + (37*3^(1/2)*dq2*dqr1*cos(2*q5)*cos(q4)*sin(q2)*sin(q3)*sin(q6))/16000 + (37*3^(1/2)*dq2*dqr1*cos(2*q5)*cos(q6)*sin(q2)*sin(q3)*sin(q4))/4000 + (37*3^(1/2)*dq2*dqr1*sin(2*q5)*cos(q4)*cos(q6)*sin(q2)*sin(q3))/8000 - (37*3^(1/2)*dq3*dqr1*cos(2*q5)*cos(q4)*sin(q2)*sin(q3)*sin(q6))/16000 - (37*3^(1/2)*dq3*dqr1*cos(2*q5)*cos(q6)*sin(q2)*sin(q3)*sin(q4))/4000 - (37*3^(1/2)*dq3*dqr1*sin(2*q5)*cos(q4)*cos(q6)*sin(q2)*sin(q3))/8000 - (37*3^(1/2)*dq4*dqr1*cos(2*q5)*cos(q2)*sin(q3)*sin(q4)*sin(q6))/16000 + (37*3^(1/2)*dq4*dqr1*cos(2*q5)*cos(q3)*sin(q2)*sin(q4)*sin(q6))/16000 - (37*3^(1/2)*dq4*dqr1*sin(2*q5)*cos(q2)*cos(q4)*sin(q3)*sin(q6))/8000 - (37*3^(1/2)*dq4*dqr1*sin(2*q5)*cos(q2)*cos(q6)*sin(q3)*sin(q4))/8000 + (37*3^(1/2)*dq4*dqr1*sin(2*q5)*cos(q3)*cos(q4)*sin(q2)*sin(q6))/8000 + (37*3^(1/2)*dq4*dqr1*sin(2*q5)*cos(q3)*cos(q6)*sin(q2)*sin(q4))/8000 - (37*3^(1/2)*dq2*dqr1*sin(2*q5)*sin(q2)*sin(q3)*sin(q4)*sin(q6))/8000 + (37*3^(1/2)*dq3*dqr1*sin(2*q5)*sin(q2)*sin(q3)*sin(q4)*sin(q6))/8000 + dq2*dqr1*cos(q4)*cos(q5)*sin(q2)*sin(q3)*sin(q6)*((111*3^(1/2))/8000 + 877/16000) - dq3*dqr1*cos(q4)*cos(q5)*sin(q2)*sin(q3)*sin(q6)*((111*3^(1/2))/8000 + 877/16000) + dq4*dqr1*cos(q2)*cos(q6)*sin(q3)*sin(q4)*sin(q5)*((37*3^(1/2))/2000 + 1923/40000) - dq4*dqr1*cos(q3)*cos(q6)*sin(q2)*sin(q4)*sin(q5)*((37*3^(1/2))/2000 + 1923/40000) + dq4*dqr1*cos(q2)*cos(q5)*sin(q3)*sin(q4)*sin(q6)*((111*3^(1/2))/8000 + 1923/80000) - dq4*dqr1*cos(q3)*cos(q5)*sin(q2)*sin(q4)*sin(q6)*((111*3^(1/2))/8000 + 1923/80000) - dq2*dqr1*cos(2*q4)*cos(q3)*cos(q5)*cos(q6)*sin(q2)*((641*3^(1/2))/40000 + 37/2000) + dq3*dqr1*cos(2*q4)*cos(q3)*cos(q5)*cos(q6)*sin(q2)*((641*3^(1/2))/40000 + 37/2000) + (37*3^(1/2)*dq4*dqr1*cos(q2)*cos(q4)*sin(q3)*sin(q5)*sin(q6))/4000 - (37*3^(1/2)*dq4*dqr1*cos(q3)*cos(q4)*sin(q2)*sin(q5)*sin(q6))/4000 + (37*3^(1/2)*dq5*dqr1*cos(q2)*cos(q4)*sin(q3)*sin(q5)*sin(q6))/2000 + (37*3^(1/2)*dq5*dqr1*cos(q2)*cos(q5)*sin(q3)*sin(q4)*sin(q6))/4000 - (37*3^(1/2)*dq5*dqr1*cos(q3)*cos(q4)*sin(q2)*sin(q5)*sin(q6))/2000 - (37*3^(1/2)*dq5*dqr1*cos(q3)*cos(q5)*sin(q2)*sin(q4)*sin(q6))/4000 - dq2*dqr1*sin(2*q4)*cos(q2)*cos(q6)*sin(q3)*sin(q5)*((641*3^(1/2))/80000 + 37/4000) + dq2*dqr1*sin(2*q4)*cos(q3)*cos(q6)*sin(q2)*sin(q5)*((641*3^(1/2))/80000 + 37/4000) + dq3*dqr1*sin(2*q4)*cos(q2)*cos(q6)*sin(q3)*sin(q5)*((641*3^(1/2))/80000 + 37/4000) - dq3*dqr1*sin(2*q4)*cos(q3)*cos(q6)*sin(q2)*sin(q5)*((641*3^(1/2))/80000 + 37/4000) - dq2*dqr1*cos(2*q4)*cos(q2)*sin(q3)*sin(q5)*sin(q6)*((641*3^(1/2))/80000 - 37/8000) + dq2*dqr1*cos(2*q4)*cos(q3)*sin(q2)*sin(q5)*sin(q6)*((641*3^(1/2))/80000 - 37/8000) + dq3*dqr1*cos(2*q4)*cos(q2)*sin(q3)*sin(q5)*sin(q6)*((641*3^(1/2))/80000 - 37/8000) - dq3*dqr1*cos(2*q4)*cos(q3)*sin(q2)*sin(q5)*sin(q6)*((641*3^(1/2))/80000 - 37/8000) - dq2*dqr1*sin(2*q4)*cos(q2)*cos(q5)*sin(q3)*sin(q6)*((641*3^(1/2))/160000 - 37/16000) + dq2*dqr1*sin(2*q4)*cos(q3)*cos(q5)*sin(q2)*sin(q6)*((641*3^(1/2))/160000 - 37/16000) + dq3*dqr1*sin(2*q4)*cos(q2)*cos(q5)*sin(q3)*sin(q6)*((641*3^(1/2))/160000 - 37/16000) - dq3*dqr1*sin(2*q4)*cos(q3)*cos(q5)*sin(q2)*sin(q6)*((641*3^(1/2))/160000 - 37/16000);
Y6_10_2=(21*dq1*dqr1*cos(q4)*sin(q6))/4000 + (29*3^(1/2)*dq1*dqr1*cos(q3)*sin(q6))/800 - (37*dq1*dqr1*sin(2*q4)*sin(2*q5)*sin(q6))/16000 + (37*dq2*dqr1*cos(q2)*cos(q6)*sin(q3))/4000 - (87*dq2*dqr1*cos(q2)*cos(q4)*sin(q6))/400 - (37*dq3*dqr1*cos(q2)*cos(q6)*sin(q3))/4000 + (7*dq1*dqr1*cos(q4)*cos(q5)*sin(q6))/4000 + (7*dq1*dqr1*cos(q4)*cos(q6)*sin(q5))/2000 + (7*dq1*dqr1*cos(q5)*cos(q6)*sin(q4))/1000 + (37*dq5*dqr1*cos(q2)*cos(q3)*sin(q6))/4000 - (7*dq1*dqr1*sin(q4)*sin(q5)*sin(q6))/2000 + dq1*dqr1*cos(q6)*sin(q5)*((6847*3^(1/2))/160000 - 111/8000) + dq1*dqr1*cos(q5)*sin(q6)*((6847*3^(1/2))/320000 - 111/32000) - (87*dq1*dqr1*sin(2*q2)*cos(q3)*sin(q4)*sin(q6))/800 - (29*3^(1/2)*dq1*dqr1*cos(q3)*cos(q5)*sin(q6))/800 - (29*3^(1/2)*dq1*dqr1*cos(q3)*cos(q6)*sin(q5))/400 - dq1*dqr1*cos(2*q4)*cos(q6)*sin(q5)*((641*3^(1/2))/160000 + 37/8000) - dq1*dqr1*cos(2*q4)*cos(q5)*sin(q6)*((641*3^(1/2))/320000 - 37/32000) + dq1*dqr1*sin(2*q4)*sin(q5)*sin(q6)*((641*3^(1/2))/160000 - 37/16000) - (29*3^(1/2)*dq1*dqr1*cos(2*q2)*cos(q3)*sin(q6))/800 + (29*dq1*dqr1*cos(q4)*cos(q5)*cos(q6)*sin(q3))/200 - (29*dq2*dqr1*cos(q2)*cos(q4)*cos(q5)*sin(q6))/400 - (29*dq2*dqr1*cos(q2)*cos(q4)*cos(q6)*sin(q5))/200 - (29*dq2*dqr1*cos(q2)*cos(q5)*cos(q6)*sin(q4))/100 + (111*dq5*dqr1*cos(q2)*cos(q3)*cos(q5)*sin(q6))/4000 - (29*3^(1/2)*dq1*dqr1*sin(2*q2)*sin(q3)*sin(q6))/800 + (29*dq2*dqr1*cos(q2)*sin(q4)*sin(q5)*sin(q6))/200 + dq1*dqr1*sin(2*q2)*sin(2*q3)*sin(q6)*((6847*3^(1/2))/320000 - 481/64000) - (333*dq1*dqr1*cos(2*q5)*sin(2*q2)*sin(2*q3)*sin(q6))/64000 - dq4*dqr1*cos(q2)*cos(q3)*sin(q6)*((1923*3^(1/2))/80000 + 259/16000) - (111*dq4*dqr1*cos(2*q5)*cos(q2)*cos(q3)*sin(q6))/16000 + (37*dq1*dqr1*sin(2*q2)*sin(2*q3)*sin(2*q4)*sin(2*q5)*sin(q6))/16000 - (37*dq2*dqr1*cos(2*q4)*cos(2*q5)*cos(q2)*cos(q6)*sin(q3))/4000 + (37*dq3*dqr1*cos(2*q4)*cos(2*q5)*cos(q2)*cos(q6)*sin(q3))/4000 + dq3*dqr1*sin(2*q4)*cos(q2)*sin(q3)*sin(q6)*((1923*3^(1/2))/160000 + 111/6400) - (1231*dq1*dqr1*cos(2*q2)*sin(2*q3)*cos(q5)*sin(q4)*sin(q6))/80000 + (1231*dq1*dqr1*cos(2*q3)*sin(2*q2)*cos(q5)*sin(q4)*sin(q6))/80000 + (37*dq2*dqr1*sin(2*q4)*sin(2*q5)*cos(q2)*cos(q6)*sin(q3))/3200 - (37*dq3*dqr1*cos(2*q4)*sin(2*q5)*cos(q2)*sin(q3)*sin(q6))/8000 - (37*dq3*dqr1*cos(2*q5)*sin(2*q4)*cos(q2)*sin(q3)*sin(q6))/6400 - (37*dq3*dqr1*sin(2*q4)*sin(2*q5)*cos(q2)*cos(q6)*sin(q3))/3200 + (29*3^(1/2)*dq1*dqr1*cos(2*q2)*cos(q3)*cos(q5)*sin(q6))/800 + (29*3^(1/2)*dq1*dqr1*cos(2*q2)*cos(q3)*cos(q6)*sin(q5))/400 + (877*dq2*dqr1*cos(q2)*cos(q3)*cos(q4)*cos(q6)*sin(q5))/8000 + (877*dq2*dqr1*cos(q2)*cos(q3)*cos(q5)*cos(q6)*sin(q4))/4000 - (877*dq3*dqr1*cos(q2)*cos(q3)*cos(q4)*cos(q6)*sin(q5))/8000 - (877*dq3*dqr1*cos(q2)*cos(q3)*cos(q5)*cos(q6)*sin(q4))/4000 - dq1*dqr1*cos(2*q2)*cos(2*q3)*cos(q6)*sin(q5)*((9411*3^(1/2))/160000 + 37/8000) - dq1*dqr1*cos(2*q2)*cos(2*q3)*cos(q5)*sin(q6)*((9411*3^(1/2))/320000 - 259/32000) + (29*3^(1/2)*dq1*dqr1*sin(2*q2)*cos(q5)*sin(q3)*sin(q6))/800 - (877*dq2*dqr1*cos(q2)*cos(q3)*sin(q4)*sin(q5)*sin(q6))/8000 + (877*dq3*dqr1*cos(q2)*cos(q3)*sin(q4)*sin(q5)*sin(q6))/8000 - dq1*dqr1*cos(2*q2)*sin(2*q3)*sin(q4)*sin(q6)*((111*3^(1/2))/16000 + 7539/80000) + dq1*dqr1*cos(2*q3)*sin(2*q2)*sin(q4)*sin(q6)*((111*3^(1/2))/16000 + 7539/80000) - dq1*dqr1*sin(2*q2)*sin(2*q3)*cos(q6)*sin(q5)*((9411*3^(1/2))/160000 + 37/8000) - dq1*dqr1*sin(2*q2)*sin(2*q3)*cos(q5)*sin(q6)*((9411*3^(1/2))/320000 - 259/32000) + dq2*dqr1*cos(q2)*cos(q3)*cos(q4)*sin(q6)*((37*3^(1/2))/16000 + 2631/16000) - dq3*dqr1*cos(q2)*cos(q3)*cos(q4)*sin(q6)*((37*3^(1/2))/16000 + 2631/16000) - dq2*dqr1*cos(q2)*cos(q5)*cos(q6)*sin(q3)*((641*3^(1/2))/40000 + 37/2000) + dq3*dqr1*cos(q2)*cos(q5)*cos(q6)*sin(q3)*((641*3^(1/2))/40000 + 37/2000) - dq4*dqr1*cos(q2)*cos(q3)*cos(q6)*sin(q5)*((641*3^(1/2))/40000 + 37/2000) - dq4*dqr1*cos(q2)*cos(q3)*cos(q5)*sin(q6)*((641*3^(1/2))/80000 - 37/8000) - (29*dq1*dqr1*cos(2*q2)*cos(q4)*cos(q5)*cos(q6)*sin(q3))/200 - (37*dq1*dqr1*cos(2*q2)*cos(2*q3)*cos(2*q4)*cos(2*q5)*sin(q6))/12800 - (29*dq1*dqr1*sin(2*q2)*cos(q3)*cos(q4)*sin(q5)*sin(q6))/400 - (29*dq1*dqr1*sin(2*q2)*cos(q3)*cos(q5)*sin(q4)*sin(q6))/800 - (29*dq1*dqr1*sin(2*q2)*cos(q3)*cos(q6)*sin(q4)*sin(q5))/400 + dq1*dqr1*cos(2*q4)*sin(2*q2)*sin(2*q3)*sin(q6)*((1923*3^(1/2))/320000 + 111/12800) + (37*3^(1/2)*dq2*dqr1*cos(q2)*cos(q3)*cos(q6)*sin(q4))/4000 - (37*3^(1/2)*dq3*dqr1*cos(q2)*cos(q3)*cos(q6)*sin(q4))/4000 - (37*3^(1/2)*dq4*dqr1*cos(q2)*cos(q4)*cos(q6)*sin(q3))/4000 + (37*dq1*dqr1*cos(2*q2)*cos(2*q3)*sin(2*q4)*sin(2*q5)*sin(q6))/16000 - (37*dq1*dqr1*cos(2*q4)*cos(2*q5)*sin(2*q2)*sin(2*q3)*sin(q6))/12800 + (37*3^(1/2)*dq2*dqr1*cos(2*q5)*cos(q2)*cos(q3)*cos(q4)*sin(q6))/16000 + (37*3^(1/2)*dq2*dqr1*cos(2*q5)*cos(q2)*cos(q3)*cos(q6)*sin(q4))/4000 - (37*3^(1/2)*dq3*dqr1*cos(2*q5)*cos(q2)*cos(q3)*cos(q4)*sin(q6))/16000 - (37*3^(1/2)*dq3*dqr1*cos(2*q5)*cos(q2)*cos(q3)*cos(q6)*sin(q4))/4000 + (37*3^(1/2)*dq4*dqr1*cos(2*q5)*cos(q2)*cos(q4)*cos(q6)*sin(q3))/4000 - (37*3^(1/2)*dq2*dqr1*sin(2*q5)*cos(q2)*cos(q3)*sin(q4)*sin(q6))/8000 + (37*3^(1/2)*dq3*dqr1*sin(2*q5)*cos(q2)*cos(q3)*sin(q4)*sin(q6))/8000 + dq1*dqr1*cos(2*q2)*sin(2*q3)*cos(q4)*sin(q5)*sin(q6)*((37*3^(1/2))/8000 - 877/16000) - dq1*dqr1*cos(2*q3)*sin(2*q2)*cos(q4)*sin(q5)*sin(q6)*((37*3^(1/2))/8000 - 877/16000) + dq1*dqr1*cos(2*q2)*sin(2*q3)*cos(q6)*sin(q4)*sin(q5)*((37*3^(1/2))/4000 - 1231/40000) - dq1*dqr1*cos(2*q3)*sin(2*q2)*cos(q6)*sin(q4)*sin(q5)*((37*3^(1/2))/4000 - 1231/40000) + dq2*dqr1*cos(q2)*cos(q3)*cos(q4)*cos(q5)*sin(q6)*((111*3^(1/2))/8000 + 877/16000) - dq3*dqr1*cos(q2)*cos(q3)*cos(q4)*cos(q5)*sin(q6)*((111*3^(1/2))/8000 + 877/16000) + dq1*dqr1*cos(2*q2)*cos(2*q3)*cos(2*q4)*cos(q6)*sin(q5)*((641*3^(1/2))/160000 + 37/8000) + dq1*dqr1*cos(2*q2)*cos(2*q3)*cos(2*q4)*cos(q5)*sin(q6)*((641*3^(1/2))/320000 - 37/32000) + dq1*dqr1*cos(2*q4)*sin(2*q2)*sin(2*q3)*cos(q6)*sin(q5)*((641*3^(1/2))/160000 + 37/8000) - dq1*dqr1*cos(2*q2)*cos(2*q3)*sin(2*q4)*sin(q5)*sin(q6)*((641*3^(1/2))/160000 - 37/16000) + dq1*dqr1*cos(2*q4)*sin(2*q2)*sin(2*q3)*cos(q5)*sin(q6)*((641*3^(1/2))/320000 - 37/32000) - dq1*dqr1*sin(2*q2)*sin(2*q3)*sin(2*q4)*sin(q5)*sin(q6)*((641*3^(1/2))/160000 - 37/16000) + dq2*dqr1*cos(2*q4)*cos(q2)*cos(q5)*cos(q6)*sin(q3)*((641*3^(1/2))/40000 + 37/2000) - dq3*dqr1*cos(2*q4)*cos(q2)*cos(q5)*cos(q6)*sin(q3)*((641*3^(1/2))/40000 + 37/2000) - (37*3^(1/2)*dq1*dqr1*cos(2*q2)*cos(2*q5)*sin(2*q3)*sin(q4)*sin(q6))/16000 - (37*3^(1/2)*dq1*dqr1*cos(2*q2)*sin(2*q3)*sin(2*q5)*cos(q4)*sin(q6))/8000 - (37*3^(1/2)*dq1*dqr1*cos(2*q2)*sin(2*q3)*sin(2*q5)*cos(q6)*sin(q4))/8000 + (37*3^(1/2)*dq1*dqr1*cos(2*q3)*cos(2*q5)*sin(2*q2)*sin(q4)*sin(q6))/16000 + (37*3^(1/2)*dq1*dqr1*cos(2*q3)*sin(2*q2)*sin(2*q5)*cos(q4)*sin(q6))/8000 + (37*3^(1/2)*dq1*dqr1*cos(2*q3)*sin(2*q2)*sin(2*q5)*cos(q6)*sin(q4))/8000;
Y6_10_3=(29*3^(1/2)*dq2*dqr2*cos(q3)*sin(q6))/400 - (111*dq1*dqr1*cos(2*q5)*sin(q6))/64000 - (111*dq1*dqr1*sin(2*q5)*cos(q6))/32000 - dq1*dqr1*sin(q6)*((14539*3^(1/2))/320000 + 111/12800) - (37*3^(1/2)*dq4*dqr2*cos(q6)*sin(q4))/4000 + (37*3^(1/2)*dq5*dqr2*cos(q4)*sin(q6))/4000 - dq1*dqr1*cos(2*q4)*sin(q6)*((1923*3^(1/2))/320000 + 111/12800) + (37*dq1*dqr1*cos(2*q4)*cos(2*q5)*sin(q6))/12800 + (37*dq1*dqr1*cos(2*q4)*sin(2*q5)*cos(q6))/6400 + (37*dq1*dqr1*cos(2*q5)*sin(2*q4)*cos(q6))/8000 + (37*dq1*dqr2*cos(q2)*cos(q6)*sin(q3))/4000 - (37*dq1*dqr2*cos(q3)*cos(q6)*sin(q2))/4000 - (87*dq1*dqr2*cos(q2)*cos(q4)*sin(q6))/400 - (87*dq2*dqr2*sin(q3)*sin(q4)*sin(q6))/400 + dq4*dqr2*cos(q4)*sin(q6)*((37*3^(1/2))/3200 + 1923/80000) + dq2*dqr2*cos(q6)*sin(q5)*((8129*3^(1/2))/80000 - 37/4000) - dq3*dqr2*cos(q6)*sin(q5)*((8129*3^(1/2))/80000 - 37/4000) - (29*3^(1/2)*dq2*dqr2*cos(q3)*cos(q5)*sin(q6))/400 - (29*3^(1/2)*dq2*dqr2*cos(q3)*cos(q6)*sin(q5))/200 - (37*3^(1/2)*dq5*dqr2*cos(q4)*cos(q5)*sin(q6))/4000 - dq1*dqr1*sin(2*q4)*cos(q5)*cos(q6)*((641*3^(1/2))/80000 + 37/4000) + dq2*dqr2*cos(2*q4)*cos(q6)*sin(q5)*((641*3^(1/2))/80000 + 37/4000) - dq3*dqr2*cos(2*q4)*cos(q6)*sin(q5)*((641*3^(1/2))/80000 + 37/4000) + (37*3^(1/2)*dq4*dqr2*sin(q4)*sin(q5)*sin(q6))/4000 + (37*3^(1/2)*dq5*dqr2*sin(q4)*sin(q5)*sin(q6))/2000 - dq2*dqr2*sin(2*q4)*sin(q5)*sin(q6)*((641*3^(1/2))/80000 - 37/8000) + dq3*dqr2*sin(2*q4)*sin(q5)*sin(q6)*((641*3^(1/2))/80000 - 37/8000) + (37*3^(1/2)*dq4*dqr2*cos(2*q5)*cos(q4)*sin(q6))/16000 + (37*3^(1/2)*dq4*dqr2*cos(2*q5)*cos(q6)*sin(q4))/4000 - (29*dq1*dqr2*cos(q2)*cos(q4)*cos(q5)*sin(q6))/400 - (29*dq1*dqr2*cos(q2)*cos(q4)*cos(q6)*sin(q5))/200 - (29*dq1*dqr2*cos(q2)*cos(q5)*cos(q6)*sin(q4))/100 + (29*dq2*dqr2*cos(q4)*cos(q5)*cos(q6)*sin(q3))/100 + dq1*dqr1*cos(2*q2)*cos(2*q3)*sin(q6)*((6847*3^(1/2))/320000 - 481/64000) - (37*3^(1/2)*dq4*dqr2*sin(2*q5)*sin(q4)*sin(q6))/8000 - (333*dq1*dqr1*cos(2*q2)*cos(2*q3)*cos(2*q5)*sin(q6))/64000 - (333*dq1*dqr1*cos(2*q2)*cos(2*q3)*sin(2*q5)*cos(q6))/32000 + (29*dq1*dqr2*cos(q2)*sin(q4)*sin(q5)*sin(q6))/200 - (29*dq2*dqr2*cos(q4)*sin(q3)*sin(q5)*sin(q6))/200 - (29*dq2*dqr2*cos(q5)*sin(q3)*sin(q4)*sin(q6))/400 - (29*dq2*dqr2*cos(q6)*sin(q3)*sin(q4)*sin(q5))/200 - (333*dq1*dqr1*sin(2*q2)*sin(2*q3)*sin(2*q5)*cos(q6))/32000 - dq4*dqr2*cos(q4)*cos(q6)*sin(q5)*((37*3^(1/2))/2000 + 1923/40000) - dq4*dqr2*cos(q4)*cos(q5)*sin(q6)*((111*3^(1/2))/8000 + 1923/80000) - (111*dq4*dqr1*sin(2*q5)*cos(q2)*cos(q3)*cos(q6))/8000 + (37*3^(1/2)*dq1*dqr2*cos(q6)*sin(q2)*sin(q3)*sin(q4))/4000 + (877*dq1*dqr1*cos(2*q2)*sin(2*q3)*cos(q4)*cos(q5)*cos(q6))/8000 - (877*dq1*dqr1*cos(2*q3)*sin(2*q2)*cos(q4)*cos(q5)*cos(q6))/8000 - (37*dq1*dqr2*cos(2*q4)*cos(2*q5)*cos(q2)*cos(q6)*sin(q3))/4000 + (37*dq1*dqr2*cos(2*q4)*cos(2*q5)*cos(q3)*cos(q6)*sin(q2))/4000 - dq1*dqr2*sin(2*q4)*cos(q2)*sin(q3)*sin(q6)*((1923*3^(1/2))/160000 + 111/6400) + dq1*dqr2*sin(2*q4)*cos(q3)*sin(q2)*sin(q6)*((1923*3^(1/2))/160000 + 111/6400) + (37*dq1*dqr2*cos(2*q4)*sin(2*q5)*cos(q2)*sin(q3)*sin(q6))/8000 - (37*dq1*dqr2*cos(2*q4)*sin(2*q5)*cos(q3)*sin(q2)*sin(q6))/8000 + (37*dq1*dqr2*cos(2*q5)*sin(2*q4)*cos(q2)*sin(q3)*sin(q6))/6400 - (37*dq1*dqr2*cos(2*q5)*sin(2*q4)*cos(q3)*sin(q2)*sin(q6))/6400 + (37*dq1*dqr2*sin(2*q4)*sin(2*q5)*cos(q2)*cos(q6)*sin(q3))/3200 - (37*dq1*dqr2*sin(2*q4)*sin(2*q5)*cos(q3)*cos(q6)*sin(q2))/3200 + (877*dq1*dqr2*cos(q2)*cos(q3)*cos(q4)*cos(q6)*sin(q5))/8000 + (877*dq1*dqr2*cos(q2)*cos(q3)*cos(q5)*cos(q6)*sin(q4))/4000 - (877*dq1*dqr2*cos(q2)*cos(q3)*sin(q4)*sin(q5)*sin(q6))/8000 + (877*dq1*dqr2*cos(q4)*cos(q6)*sin(q2)*sin(q3)*sin(q5))/8000 + (877*dq1*dqr2*cos(q5)*cos(q6)*sin(q2)*sin(q3)*sin(q4))/4000 - (877*dq1*dqr2*sin(q2)*sin(q3)*sin(q4)*sin(q5)*sin(q6))/8000 + dq1*dqr2*cos(q2)*cos(q3)*cos(q4)*sin(q6)*((37*3^(1/2))/16000 + 2631/16000) - dq1*dqr2*cos(q2)*cos(q5)*cos(q6)*sin(q3)*((641*3^(1/2))/40000 + 37/2000) + dq1*dqr2*cos(q3)*cos(q5)*cos(q6)*sin(q2)*((641*3^(1/2))/40000 + 37/2000) + (29*dq1*dqr1*sin(2*q2)*cos(q3)*cos(q4)*cos(q5)*cos(q6))/200 + dq1*dqr1*cos(2*q2)*cos(2*q3)*cos(2*q4)*sin(q6)*((1923*3^(1/2))/320000 + 111/12800) + dq1*dqr2*cos(q4)*sin(q2)*sin(q3)*sin(q6)*((37*3^(1/2))/16000 + 2631/16000) + dq1*dqr2*cos(q2)*sin(q3)*sin(q5)*sin(q6)*((641*3^(1/2))/80000 + 37/1600) - dq1*dqr2*cos(q3)*sin(q2)*sin(q5)*sin(q6)*((641*3^(1/2))/80000 + 37/1600) - (37*dq1*dqr1*cos(2*q2)*cos(2*q3)*cos(2*q4)*sin(2*q5)*cos(q6))/6400 - (37*dq1*dqr1*cos(2*q2)*cos(2*q3)*cos(2*q5)*sin(2*q4)*cos(q6))/8000 + (37*3^(1/2)*dq1*dqr2*cos(q2)*cos(q3)*cos(q6)*sin(q4))/4000 - (37*dq1*dqr1*cos(2*q4)*sin(2*q2)*sin(2*q3)*sin(2*q5)*cos(q6))/6400 - (37*dq1*dqr1*cos(2*q5)*sin(2*q2)*sin(2*q3)*sin(2*q4)*cos(q6))/8000 + (37*3^(1/2)*dq1*dqr2*cos(2*q5)*cos(q2)*cos(q3)*cos(q4)*sin(q6))/16000 + (37*3^(1/2)*dq1*dqr2*cos(2*q5)*cos(q2)*cos(q3)*cos(q6)*sin(q4))/4000 + (37*3^(1/2)*dq2*dqr1*sin(2*q5)*cos(q2)*cos(q3)*cos(q4)*cos(q6))/8000 - (37*3^(1/2)*dq3*dqr1*sin(2*q5)*cos(q2)*cos(q3)*cos(q4)*cos(q6))/8000 + (37*3^(1/2)*dq1*dqr2*cos(2*q5)*cos(q4)*sin(q2)*sin(q3)*sin(q6))/16000 + (37*3^(1/2)*dq1*dqr2*cos(2*q5)*cos(q6)*sin(q2)*sin(q3)*sin(q4))/4000 - (37*3^(1/2)*dq1*dqr2*sin(2*q5)*cos(q2)*cos(q3)*sin(q4)*sin(q6))/8000 + (37*3^(1/2)*dq1*dqr2*sin(2*q5)*cos(q4)*cos(q6)*sin(q2)*sin(q3))/8000 - (37*3^(1/2)*dq1*dqr2*sin(2*q5)*sin(q2)*sin(q3)*sin(q4)*sin(q6))/8000 + dq1*dqr2*cos(q2)*cos(q3)*cos(q4)*cos(q5)*sin(q6)*((111*3^(1/2))/8000 + 877/16000) + dq1*dqr1*cos(2*q2)*cos(2*q3)*sin(2*q4)*cos(q5)*cos(q6)*((641*3^(1/2))/80000 + 37/4000) + dq1*dqr2*cos(q4)*cos(q5)*sin(q2)*sin(q3)*sin(q6)*((111*3^(1/2))/8000 + 877/16000) + dq1*dqr1*sin(2*q2)*sin(2*q3)*sin(2*q4)*cos(q5)*cos(q6)*((641*3^(1/2))/80000 + 37/4000) + (37*3^(1/2)*dq1*dqr1*cos(2*q2)*cos(2*q5)*sin(2*q3)*cos(q4)*cos(q6))/4000 - (37*3^(1/2)*dq1*dqr1*cos(2*q3)*cos(2*q5)*sin(2*q2)*cos(q4)*cos(q6))/4000 + dq1*dqr2*cos(2*q4)*cos(q2)*cos(q5)*cos(q6)*sin(q3)*((641*3^(1/2))/40000 + 37/2000) - dq1*dqr2*cos(2*q4)*cos(q3)*cos(q5)*cos(q6)*sin(q2)*((641*3^(1/2))/40000 + 37/2000) - dq1*dqr2*sin(2*q4)*cos(q2)*cos(q6)*sin(q3)*sin(q5)*((641*3^(1/2))/80000 + 37/4000) + dq1*dqr2*sin(2*q4)*cos(q3)*cos(q6)*sin(q2)*sin(q5)*((641*3^(1/2))/80000 + 37/4000) - dq1*dqr2*cos(2*q4)*cos(q2)*sin(q3)*sin(q5)*sin(q6)*((641*3^(1/2))/80000 - 37/8000) + dq1*dqr2*cos(2*q4)*cos(q3)*sin(q2)*sin(q5)*sin(q6)*((641*3^(1/2))/80000 - 37/8000) - dq1*dqr2*sin(2*q4)*cos(q2)*cos(q5)*sin(q3)*sin(q6)*((641*3^(1/2))/160000 - 37/16000) + dq1*dqr2*sin(2*q4)*cos(q3)*cos(q5)*sin(q2)*sin(q6)*((641*3^(1/2))/160000 - 37/16000);
Y6_10_4=dq2*dqr3*sin(q6)*((10693*3^(1/2))/160000 + 37/32000) - dq2*dqr2*sin(q6)*((10693*3^(1/2))/160000 + 37/32000) + dq3*dqr2*sin(q6)*((10693*3^(1/2))/160000 + 37/32000) - dq3*dqr3*sin(q6)*((10693*3^(1/2))/160000 + 37/32000) + (111*dq2*dqr2*cos(2*q5)*sin(q6))/32000 + (111*dq2*dqr2*sin(2*q5)*cos(q6))/16000 - (111*dq2*dqr3*cos(2*q5)*sin(q6))/32000 - (111*dq3*dqr2*cos(2*q5)*sin(q6))/32000 - (111*dq3*dqr2*sin(2*q5)*cos(q6))/16000 + (111*dq3*dqr3*cos(2*q5)*sin(q6))/32000 + (37*3^(1/2)*dq4*dqr3*cos(q6)*sin(q4))/4000 - (37*3^(1/2)*dq5*dqr3*cos(q4)*sin(q6))/4000 + dq2*dqr2*cos(2*q4)*sin(q6)*((1923*3^(1/2))/160000 + 111/6400) - dq2*dqr3*cos(2*q4)*sin(q6)*((1923*3^(1/2))/160000 + 111/6400) - dq3*dqr2*cos(2*q4)*sin(q6)*((1923*3^(1/2))/160000 + 111/6400) + dq3*dqr3*cos(2*q4)*sin(q6)*((1923*3^(1/2))/160000 + 111/6400) - (37*dq2*dqr2*cos(2*q4)*cos(2*q5)*sin(q6))/6400 - (37*dq2*dqr2*cos(2*q4)*sin(2*q5)*cos(q6))/3200 - (37*dq2*dqr2*cos(2*q5)*sin(2*q4)*cos(q6))/4000 + (37*dq2*dqr3*cos(2*q4)*cos(2*q5)*sin(q6))/6400 + (37*dq3*dqr2*cos(2*q4)*cos(2*q5)*sin(q6))/6400 + (37*dq3*dqr2*cos(2*q4)*sin(2*q5)*cos(q6))/3200 + (37*dq3*dqr2*cos(2*q5)*sin(2*q4)*cos(q6))/4000 - (37*dq3*dqr3*cos(2*q4)*cos(2*q5)*sin(q6))/6400 + (37*dq2*dqr2*sin(2*q4)*sin(2*q5)*sin(q6))/8000 - (37*dq2*dqr3*sin(2*q4)*sin(2*q5)*sin(q6))/8000 - (37*dq3*dqr2*sin(2*q4)*sin(2*q5)*sin(q6))/8000 + (37*dq3*dqr3*sin(2*q4)*sin(2*q5)*sin(q6))/8000 - (37*dq1*dqr3*cos(q2)*cos(q6)*sin(q3))/4000 + (37*dq1*dqr3*cos(q3)*cos(q6)*sin(q2))/4000 - dq4*dqr3*cos(q4)*sin(q6)*((37*3^(1/2))/3200 + 1923/80000) - dq2*dqr3*cos(q6)*sin(q5)*((8129*3^(1/2))/80000 - 37/4000) + dq3*dqr3*cos(q6)*sin(q5)*((8129*3^(1/2))/80000 - 37/4000) + dq2*dqr2*cos(q5)*sin(q6)*((8129*3^(1/2))/160000 - 37/3200) - dq2*dqr3*cos(q5)*sin(q6)*((8129*3^(1/2))/160000 - 37/3200) - dq3*dqr2*cos(q5)*sin(q6)*((8129*3^(1/2))/160000 - 37/3200) + dq3*dqr3*cos(q5)*sin(q6)*((8129*3^(1/2))/160000 - 37/3200) + (37*3^(1/2)*dq5*dqr3*cos(q4)*cos(q5)*sin(q6))/4000 + dq2*dqr2*sin(2*q4)*cos(q5)*cos(q6)*((641*3^(1/2))/40000 + 37/2000) - dq3*dqr2*sin(2*q4)*cos(q5)*cos(q6)*((641*3^(1/2))/40000 + 37/2000) - dq2*dqr3*cos(2*q4)*cos(q6)*sin(q5)*((641*3^(1/2))/80000 + 37/4000) + dq3*dqr3*cos(2*q4)*cos(q6)*sin(q5)*((641*3^(1/2))/80000 + 37/4000) + dq2*dqr2*cos(2*q4)*cos(q5)*sin(q6)*((641*3^(1/2))/160000 - 37/16000) - dq2*dqr3*cos(2*q4)*cos(q5)*sin(q6)*((641*3^(1/2))/160000 - 37/16000) - dq3*dqr2*cos(2*q4)*cos(q5)*sin(q6)*((641*3^(1/2))/160000 - 37/16000) + dq3*dqr3*cos(2*q4)*cos(q5)*sin(q6)*((641*3^(1/2))/160000 - 37/16000) - (37*3^(1/2)*dq4*dqr3*sin(q4)*sin(q5)*sin(q6))/4000 - (37*3^(1/2)*dq5*dqr3*sin(q4)*sin(q5)*sin(q6))/2000 + dq2*dqr3*sin(2*q4)*sin(q5)*sin(q6)*((641*3^(1/2))/80000 - 37/8000) - dq3*dqr3*sin(2*q4)*sin(q5)*sin(q6)*((641*3^(1/2))/80000 - 37/8000) + (37*3^(1/2)*dq4*dqr2*sin(2*q5)*cos(q4)*cos(q6))/8000 - (37*3^(1/2)*dq4*dqr3*cos(2*q5)*cos(q4)*sin(q6))/16000 - (37*3^(1/2)*dq4*dqr3*cos(2*q5)*cos(q6)*sin(q4))/4000 - (37*3^(1/2)*dq4*dqr3*sin(2*q5)*cos(q4)*cos(q6))/8000 + (37*3^(1/2)*dq4*dqr3*sin(2*q5)*sin(q4)*sin(q6))/8000 + dq4*dqr3*cos(q4)*cos(q6)*sin(q5)*((37*3^(1/2))/2000 + 1923/40000) + dq4*dqr3*cos(q4)*cos(q5)*sin(q6)*((111*3^(1/2))/8000 + 1923/80000) - (37*3^(1/2)*dq1*dqr3*cos(q6)*sin(q2)*sin(q3)*sin(q4))/4000 + (37*dq1*dqr3*cos(2*q4)*cos(2*q5)*cos(q2)*cos(q6)*sin(q3))/4000 - (37*dq1*dqr3*cos(2*q4)*cos(2*q5)*cos(q3)*cos(q6)*sin(q2))/4000 + dq1*dqr3*sin(2*q4)*cos(q2)*sin(q3)*sin(q6)*((1923*3^(1/2))/160000 + 111/6400) - dq1*dqr3*sin(2*q4)*cos(q3)*sin(q2)*sin(q6)*((1923*3^(1/2))/160000 + 111/6400) - (37*dq1*dqr3*cos(2*q4)*sin(2*q5)*cos(q2)*sin(q3)*sin(q6))/8000 + (37*dq1*dqr3*cos(2*q4)*sin(2*q5)*cos(q3)*sin(q2)*sin(q6))/8000 - (37*dq1*dqr3*cos(2*q5)*sin(2*q4)*cos(q2)*sin(q3)*sin(q6))/6400 + (37*dq1*dqr3*cos(2*q5)*sin(2*q4)*cos(q3)*sin(q2)*sin(q6))/6400 - (37*dq1*dqr3*sin(2*q4)*sin(2*q5)*cos(q2)*cos(q6)*sin(q3))/3200 + (37*dq1*dqr3*sin(2*q4)*sin(2*q5)*cos(q3)*cos(q6)*sin(q2))/3200 - (877*dq1*dqr3*cos(q2)*cos(q3)*cos(q4)*cos(q6)*sin(q5))/8000 - (877*dq1*dqr3*cos(q2)*cos(q3)*cos(q5)*cos(q6)*sin(q4))/4000 + (877*dq1*dqr3*cos(q2)*cos(q3)*sin(q4)*sin(q5)*sin(q6))/8000 - (877*dq1*dqr3*cos(q4)*cos(q6)*sin(q2)*sin(q3)*sin(q5))/8000 - (877*dq1*dqr3*cos(q5)*cos(q6)*sin(q2)*sin(q3)*sin(q4))/4000 + (877*dq1*dqr3*sin(q2)*sin(q3)*sin(q4)*sin(q5)*sin(q6))/8000 - dq1*dqr3*cos(q2)*cos(q3)*cos(q4)*sin(q6)*((37*3^(1/2))/16000 + 2631/16000) + dq1*dqr3*cos(q2)*cos(q5)*cos(q6)*sin(q3)*((641*3^(1/2))/40000 + 37/2000) - dq1*dqr3*cos(q3)*cos(q5)*cos(q6)*sin(q2)*((641*3^(1/2))/40000 + 37/2000) - dq1*dqr3*cos(q4)*sin(q2)*sin(q3)*sin(q6)*((37*3^(1/2))/16000 + 2631/16000) - dq1*dqr3*cos(q2)*sin(q3)*sin(q5)*sin(q6)*((641*3^(1/2))/80000 + 37/1600) + dq1*dqr3*cos(q3)*sin(q2)*sin(q5)*sin(q6)*((641*3^(1/2))/80000 + 37/1600) - (37*3^(1/2)*dq1*dqr3*cos(q2)*cos(q3)*cos(q6)*sin(q4))/4000 + (37*3^(1/2)*dq1*dqr2*sin(2*q5)*cos(q2)*cos(q3)*cos(q4)*cos(q6))/8000 - (37*3^(1/2)*dq1*dqr3*cos(2*q5)*cos(q2)*cos(q3)*cos(q4)*sin(q6))/16000 - (37*3^(1/2)*dq1*dqr3*cos(2*q5)*cos(q2)*cos(q3)*cos(q6)*sin(q4))/4000 - (37*3^(1/2)*dq1*dqr3*sin(2*q5)*cos(q2)*cos(q3)*cos(q4)*cos(q6))/8000 - (37*3^(1/2)*dq1*dqr3*cos(2*q5)*cos(q4)*sin(q2)*sin(q3)*sin(q6))/16000 - (37*3^(1/2)*dq1*dqr3*cos(2*q5)*cos(q6)*sin(q2)*sin(q3)*sin(q4))/4000 + (37*3^(1/2)*dq1*dqr3*sin(2*q5)*cos(q2)*cos(q3)*sin(q4)*sin(q6))/8000 - (37*3^(1/2)*dq1*dqr3*sin(2*q5)*cos(q4)*cos(q6)*sin(q2)*sin(q3))/8000 + (37*3^(1/2)*dq1*dqr3*sin(2*q5)*sin(q2)*sin(q3)*sin(q4)*sin(q6))/8000 - dq1*dqr3*cos(q2)*cos(q3)*cos(q4)*cos(q5)*sin(q6)*((111*3^(1/2))/8000 + 877/16000) - dq1*dqr3*cos(q4)*cos(q5)*sin(q2)*sin(q3)*sin(q6)*((111*3^(1/2))/8000 + 877/16000) - dq1*dqr3*cos(2*q4)*cos(q2)*cos(q5)*cos(q6)*sin(q3)*((641*3^(1/2))/40000 + 37/2000) + dq1*dqr3*cos(2*q4)*cos(q3)*cos(q5)*cos(q6)*sin(q2)*((641*3^(1/2))/40000 + 37/2000) + dq1*dqr3*sin(2*q4)*cos(q2)*cos(q6)*sin(q3)*sin(q5)*((641*3^(1/2))/80000 + 37/4000) - dq1*dqr3*sin(2*q4)*cos(q3)*cos(q6)*sin(q2)*sin(q5)*((641*3^(1/2))/80000 + 37/4000) + dq1*dqr3*cos(2*q4)*cos(q2)*sin(q3)*sin(q5)*sin(q6)*((641*3^(1/2))/80000 - 37/8000) - dq1*dqr3*cos(2*q4)*cos(q3)*sin(q2)*sin(q5)*sin(q6)*((641*3^(1/2))/80000 - 37/8000) + dq1*dqr3*sin(2*q4)*cos(q2)*cos(q5)*sin(q3)*sin(q6)*((641*3^(1/2))/160000 - 37/16000) - dq1*dqr3*sin(2*q4)*cos(q3)*cos(q5)*sin(q2)*sin(q6)*((641*3^(1/2))/160000 - 37/16000);
Y6_10_5=(37*dq4*dqr5*sin(q6))/4000 + (37*dq5*dqr4*sin(q6))/4000 + (37*dq5*dqr5*sin(q6))/2000 - dq4*dqr4*sin(q6)*((1923*3^(1/2))/80000 + 259/16000) - (111*dq2*dqr3*sin(2*q5)*cos(q6))/16000 + (111*dq3*dqr3*sin(2*q5)*cos(q6))/16000 - (111*dq4*dqr4*cos(2*q5)*sin(q6))/16000 - (111*dq4*dqr4*sin(2*q5)*cos(q6))/8000 - (87*ddqr1*cos(q4)*sin(q2)*sin(q6))/400 + (111*dq4*dqr5*cos(q5)*sin(q6))/4000 + (111*dq5*dqr4*cos(q5)*sin(q6))/4000 + (29*3^(1/2)*ddqr2*sin(q3)*sin(q6))/400 - (29*ddqr1*cos(q4)*cos(q5)*sin(q2)*sin(q6))/400 - (29*ddqr1*cos(q4)*cos(q6)*sin(q2)*sin(q5))/200 - (29*ddqr1*cos(q5)*cos(q6)*sin(q2)*sin(q4))/100 + (29*ddqr2*cos(q3)*cos(q6)*sin(q4)*sin(q5))/200 - (37*3^(1/2)*dq2*dqr4*cos(q6)*sin(q4))/4000 + (37*3^(1/2)*dq2*dqr5*cos(q4)*sin(q6))/4000 + (37*3^(1/2)*dq3*dqr4*cos(q6)*sin(q4))/4000 - (37*3^(1/2)*dq3*dqr5*cos(q4)*sin(q6))/4000 - (21*ddqr1*sin(q2)*sin(q3)*sin(q4)*sin(q6))/4000 + (29*ddqr1*sin(q2)*sin(q4)*sin(q5)*sin(q6))/200 - (43*ddqr1*cos(q2 - q3)*cos(q6)*sin(q4)*sin(q5))/10000 + (37*dq2*dqr3*cos(2*q4)*sin(2*q5)*cos(q6))/3200 + (37*dq2*dqr3*cos(2*q5)*sin(2*q4)*cos(q6))/4000 - (37*dq3*dqr3*cos(2*q4)*sin(2*q5)*cos(q6))/3200 - (37*dq3*dqr3*cos(2*q5)*sin(2*q4)*cos(q6))/4000 + (37*dq1*dqr5*cos(q2)*cos(q3)*sin(q6))/4000 - (7*3^(1/2)*ddqr1*cos(q2)*sin(q3)*sin(q6))/4000 + (7*3^(1/2)*ddqr1*cos(q3)*sin(q2)*sin(q6))/4000 - (29*3^(1/2)*ddqr2*cos(q5)*sin(q3)*sin(q6))/400 - (29*3^(1/2)*ddqr2*cos(q6)*sin(q3)*sin(q5))/200 + (37*dq1*dqr5*sin(q2)*sin(q3)*sin(q6))/4000 - dq4*dqr4*cos(q6)*sin(q5)*((641*3^(1/2))/40000 + 37/2000) + dq2*dqr4*cos(q4)*sin(q6)*((37*3^(1/2))/3200 + 1923/80000) - dq3*dqr4*cos(q4)*sin(q6)*((37*3^(1/2))/3200 + 1923/80000) - dq4*dqr4*cos(q5)*sin(q6)*((641*3^(1/2))/80000 - 37/8000) - (111*dq1*dqr4*cos(2*q5)*sin(q2)*sin(q3)*sin(q6))/16000 - (111*dq1*dqr4*sin(2*q5)*cos(q6)*sin(q2)*sin(q3))/8000 + (ddqr1*cos(q2)*cos(q3)*cos(q6)*sin(q4)*sin(q5))/1250 - (ddqr1*cos(q4)*cos(q5)*cos(q6)*sin(q2)*sin(q3))/625 - (37*3^(1/2)*dq2*dqr5*cos(q4)*cos(q5)*sin(q6))/4000 + (37*3^(1/2)*dq3*dqr5*cos(q4)*cos(q5)*sin(q6))/4000 + (ddqr1*cos(q4)*sin(q2)*sin(q3)*sin(q5)*sin(q6))/1250 + (ddqr1*cos(q5)*sin(q2)*sin(q3)*sin(q4)*sin(q6))/2500 + (ddqr1*cos(q6)*sin(q2)*sin(q3)*sin(q4)*sin(q5))/1250 - dq2*dqr3*sin(2*q4)*cos(q5)*cos(q6)*((641*3^(1/2))/40000 + 37/2000) + dq3*dqr3*sin(2*q4)*cos(q5)*cos(q6)*((641*3^(1/2))/40000 + 37/2000) + (37*3^(1/2)*dq2*dqr4*sin(q4)*sin(q5)*sin(q6))/4000 + (37*3^(1/2)*dq2*dqr5*sin(q4)*sin(q5)*sin(q6))/2000 - (37*3^(1/2)*dq3*dqr4*sin(q4)*sin(q5)*sin(q6))/4000 - (37*3^(1/2)*dq3*dqr5*sin(q4)*sin(q5)*sin(q6))/2000 + ddqr1*cos(q2)*cos(q4)*sin(q3)*sin(q6)*((37*3^(1/2))/4000 - 351/2500) - ddqr1*cos(q3)*cos(q4)*sin(q2)*sin(q6)*((37*3^(1/2))/4000 - 351/2500) + (37*3^(1/2)*dq2*dqr4*cos(2*q5)*cos(q4)*sin(q6))/16000 + (37*3^(1/2)*dq2*dqr4*cos(2*q5)*cos(q6)*sin(q4))/4000 + (37*3^(1/2)*dq2*dqr4*sin(2*q5)*cos(q4)*cos(q6))/8000 - (37*3^(1/2)*dq3*dqr4*cos(2*q5)*cos(q4)*sin(q6))/16000 - (37*3^(1/2)*dq3*dqr4*cos(2*q5)*cos(q6)*sin(q4))/4000 - (37*3^(1/2)*dq3*dqr4*sin(2*q5)*cos(q4)*cos(q6))/8000 + (111*dq1*dqr5*cos(q2)*cos(q3)*cos(q5)*sin(q6))/4000 - (37*3^(1/2)*dq2*dqr4*sin(2*q5)*sin(q4)*sin(q6))/8000 + (37*3^(1/2)*dq3*dqr4*sin(2*q5)*sin(q4)*sin(q6))/8000 + (111*dq1*dqr5*cos(q5)*sin(q2)*sin(q3)*sin(q6))/4000 - dq2*dqr4*cos(q4)*cos(q6)*sin(q5)*((37*3^(1/2))/2000 + 1923/40000) + dq3*dqr4*cos(q4)*cos(q6)*sin(q5)*((37*3^(1/2))/2000 + 1923/40000) - dq2*dqr4*cos(q4)*cos(q5)*sin(q6)*((111*3^(1/2))/8000 + 1923/80000) + dq3*dqr4*cos(q4)*cos(q5)*sin(q6)*((111*3^(1/2))/8000 + 1923/80000) - dq1*dqr4*cos(q2)*cos(q3)*sin(q6)*((1923*3^(1/2))/80000 + 259/16000) - (111*dq1*dqr4*cos(2*q5)*cos(q2)*cos(q3)*sin(q6))/16000 - (111*dq1*dqr4*sin(2*q5)*cos(q2)*cos(q3)*cos(q6))/8000 - dq1*dqr4*sin(q2)*sin(q3)*sin(q6)*((1923*3^(1/2))/80000 + 259/16000) - (37*3^(1/2)*dq1*dqr5*cos(q2)*sin(q3)*sin(q4)*sin(q6))/4000 + (37*3^(1/2)*dq1*dqr5*cos(q3)*sin(q2)*sin(q4)*sin(q6))/4000 - dq1*dqr4*cos(q2)*cos(q3)*cos(q6)*sin(q5)*((641*3^(1/2))/40000 + 37/2000) - dq1*dqr4*cos(q2)*cos(q3)*cos(q5)*sin(q6)*((641*3^(1/2))/80000 - 37/8000) - dq1*dqr4*cos(q6)*sin(q2)*sin(q3)*sin(q5)*((641*3^(1/2))/40000 + 37/2000) - dq1*dqr4*cos(q2)*sin(q3)*sin(q4)*sin(q6)*((37*3^(1/2))/3200 + 1923/80000) + dq1*dqr4*cos(q3)*sin(q2)*sin(q4)*sin(q6)*((37*3^(1/2))/3200 + 1923/80000) - dq1*dqr4*cos(q5)*sin(q2)*sin(q3)*sin(q6)*((641*3^(1/2))/80000 - 37/8000) - (37*3^(1/2)*dq1*dqr4*cos(q2)*cos(q4)*cos(q6)*sin(q3))/4000 + (37*3^(1/2)*dq1*dqr4*cos(q3)*cos(q4)*cos(q6)*sin(q2))/4000 + (37*3^(1/2)*dq1*dqr4*cos(2*q5)*cos(q2)*cos(q4)*cos(q6)*sin(q3))/4000 - (37*3^(1/2)*dq1*dqr4*cos(2*q5)*cos(q3)*cos(q4)*cos(q6)*sin(q2))/4000 - (37*3^(1/2)*dq1*dqr4*cos(2*q5)*cos(q2)*sin(q3)*sin(q4)*sin(q6))/16000 + (37*3^(1/2)*dq1*dqr4*cos(2*q5)*cos(q3)*sin(q2)*sin(q4)*sin(q6))/16000 - (37*3^(1/2)*dq1*dqr4*sin(2*q5)*cos(q2)*cos(q4)*sin(q3)*sin(q6))/8000 - (37*3^(1/2)*dq1*dqr4*sin(2*q5)*cos(q2)*cos(q6)*sin(q3)*sin(q4))/8000 + (37*3^(1/2)*dq1*dqr4*sin(2*q5)*cos(q3)*cos(q4)*sin(q2)*sin(q6))/8000 + (37*3^(1/2)*dq1*dqr4*sin(2*q5)*cos(q3)*cos(q6)*sin(q2)*sin(q4))/8000 + dq1*dqr4*cos(q2)*cos(q6)*sin(q3)*sin(q4)*sin(q5)*((37*3^(1/2))/2000 + 1923/40000) - dq1*dqr4*cos(q3)*cos(q6)*sin(q2)*sin(q4)*sin(q5)*((37*3^(1/2))/2000 + 1923/40000) + dq1*dqr4*cos(q2)*cos(q5)*sin(q3)*sin(q4)*sin(q6)*((111*3^(1/2))/8000 + 1923/80000) - dq1*dqr4*cos(q3)*cos(q5)*sin(q2)*sin(q4)*sin(q6)*((111*3^(1/2))/8000 + 1923/80000) + (37*3^(1/2)*dq1*dqr4*cos(q2)*cos(q4)*sin(q3)*sin(q5)*sin(q6))/4000 - (37*3^(1/2)*dq1*dqr4*cos(q3)*cos(q4)*sin(q2)*sin(q5)*sin(q6))/4000 + (37*3^(1/2)*dq1*dqr5*cos(q2)*cos(q4)*sin(q3)*sin(q5)*sin(q6))/2000 + (37*3^(1/2)*dq1*dqr5*cos(q2)*cos(q5)*sin(q3)*sin(q4)*sin(q6))/4000 - (37*3^(1/2)*dq1*dqr5*cos(q3)*cos(q4)*sin(q2)*sin(q5)*sin(q6))/2000 - (37*3^(1/2)*dq1*dqr5*cos(q3)*cos(q5)*sin(q2)*sin(q4)*sin(q6))/4000;
Y6_10_6=(37*ddqr4*cos(q6))/2000 + (37*ddqr5*cos(q6))/1000 + (37*ddqr1*cos(q2 - q3)*cos(q6))/2000 + (877*ddqr2*cos(q4)*cos(q5)*cos(q6))/4000 - (877*ddqr3*cos(q4)*cos(q5)*cos(q6))/4000 + (87*ddqr2*cos(q3)*sin(q4)*sin(q6))/400 - ddqr4*cos(q5)*cos(q6)*((641*3^(1/2))/20000 + 37/1000) + ddqr2*sin(q4)*sin(q6)*((37*3^(1/2))/4000 - 351/2500) - ddqr3*sin(q4)*sin(q6)*((37*3^(1/2))/4000 - 351/2500) + ddqr4*sin(q5)*sin(q6)*((641*3^(1/2))/40000 + 37/800) + (37*3^(1/2)*ddqr2*cos(q4)*cos(q6))/2000 - (37*3^(1/2)*ddqr3*cos(q4)*cos(q6))/2000 - (29*ddqr2*cos(q3)*cos(q4)*cos(q5)*cos(q6))/100 - (21*ddqr1*cos(q2)*cos(q3)*sin(q4)*sin(q6))/4000 + (29*ddqr2*cos(q3)*cos(q4)*sin(q5)*sin(q6))/200 + (29*ddqr2*cos(q3)*cos(q5)*sin(q4)*sin(q6))/400 + (43*ddqr1*cos(q2 - q3)*cos(q4)*cos(q5)*cos(q6))/5000 - (43*ddqr1*cos(q2 - q3)*cos(q4)*sin(q5)*sin(q6))/10000 - (43*ddqr1*cos(q2 - q3)*cos(q5)*sin(q4)*sin(q6))/20000 - ddqr2*cos(q4)*sin(q5)*sin(q6)*((37*3^(1/2))/4000 + 877/8000) + ddqr3*cos(q4)*sin(q5)*sin(q6)*((37*3^(1/2))/4000 + 877/8000) - ddqr2*cos(q6)*sin(q4)*sin(q5)*((37*3^(1/2))/2000 + 1577/10000) + ddqr3*cos(q6)*sin(q4)*sin(q5)*((37*3^(1/2))/2000 + 1577/10000) - ddqr2*cos(q5)*sin(q4)*sin(q6)*((111*3^(1/2))/4000 + 1577/20000) + ddqr3*cos(q5)*sin(q4)*sin(q6)*((111*3^(1/2))/4000 + 1577/20000) - ddqr1*cos(q2 - q3)*cos(q5)*cos(q6)*((641*3^(1/2))/20000 + 37/1000) + ddqr1*cos(q2 - q3)*sin(q5)*sin(q6)*((641*3^(1/2))/40000 + 37/800) + (ddqr1*cos(q2)*cos(q3)*cos(q4)*sin(q5)*sin(q6))/1250 + (ddqr1*cos(q2)*cos(q3)*cos(q5)*sin(q4)*sin(q6))/2500 - (ddqr1*cos(q2)*cos(q3)*cos(q4)*cos(q5)*cos(q6))/625;
Y6_20_1=(3^(1/2)*ddqr1*sin(q2 - q3)*sin(q4))/4 - (dq2*dqr1*cos(q3)*sin(q2))/8 + (dq3*dqr1*cos(q3)*sin(q2))/8 + (3*dq4*dqr1*sin(2*q6)*sin(q2)*sin(q3))/64 - (3*dq5*dqr1*sin(2*q6)*sin(q2)*sin(q3))/16 - (3*dq2*dqr1*cos(q3)*cos(q5)*sin(q2))/8 + (3*dq3*dqr1*cos(q3)*cos(q5)*sin(q2))/8 - (3*dq5*dqr1*sin(q2)*sin(q3)*sin(q5))/8 - (3^(1/2)*ddqr1*sin(q2 - q3)*cos(q4)*sin(q5))/2 - (3^(1/2)*ddqr1*sin(q2 - q3)*cos(q5)*sin(q4))/4 + (3*dq4*dqr1*cos(2*q6)*sin(q2)*sin(q3)*sin(q5))/8 + (3*dq4*dqr1*sin(2*q6)*cos(q5)*sin(q2)*sin(q3))/16 + (3*dq5*dqr1*cos(2*q6)*sin(q2)*sin(q3)*sin(q5))/8 + (3*dq5*dqr1*sin(2*q6)*cos(q5)*sin(q2)*sin(q3))/16 - (3^(1/2)*dq4*dqr1*cos(q2)*cos(q4)*sin(q3))/8 + (3^(1/2)*dq4*dqr1*cos(q3)*cos(q4)*sin(q2))/8 + (3^(1/2)*dq2*dqr1*sin(q2)*sin(q3)*sin(q4))/8 - (3^(1/2)*dq3*dqr1*sin(q2)*sin(q3)*sin(q4))/8 - (27*dq2*dqr1*sin(2*q4)*sin(2*q6)*cos(q3)*sin(q2))/128 + (27*dq3*dqr1*sin(2*q4)*sin(2*q6)*cos(q3)*sin(q2))/128 - (15*dq4*dqr1*cos(2*q5)*sin(2*q6)*sin(q2)*sin(q3))/64 - (3*dq4*dqr1*cos(2*q6)*sin(2*q5)*sin(q2)*sin(q3))/16 - (3^(1/2)*dq2*dqr1*cos(q4)*sin(q2)*sin(q3)*sin(q5))/4 - (3^(1/2)*dq2*dqr1*cos(q5)*sin(q2)*sin(q3)*sin(q4))/8 + (3^(1/2)*dq3*dqr1*cos(q4)*sin(q2)*sin(q3)*sin(q5))/4 + (3^(1/2)*dq3*dqr1*cos(q5)*sin(q2)*sin(q3)*sin(q4))/8 - (3^(1/2)*dq4*dqr1*cos(q2)*sin(q3)*sin(q4)*sin(q5))/4 + (3^(1/2)*dq4*dqr1*cos(q3)*sin(q2)*sin(q4)*sin(q5))/4 - (3^(1/2)*dq5*dqr1*cos(q2)*sin(q3)*sin(q4)*sin(q5))/8 + (3^(1/2)*dq5*dqr1*cos(q3)*sin(q2)*sin(q4)*sin(q5))/8 + (3*dq2*dqr1*cos(2*q4)*cos(2*q6)*cos(q3)*cos(q5)*sin(q2))/8 - (3*dq3*dqr1*cos(2*q4)*cos(2*q6)*cos(q3)*cos(q5)*sin(q2))/8 + (3*dq2*dqr1*cos(2*q4)*sin(2*q6)*cos(q2)*sin(q3)*sin(q5))/16 - (3*dq2*dqr1*cos(2*q4)*sin(2*q6)*cos(q3)*sin(q2)*sin(q5))/16 + (3*dq2*dqr1*cos(2*q6)*sin(2*q4)*cos(q2)*sin(q3)*sin(q5))/16 - (3*dq2*dqr1*cos(2*q6)*sin(2*q4)*cos(q3)*sin(q2)*sin(q5))/16 - (3*dq2*dqr1*sin(2*q4)*sin(2*q6)*cos(q3)*cos(q5)*sin(q2))/32 - (3*dq3*dqr1*cos(2*q4)*sin(2*q6)*cos(q2)*sin(q3)*sin(q5))/16 + (3*dq3*dqr1*cos(2*q4)*sin(2*q6)*cos(q3)*sin(q2)*sin(q5))/16 - (3*dq3*dqr1*cos(2*q6)*sin(2*q4)*cos(q2)*sin(q3)*sin(q5))/16 + (3*dq3*dqr1*cos(2*q6)*sin(2*q4)*cos(q3)*sin(q2)*sin(q5))/16 + (3*dq3*dqr1*sin(2*q4)*sin(2*q6)*cos(q3)*cos(q5)*sin(q2))/32 - (9*3^(1/2)*dq2*dqr1*sin(2*q6)*cos(q4)*sin(q2)*sin(q3))/64 + (9*3^(1/2)*dq3*dqr1*sin(2*q6)*cos(q4)*sin(q2)*sin(q3))/64 + (9*3^(1/2)*dq4*dqr1*sin(2*q6)*cos(q2)*sin(q3)*sin(q4))/64 - (9*3^(1/2)*dq4*dqr1*sin(2*q6)*cos(q3)*sin(q2)*sin(q4))/64 + (3*3^(1/2)*dq5*dqr1*sin(2*q6)*cos(q2)*sin(q3)*sin(q4))/16 - (3*3^(1/2)*dq5*dqr1*sin(2*q6)*cos(q3)*sin(q2)*sin(q4))/16 + (dq2*dqr1*cos(2*q4)*cos(2*q5)*cos(2*q6)*cos(q3)*sin(q2))/8 - (dq3*dqr1*cos(2*q4)*cos(2*q5)*cos(2*q6)*cos(q3)*sin(q2))/8 - (5*dq2*dqr1*cos(2*q4)*sin(2*q5)*sin(2*q6)*cos(q3)*sin(q2))/32 - (25*dq2*dqr1*cos(2*q5)*sin(2*q4)*sin(2*q6)*cos(q3)*sin(q2))/128 - (5*dq2*dqr1*cos(2*q6)*sin(2*q4)*sin(2*q5)*cos(q3)*sin(q2))/32 + (5*dq3*dqr1*cos(2*q4)*sin(2*q5)*sin(2*q6)*cos(q3)*sin(q2))/32 + (25*dq3*dqr1*cos(2*q5)*sin(2*q4)*sin(2*q6)*cos(q3)*sin(q2))/128 + (5*dq3*dqr1*cos(2*q6)*sin(2*q4)*sin(2*q5)*cos(q3)*sin(q2))/32 + (3^(1/2)*dq4*dqr1*cos(q2)*cos(q4)*cos(q5)*sin(q3))/8 - (3^(1/2)*dq4*dqr1*cos(q3)*cos(q4)*cos(q5)*sin(q2))/8 + (3^(1/2)*dq5*dqr1*cos(q2)*cos(q4)*cos(q5)*sin(q3))/4 - (3^(1/2)*dq5*dqr1*cos(q3)*cos(q4)*cos(q5)*sin(q2))/4 - (3^(1/2)*dq4*dqr1*cos(2*q6)*cos(q2)*cos(q4)*cos(q5)*sin(q3))/8 + (3^(1/2)*dq4*dqr1*cos(2*q6)*cos(q3)*cos(q4)*cos(q5)*sin(q2))/8 - (3^(1/2)*dq5*dqr1*cos(2*q6)*cos(q2)*cos(q4)*cos(q5)*sin(q3))/4 + (3^(1/2)*dq5*dqr1*cos(2*q6)*cos(q3)*cos(q4)*cos(q5)*sin(q2))/4 + (3^(1/2)*dq2*dqr1*cos(2*q6)*cos(q4)*sin(q2)*sin(q3)*sin(q5))/8 - (3^(1/2)*dq2*dqr1*cos(2*q6)*cos(q5)*sin(q2)*sin(q3)*sin(q4))/8 + (3^(1/2)*dq2*dqr1*sin(2*q6)*cos(q4)*cos(q5)*sin(q2)*sin(q3))/16 - (3^(1/2)*dq3*dqr1*cos(2*q6)*cos(q4)*sin(q2)*sin(q3)*sin(q5))/8 + (3^(1/2)*dq3*dqr1*cos(2*q6)*cos(q5)*sin(q2)*sin(q3)*sin(q4))/8 - (3^(1/2)*dq3*dqr1*sin(2*q6)*cos(q4)*cos(q5)*sin(q2)*sin(q3))/16 - (3^(1/2)*dq4*dqr1*cos(2*q6)*cos(q2)*sin(q3)*sin(q4)*sin(q5))/8 + (3^(1/2)*dq4*dqr1*cos(2*q6)*cos(q3)*sin(q2)*sin(q4)*sin(q5))/8 + (3^(1/2)*dq4*dqr1*sin(2*q6)*cos(q2)*cos(q4)*sin(q3)*sin(q5))/16 - (3^(1/2)*dq4*dqr1*sin(2*q6)*cos(q2)*cos(q5)*sin(q3)*sin(q4))/16 - (3^(1/2)*dq4*dqr1*sin(2*q6)*cos(q3)*cos(q4)*sin(q2)*sin(q5))/16 + (3^(1/2)*dq4*dqr1*sin(2*q6)*cos(q3)*cos(q5)*sin(q2)*sin(q4))/16 + (3^(1/2)*dq5*dqr1*cos(2*q6)*cos(q2)*sin(q3)*sin(q4)*sin(q5))/8 - (3^(1/2)*dq5*dqr1*cos(2*q6)*cos(q3)*sin(q2)*sin(q4)*sin(q5))/8 + (3^(1/2)*dq5*dqr1*sin(2*q6)*cos(q2)*cos(q4)*sin(q3)*sin(q5))/8 + (3^(1/2)*dq5*dqr1*sin(2*q6)*cos(q2)*cos(q5)*sin(q3)*sin(q4))/16 - (3^(1/2)*dq5*dqr1*sin(2*q6)*cos(q3)*cos(q4)*sin(q2)*sin(q5))/8 - (3^(1/2)*dq5*dqr1*sin(2*q6)*cos(q3)*cos(q5)*sin(q2)*sin(q4))/16 + (3^(1/2)*dq2*dqr1*sin(2*q6)*sin(q2)*sin(q3)*sin(q4)*sin(q5))/16 - (3^(1/2)*dq3*dqr1*sin(2*q6)*sin(q2)*sin(q3)*sin(q4)*sin(q5))/16 + (3^(1/2)*dq4*dqr1*cos(2*q5)*cos(2*q6)*cos(q2)*cos(q4)*sin(q3))/8 - (3^(1/2)*dq4*dqr1*cos(2*q5)*cos(2*q6)*cos(q3)*cos(q4)*sin(q2))/8 + (3^(1/2)*dq2*dqr1*cos(2*q5)*cos(2*q6)*sin(q2)*sin(q3)*sin(q4))/8 + (5*3^(1/2)*dq2*dqr1*cos(2*q5)*sin(2*q6)*cos(q4)*sin(q2)*sin(q3))/64 + (3^(1/2)*dq2*dqr1*cos(2*q6)*sin(2*q5)*cos(q4)*sin(q2)*sin(q3))/16 - (3^(1/2)*dq3*dqr1*cos(2*q5)*cos(2*q6)*sin(q2)*sin(q3)*sin(q4))/8 - (5*3^(1/2)*dq3*dqr1*cos(2*q5)*sin(2*q6)*cos(q4)*sin(q2)*sin(q3))/64 - (3^(1/2)*dq3*dqr1*cos(2*q6)*sin(2*q5)*cos(q4)*sin(q2)*sin(q3))/16 - (5*3^(1/2)*dq4*dqr1*cos(2*q5)*sin(2*q6)*cos(q2)*sin(q3)*sin(q4))/64 + (5*3^(1/2)*dq4*dqr1*cos(2*q5)*sin(2*q6)*cos(q3)*sin(q2)*sin(q4))/64 - (3^(1/2)*dq4*dqr1*cos(2*q6)*sin(2*q5)*cos(q2)*sin(q3)*sin(q4))/16 + (3^(1/2)*dq4*dqr1*cos(2*q6)*sin(2*q5)*cos(q3)*sin(q2)*sin(q4))/16 - (5*3^(1/2)*dq4*dqr1*sin(2*q5)*sin(2*q6)*cos(q2)*cos(q4)*sin(q3))/32 + (5*3^(1/2)*dq4*dqr1*sin(2*q5)*sin(2*q6)*cos(q3)*cos(q4)*sin(q2))/32 - (5*3^(1/2)*dq2*dqr1*sin(2*q5)*sin(2*q6)*sin(q2)*sin(q3)*sin(q4))/32 + (5*3^(1/2)*dq3*dqr1*sin(2*q5)*sin(2*q6)*sin(q2)*sin(q3)*sin(q4))/32;
Y6_20_2=(3*dq1*dqr1*cos(2*q6)*sin(q5))/32 + (3*dq1*dqr1*sin(2*q6)*cos(q5))/64 + (dq2*dqr1*cos(q2)*sin(q3))/8 - (dq3*dqr1*cos(q2)*sin(q3))/8 + (3*dq4*dqr1*sin(2*q6)*cos(q2)*cos(q3))/64 - (3*dq5*dqr1*sin(2*q6)*cos(q2)*cos(q3))/16 + (3*dq1*dqr1*cos(2*q4)*cos(2*q6)*sin(q5))/32 + (3*dq1*dqr1*cos(2*q4)*sin(2*q6)*cos(q5))/64 + (3*dq1*dqr1*cos(2*q6)*sin(2*q4)*cos(q5))/16 - (3*dq1*dqr1*sin(2*q4)*sin(2*q6)*sin(q5))/32 + (3*dq2*dqr1*cos(q2)*cos(q5)*sin(q3))/8 - (3*dq3*dqr1*cos(q2)*cos(q5)*sin(q3))/8 - (3*dq5*dqr1*cos(q2)*cos(q3)*sin(q5))/8 + (dq1*dqr1*cos(2*q5)*cos(2*q6)*sin(2*q4))/16 + (9*dq1*dqr1*sin(2*q2)*sin(2*q3)*sin(2*q6))/256 - (5*dq1*dqr1*sin(2*q4)*sin(2*q5)*sin(2*q6))/64 + (3^(1/2)*dq2*dqr1*cos(q2)*cos(q3)*sin(q4))/8 - (3^(1/2)*dq3*dqr1*cos(q2)*cos(q3)*sin(q4))/8 - (27*dq1*dqr1*cos(2*q4)*sin(2*q2)*sin(2*q3)*sin(2*q6))/256 - (45*dq1*dqr1*cos(2*q5)*sin(2*q2)*sin(2*q3)*sin(2*q6))/256 - (9*dq1*dqr1*cos(2*q6)*sin(2*q2)*sin(2*q3)*sin(2*q5))/64 - (15*dq4*dqr1*cos(2*q5)*sin(2*q6)*cos(q2)*cos(q3))/64 - (3*dq4*dqr1*cos(2*q6)*sin(2*q5)*cos(q2)*cos(q3))/16 + (27*dq2*dqr1*sin(2*q4)*sin(2*q6)*cos(q2)*sin(q3))/128 - (27*dq3*dqr1*sin(2*q4)*sin(2*q6)*cos(q2)*sin(q3))/128 + (9*dq1*dqr1*cos(2*q2)*cos(2*q3)*cos(2*q6)*sin(q5))/32 + (9*dq1*dqr1*cos(2*q2)*cos(2*q3)*sin(2*q6)*cos(q5))/64 + (9*dq1*dqr1*cos(2*q6)*sin(2*q2)*sin(2*q3)*sin(q5))/32 + (9*dq1*dqr1*sin(2*q2)*sin(2*q3)*sin(2*q6)*cos(q5))/64 + (3*dq4*dqr1*cos(2*q6)*cos(q2)*cos(q3)*sin(q5))/8 + (3*dq4*dqr1*sin(2*q6)*cos(q2)*cos(q3)*cos(q5))/16 + (3*dq5*dqr1*cos(2*q6)*cos(q2)*cos(q3)*sin(q5))/8 + (3*dq5*dqr1*sin(2*q6)*cos(q2)*cos(q3)*cos(q5))/16 + (3*dq1*dqr1*sin(2*q2)*sin(2*q3)*sin(2*q4)*sin(2*q6)*sin(q5))/32 - (3*dq2*dqr1*cos(2*q4)*cos(2*q6)*cos(q2)*cos(q5)*sin(q3))/8 + (3*dq3*dqr1*cos(2*q4)*cos(2*q6)*cos(q2)*cos(q5)*sin(q3))/8 + (9*3^(1/2)*dq1*dqr1*cos(2*q2)*sin(2*q3)*sin(2*q6)*sin(q4))/64 - (9*3^(1/2)*dq1*dqr1*cos(2*q3)*sin(2*q2)*sin(2*q6)*sin(q4))/64 - (5*dq1*dqr1*cos(2*q2)*cos(2*q3)*cos(2*q4)*cos(2*q6)*sin(2*q5))/64 - (dq1*dqr1*cos(2*q2)*cos(2*q3)*cos(2*q5)*cos(2*q6)*sin(2*q4))/16 + (3*dq2*dqr1*sin(2*q4)*sin(2*q6)*cos(q2)*cos(q5)*sin(q3))/32 - (3*dq3*dqr1*sin(2*q4)*sin(2*q6)*cos(q2)*cos(q5)*sin(q3))/32 - (9*3^(1/2)*dq2*dqr1*sin(2*q6)*cos(q2)*cos(q3)*cos(q4))/64 + (9*3^(1/2)*dq3*dqr1*sin(2*q6)*cos(q2)*cos(q3)*cos(q4))/64 + (5*dq1*dqr1*cos(2*q2)*cos(2*q3)*sin(2*q4)*sin(2*q5)*sin(2*q6))/64 - (25*dq1*dqr1*cos(2*q4)*cos(2*q5)*sin(2*q2)*sin(2*q3)*sin(2*q6))/256 - (5*dq1*dqr1*cos(2*q4)*cos(2*q6)*sin(2*q2)*sin(2*q3)*sin(2*q5))/64 - (dq1*dqr1*cos(2*q5)*cos(2*q6)*sin(2*q2)*sin(2*q3)*sin(2*q4))/16 + (5*dq1*dqr1*sin(2*q2)*sin(2*q3)*sin(2*q4)*sin(2*q5)*sin(2*q6))/64 - (dq2*dqr1*cos(2*q4)*cos(2*q5)*cos(2*q6)*cos(q2)*sin(q3))/8 + (dq3*dqr1*cos(2*q4)*cos(2*q5)*cos(2*q6)*cos(q2)*sin(q3))/8 + (5*dq2*dqr1*cos(2*q4)*sin(2*q5)*sin(2*q6)*cos(q2)*sin(q3))/32 + (25*dq2*dqr1*cos(2*q5)*sin(2*q4)*sin(2*q6)*cos(q2)*sin(q3))/128 + (5*dq2*dqr1*cos(2*q6)*sin(2*q4)*sin(2*q5)*cos(q2)*sin(q3))/32 - (5*dq3*dqr1*cos(2*q4)*sin(2*q5)*sin(2*q6)*cos(q2)*sin(q3))/32 - (25*dq3*dqr1*cos(2*q5)*sin(2*q4)*sin(2*q6)*cos(q2)*sin(q3))/128 - (5*dq3*dqr1*cos(2*q6)*sin(2*q4)*sin(2*q5)*cos(q2)*sin(q3))/32 - (3*dq1*dqr1*cos(2*q2)*cos(2*q3)*cos(2*q4)*cos(2*q6)*sin(q5))/32 - (3*dq1*dqr1*cos(2*q2)*cos(2*q3)*cos(2*q4)*sin(2*q6)*cos(q5))/64 - (3*dq1*dqr1*cos(2*q2)*cos(2*q3)*cos(2*q6)*sin(2*q4)*cos(q5))/16 - (3^(1/2)*dq2*dqr1*cos(q2)*cos(q3)*cos(q4)*sin(q5))/4 - (3^(1/2)*dq2*dqr1*cos(q2)*cos(q3)*cos(q5)*sin(q4))/8 + (3^(1/2)*dq3*dqr1*cos(q2)*cos(q3)*cos(q4)*sin(q5))/4 + (3^(1/2)*dq3*dqr1*cos(q2)*cos(q3)*cos(q5)*sin(q4))/8 + (3*dq1*dqr1*cos(2*q2)*cos(2*q3)*sin(2*q4)*sin(2*q6)*sin(q5))/32 - (3*dq1*dqr1*cos(2*q4)*cos(2*q6)*sin(2*q2)*sin(2*q3)*sin(q5))/32 - (3*dq1*dqr1*cos(2*q4)*sin(2*q2)*sin(2*q3)*sin(2*q6)*cos(q5))/64 - (3*dq1*dqr1*cos(2*q6)*sin(2*q2)*sin(2*q3)*sin(2*q4)*cos(q5))/16 + (3^(1/2)*dq2*dqr1*cos(2*q6)*cos(q2)*cos(q3)*cos(q4)*sin(q5))/8 - (3^(1/2)*dq2*dqr1*cos(2*q6)*cos(q2)*cos(q3)*cos(q5)*sin(q4))/8 + (3^(1/2)*dq2*dqr1*sin(2*q6)*cos(q2)*cos(q3)*cos(q4)*cos(q5))/16 - (3^(1/2)*dq3*dqr1*cos(2*q6)*cos(q2)*cos(q3)*cos(q4)*sin(q5))/8 + (3^(1/2)*dq3*dqr1*cos(2*q6)*cos(q2)*cos(q3)*cos(q5)*sin(q4))/8 - (3^(1/2)*dq3*dqr1*sin(2*q6)*cos(q2)*cos(q3)*cos(q4)*cos(q5))/16 + (3^(1/2)*dq1*dqr1*cos(2*q2)*cos(2*q5)*cos(2*q6)*sin(2*q3)*cos(q4))/8 - (3^(1/2)*dq1*dqr1*cos(2*q3)*cos(2*q5)*cos(2*q6)*sin(2*q2)*cos(q4))/8 + (3^(1/2)*dq2*dqr1*sin(2*q6)*cos(q2)*cos(q3)*sin(q4)*sin(q5))/16 - (3^(1/2)*dq3*dqr1*sin(2*q6)*cos(q2)*cos(q3)*sin(q4)*sin(q5))/16 - (5*3^(1/2)*dq1*dqr1*cos(2*q2)*cos(2*q5)*sin(2*q3)*sin(2*q6)*sin(q4))/64 - (3^(1/2)*dq1*dqr1*cos(2*q2)*cos(2*q6)*sin(2*q3)*sin(2*q5)*sin(q4))/16 - (5*3^(1/2)*dq1*dqr1*cos(2*q2)*sin(2*q3)*sin(2*q5)*sin(2*q6)*cos(q4))/32 + (5*3^(1/2)*dq1*dqr1*cos(2*q3)*cos(2*q5)*sin(2*q2)*sin(2*q6)*sin(q4))/64 + (3^(1/2)*dq1*dqr1*cos(2*q3)*cos(2*q6)*sin(2*q2)*sin(2*q5)*sin(q4))/16 + (5*3^(1/2)*dq1*dqr1*cos(2*q3)*sin(2*q2)*sin(2*q5)*sin(2*q6)*cos(q4))/32 + (3^(1/2)*dq2*dqr1*cos(2*q5)*cos(2*q6)*cos(q2)*cos(q3)*sin(q4))/8 + (5*3^(1/2)*dq2*dqr1*cos(2*q5)*sin(2*q6)*cos(q2)*cos(q3)*cos(q4))/64 + (3^(1/2)*dq2*dqr1*cos(2*q6)*sin(2*q5)*cos(q2)*cos(q3)*cos(q4))/16 - (3^(1/2)*dq3*dqr1*cos(2*q5)*cos(2*q6)*cos(q2)*cos(q3)*sin(q4))/8 - (5*3^(1/2)*dq3*dqr1*cos(2*q5)*sin(2*q6)*cos(q2)*cos(q3)*cos(q4))/64 - (3^(1/2)*dq3*dqr1*cos(2*q6)*sin(2*q5)*cos(q2)*cos(q3)*cos(q4))/16 - (5*3^(1/2)*dq2*dqr1*sin(2*q5)*sin(2*q6)*cos(q2)*cos(q3)*sin(q4))/32 + (5*3^(1/2)*dq3*dqr1*sin(2*q5)*sin(2*q6)*cos(q2)*cos(q3)*sin(q4))/32 - (3^(1/2)*dq1*dqr1*cos(2*q2)*cos(2*q6)*sin(2*q3)*cos(q4)*cos(q5))/8 + (3^(1/2)*dq1*dqr1*cos(2*q3)*cos(2*q6)*sin(2*q2)*cos(q4)*cos(q5))/8 - (3^(1/2)*dq1*dqr1*cos(2*q2)*cos(2*q6)*sin(2*q3)*sin(q4)*sin(q5))/8 + (3^(1/2)*dq1*dqr1*cos(2*q2)*sin(2*q3)*sin(2*q6)*cos(q4)*sin(q5))/16 - (3^(1/2)*dq1*dqr1*cos(2*q2)*sin(2*q3)*sin(2*q6)*cos(q5)*sin(q4))/16 + (3^(1/2)*dq1*dqr1*cos(2*q3)*cos(2*q6)*sin(2*q2)*sin(q4)*sin(q5))/8 - (3^(1/2)*dq1*dqr1*cos(2*q3)*sin(2*q2)*sin(2*q6)*cos(q4)*sin(q5))/16 + (3^(1/2)*dq1*dqr1*cos(2*q3)*sin(2*q2)*sin(2*q6)*cos(q5)*sin(q4))/16;
Y6_20_3=(3*dq1*dqr1*sin(2*q6))/256 - (3*dq2*dqr2*sin(2*q6))/128 - (3*dq2*dqr2*cos(2*q6)*sin(q5))/16 - (3*dq2*dqr2*sin(2*q6)*cos(q5))/32 + (3*dq3*dqr2*cos(2*q6)*sin(q5))/16 + (3*dq3*dqr2*sin(2*q6)*cos(q5))/32 - (3^(1/2)*dq4*dqr2*sin(q4))/8 + (27*dq1*dqr1*cos(2*q4)*sin(2*q6))/256 - (15*dq1*dqr1*cos(2*q5)*sin(2*q6))/256 - (3*dq1*dqr1*cos(2*q6)*sin(2*q5))/64 - (27*dq2*dqr2*cos(2*q4)*sin(2*q6))/128 + (15*dq2*dqr2*cos(2*q5)*sin(2*q6))/128 + (3*dq2*dqr2*cos(2*q6)*sin(2*q5))/32 - (3*dq3*dqr2*cos(2*q6)*sin(2*q5))/32 + (dq1*dqr2*cos(q2)*sin(q3))/8 - (dq1*dqr2*cos(q3)*sin(q2))/8 + (3^(1/2)*dq4*dqr2*cos(q4)*sin(q5))/4 + (3^(1/2)*dq4*dqr2*cos(q5)*sin(q4))/8 + (3^(1/2)*dq5*dqr2*cos(q4)*sin(q5))/8 + (3^(1/2)*dq5*dqr2*cos(q5)*sin(q4))/4 - (3*dq2*dqr2*cos(2*q4)*cos(2*q6)*sin(q5))/16 - (3*dq2*dqr2*cos(2*q4)*sin(2*q6)*cos(q5))/32 - (3*dq2*dqr2*cos(2*q6)*sin(2*q4)*cos(q5))/8 + (3*dq3*dqr2*cos(2*q4)*cos(2*q6)*sin(q5))/16 + (3*dq3*dqr2*cos(2*q4)*sin(2*q6)*cos(q5))/32 + (3*dq3*dqr2*cos(2*q6)*sin(2*q4)*cos(q5))/8 + (3*dq2*dqr2*sin(2*q4)*sin(2*q6)*sin(q5))/16 - (3*dq3*dqr2*sin(2*q4)*sin(2*q6)*sin(q5))/16 - (9*3^(1/2)*dq4*dqr2*sin(2*q6)*cos(q4))/64 - (3*3^(1/2)*dq5*dqr2*sin(2*q6)*cos(q4))/16 + (3*dq1*dqr2*cos(q2)*cos(q5)*sin(q3))/8 - (3*dq1*dqr2*cos(q3)*cos(q5)*sin(q2))/8 + (9*dq1*dqr1*cos(2*q2)*cos(2*q3)*sin(2*q6))/256 + (25*dq1*dqr1*cos(2*q4)*cos(2*q5)*sin(2*q6))/256 + (5*dq1*dqr1*cos(2*q4)*cos(2*q6)*sin(2*q5))/64 - (25*dq2*dqr2*cos(2*q4)*cos(2*q5)*sin(2*q6))/128 - (5*dq2*dqr2*cos(2*q4)*cos(2*q6)*sin(2*q5))/32 - (dq2*dqr2*cos(2*q5)*cos(2*q6)*sin(2*q4))/8 + (5*dq3*dqr2*cos(2*q4)*cos(2*q6)*sin(2*q5))/32 + (dq3*dqr2*cos(2*q5)*cos(2*q6)*sin(2*q4))/8 + (5*dq2*dqr2*sin(2*q4)*sin(2*q5)*sin(2*q6))/32 - (5*dq3*dqr2*sin(2*q4)*sin(2*q5)*sin(2*q6))/32 - (27*dq1*dqr1*cos(2*q2)*cos(2*q3)*cos(2*q4)*sin(2*q6))/256 - (45*dq1*dqr1*cos(2*q2)*cos(2*q3)*cos(2*q5)*sin(2*q6))/256 - (9*dq1*dqr1*cos(2*q2)*cos(2*q3)*cos(2*q6)*sin(2*q5))/64 + (3^(1/2)*dq1*dqr2*cos(q2)*cos(q3)*sin(q4))/8 + (3^(1/2)*dq1*dqr2*sin(q2)*sin(q3)*sin(q4))/8 + (27*dq1*dqr2*sin(2*q4)*sin(2*q6)*cos(q2)*sin(q3))/128 - (27*dq1*dqr2*sin(2*q4)*sin(2*q6)*cos(q3)*sin(q2))/128 + (3^(1/2)*dq4*dqr2*cos(2*q6)*cos(q4)*sin(q5))/8 - (3^(1/2)*dq4*dqr2*cos(2*q6)*cos(q5)*sin(q4))/8 + (3^(1/2)*dq4*dqr2*sin(2*q6)*cos(q4)*cos(q5))/16 - (3^(1/2)*dq5*dqr2*cos(2*q6)*cos(q4)*sin(q5))/8 - (3^(1/2)*dq5*dqr2*cos(2*q6)*cos(q5)*sin(q4))/4 - (3^(1/2)*dq5*dqr2*sin(2*q6)*cos(q4)*cos(q5))/16 + (3^(1/2)*dq4*dqr2*sin(2*q6)*sin(q4)*sin(q5))/16 + (3^(1/2)*dq5*dqr2*sin(2*q6)*sin(q4)*sin(q5))/8 + (3^(1/2)*dq4*dqr2*cos(2*q5)*cos(2*q6)*sin(q4))/8 + (5*3^(1/2)*dq4*dqr2*cos(2*q5)*sin(2*q6)*cos(q4))/64 + (3^(1/2)*dq4*dqr2*cos(2*q6)*sin(2*q5)*cos(q4))/16 - (5*3^(1/2)*dq4*dqr2*sin(2*q5)*sin(2*q6)*sin(q4))/32 - (3^(1/2)*dq1*dqr2*cos(q4)*sin(q2)*sin(q3)*sin(q5))/4 - (3^(1/2)*dq1*dqr2*cos(q5)*sin(q2)*sin(q3)*sin(q4))/8 - (3*dq1*dqr2*cos(2*q4)*cos(2*q6)*cos(q2)*cos(q5)*sin(q3))/8 + (3*dq1*dqr2*cos(2*q4)*cos(2*q6)*cos(q3)*cos(q5)*sin(q2))/8 - (25*dq1*dqr1*cos(2*q2)*cos(2*q3)*cos(2*q4)*cos(2*q5)*sin(2*q6))/256 + (3*dq1*dqr2*cos(2*q4)*sin(2*q6)*cos(q2)*sin(q3)*sin(q5))/16 - (3*dq1*dqr2*cos(2*q4)*sin(2*q6)*cos(q3)*sin(q2)*sin(q5))/16 + (3*dq1*dqr2*cos(2*q6)*sin(2*q4)*cos(q2)*sin(q3)*sin(q5))/16 - (3*dq1*dqr2*cos(2*q6)*sin(2*q4)*cos(q3)*sin(q2)*sin(q5))/16 + (3*dq1*dqr2*sin(2*q4)*sin(2*q6)*cos(q2)*cos(q5)*sin(q3))/32 - (3*dq1*dqr2*sin(2*q4)*sin(2*q6)*cos(q3)*cos(q5)*sin(q2))/32 - (9*3^(1/2)*dq1*dqr2*sin(2*q6)*cos(q2)*cos(q3)*cos(q4))/64 - (9*3^(1/2)*dq1*dqr2*sin(2*q6)*cos(q4)*sin(q2)*sin(q3))/64 - (dq1*dqr2*cos(2*q4)*cos(2*q5)*cos(2*q6)*cos(q2)*sin(q3))/8 + (dq1*dqr2*cos(2*q4)*cos(2*q5)*cos(2*q6)*cos(q3)*sin(q2))/8 + (5*dq1*dqr2*cos(2*q4)*sin(2*q5)*sin(2*q6)*cos(q2)*sin(q3))/32 - (5*dq1*dqr2*cos(2*q4)*sin(2*q5)*sin(2*q6)*cos(q3)*sin(q2))/32 + (25*dq1*dqr2*cos(2*q5)*sin(2*q4)*sin(2*q6)*cos(q2)*sin(q3))/128 - (25*dq1*dqr2*cos(2*q5)*sin(2*q4)*sin(2*q6)*cos(q3)*sin(q2))/128 + (5*dq1*dqr2*cos(2*q6)*sin(2*q4)*sin(2*q5)*cos(q2)*sin(q3))/32 - (5*dq1*dqr2*cos(2*q6)*sin(2*q4)*sin(2*q5)*cos(q3)*sin(q2))/32 - (3^(1/2)*dq1*dqr2*cos(q2)*cos(q3)*cos(q4)*sin(q5))/4 - (3^(1/2)*dq1*dqr2*cos(q2)*cos(q3)*cos(q5)*sin(q4))/8 + (3^(1/2)*dq1*dqr2*cos(2*q6)*cos(q2)*cos(q3)*cos(q4)*sin(q5))/8 - (3^(1/2)*dq1*dqr2*cos(2*q6)*cos(q2)*cos(q3)*cos(q5)*sin(q4))/8 + (3^(1/2)*dq1*dqr2*sin(2*q6)*cos(q2)*cos(q3)*cos(q4)*cos(q5))/16 + (3^(1/2)*dq1*dqr2*cos(2*q6)*cos(q4)*sin(q2)*sin(q3)*sin(q5))/8 - (3^(1/2)*dq1*dqr2*cos(2*q6)*cos(q5)*sin(q2)*sin(q3)*sin(q4))/8 + (3^(1/2)*dq1*dqr2*sin(2*q6)*cos(q2)*cos(q3)*sin(q4)*sin(q5))/16 + (3^(1/2)*dq1*dqr2*sin(2*q6)*cos(q4)*cos(q5)*sin(q2)*sin(q3))/16 + (3^(1/2)*dq1*dqr2*sin(2*q6)*sin(q2)*sin(q3)*sin(q4)*sin(q5))/16 + (3^(1/2)*dq1*dqr2*cos(2*q5)*cos(2*q6)*cos(q2)*cos(q3)*sin(q4))/8 + (5*3^(1/2)*dq1*dqr2*cos(2*q5)*sin(2*q6)*cos(q2)*cos(q3)*cos(q4))/64 + (3^(1/2)*dq1*dqr2*cos(2*q6)*sin(2*q5)*cos(q2)*cos(q3)*cos(q4))/16 + (3^(1/2)*dq1*dqr2*cos(2*q5)*cos(2*q6)*sin(q2)*sin(q3)*sin(q4))/8 + (5*3^(1/2)*dq1*dqr2*cos(2*q5)*sin(2*q6)*cos(q4)*sin(q2)*sin(q3))/64 + (3^(1/2)*dq1*dqr2*cos(2*q6)*sin(2*q5)*cos(q4)*sin(q2)*sin(q3))/16 - (5*3^(1/2)*dq1*dqr2*sin(2*q5)*sin(2*q6)*cos(q2)*cos(q3)*sin(q4))/32 - (5*3^(1/2)*dq1*dqr2*sin(2*q5)*sin(2*q6)*sin(q2)*sin(q3)*sin(q4))/32;
